simulink model "DYN_03x"  (R2021a)
(part 6 of 9)

C315 = + 1.5*a3*de5*m6*y6*cos(e2)*cos(e3)*sin(e4)*sin(e5)*sin(e6) + 1.5*a3*de6*m6*y6*cos(e5)*cos(e6)*sin(e2)*sin(e3)*sin(e4) + 0.5*d4*de2*m6*x6*cos(e5)*cos(e6)*sin(e2)*sin(e3)*sin(e4) + 0.5*d4*de3*m6*x6*cos(e5)*cos(e6)*sin(e2)*sin(e3)*sin(e4) + 1.5*d4*de5*m6*x6*cos(e2)*cos(e6)*sin(e3)*sin(e4)*sin(e5) + 1.5*d4*de5*m6*x6*cos(e3)*cos(e6)*sin(e2)*sin(e4)*sin(e5) + 1.5*d4*de6*m6*x6*cos(e2)*cos(e5)*sin(e3)*sin(e4)*sin(e6) + 1.5*d4*de6*m6*x6*cos(e3)*cos(e5)*sin(e2)*sin(e4)*sin(e6) - 2.0*I6xx*de5*cos(e4)*cos(e5)*cos(e6)^2*sin(e2)*sin(e3)*sin(e4)*sin(e5) - 2.0*I6xx*de6*cos(e4)*cos(e5)^2*cos(e6)*sin(e2)*sin(e3)*sin(e4)*sin(e6) + 2.0*I6yy*de5*cos(e4)*cos(e5)*cos(e6)^2*sin(e2)*sin(e3)*sin(e4)*sin(e5) + 2.0*I6yy*de6*cos(e4)*cos(e5)^2*cos(e6)*sin(e2)*sin(e3)*sin(e4)*sin(e6) - 4.0*d4*de1*m4*y4*cos(e2)*cos(e3)*sin(e2)*sin(e3)*sin(e4) + 4.0*d4*de1*m5*z5*cos(e2)*cos(e3)*sin(e2)*sin(e3)*sin(e4) - 8.0*de1*m6*x6*z6*cos(e2)^2*cos(e3)^2*cos(e4)*cos(e5)^2*cos(e6) - 4.0*de1*m5*x5*y5*cos(e2)*cos(e3)*cos(e4)*sin(e2)*sin(e3) + 2.0*de1*m6*x6*y6*cos(e2)*cos(e4)*cos(e5)*sin(e2)*sin(e4) + 2.0*de1*m6*x6*y6*cos(e3)*cos(e4)*cos(e5)*sin(e3)*sin(e4) + 2.0*de1*m6*x6*y6*cos(e4)*cos(e5)*cos(e6)*sin(e5)*sin(e6) + 4.0*de1*m4*x4*z4*cos(e2)*cos(e3)*cos(e4)*sin(e2)*sin(e3) + 2.0*de1*m5*x5*z5*cos(e2)*cos(e4)*cos(e5)*sin(e2)*sin(e4) + 2.0*de1*m5*x5*z5*cos(e3)*cos(e4)*cos(e5)*sin(e3)*sin(e4) - 2.0*de1*m6*x6*z6*cos(e2)*cos(e5)*cos(e6)*sin(e2)*sin(e5) - 2.0*de1*m6*x6*z6*cos(e3)*cos(e5)*cos(e6)*sin(e3)*sin(e5) - 4.0*de4*m5*y5*z5*cos(e2)*cos(e3)*cos(e4)*sin(e4)*sin(e5) + 0.5*de2*m6*y6*z6*cos(e4)*cos(e5)*cos(e6)*sin(e2)*sin(e3) + 0.5*de3*m6*y6*z6*cos(e4)*cos(e5)*cos(e6)*sin(e2)*sin(e3) + 1.5*de4*m6*y6*z6*cos(e2)*cos(e5)*cos(e6)*sin(e3)*sin(e4) + 1.5*de4*m6*y6*z6*cos(e3)*cos(e5)*cos(e6)*sin(e2)*sin(e4) - 2.0*de5*m6*y6*z6*cos(e2)*cos(e3)*cos(e4)*sin(e4)*sin(e6) - 1.0*de4*m6*y6*z6*cos(e2)*cos(e3)*cos(e5)*sin(e5)*sin(e6) + 0.5*de5*m6*y6*z6*cos(e2)*cos(e4)*cos(e6)*sin(e3)*sin(e5) + 0.5*de5*m6*y6*z6*cos(e3)*cos(e4)*cos(e6)*sin(e2)*sin(e5) + 1.5*de6*m6*y6*z6*cos(e2)*cos(e4)*cos(e5)*sin(e3)*sin(e6) + 1.5*de6*m6*y6*z6*cos(e3)*cos(e4)*cos(e5)*sin(e2)*sin(e6) + 1.5*a3*de5*m6*x6*cos(e6)*sin(e2)*sin(e3)*sin(e4)*sin(e5) + 1.5*a3*de6*m6*x6*cos(e5)*sin(e2)*sin(e3)*sin(e4)*sin(e6) - 1.0*a2*de1*m6*y6*cos(e2)*sin(e2)*sin(e3)*sin(e5)*sin(e6) - 0.5*d4*de2*m6*y6*cos(e5)*sin(e2)*sin(e3)*sin(e4)*sin(e6) - 0.5*d4*de3*m6*y6*cos(e5)*sin(e2)*sin(e3)*sin(e4)*sin(e6) - 1.5*d4*de5*m6*y6*cos(e2)*sin(e3)*sin(e4)*sin(e5)*sin(e6) - 1.5*d4*de5*m6*y6*cos(e3)*sin(e2)*sin(e4)*sin(e5)*sin(e6) - 0.5*de2*m6*x6^2*cos(e2)*cos(e3)*cos(e5)*cos(e6)^2*sin(e4)*sin(e5) - 1.0*de2*m6*x6^2*cos(e2)*cos(e4)^2*cos(e5)*cos(e6)*sin(e3)*sin(e6) - 1.0*de2*m6*x6^2*cos(e3)*cos(e4)^2*cos(e5)*cos(e6)*sin(e2)*sin(e6) - 0.5*de3*m6*x6^2*cos(e2)*cos(e3)*cos(e5)*cos(e6)^2*sin(e4)*sin(e5) - 1.0*de3*m6*x6^2*cos(e2)*cos(e4)^2*cos(e5)*cos(e6)*sin(e3)*sin(e6) - 1.0*de3*m6*x6^2*cos(e3)*cos(e4)^2*cos(e5)*cos(e6)*sin(e2)*sin(e6) - 1.5*de4*m6*x6^2*cos(e2)*cos(e4)*cos(e5)*cos(e6)^2*sin(e3)*sin(e5) - 1.5*de4*m6*x6^2*cos(e3)*cos(e4)*cos(e5)*cos(e6)^2*sin(e2)*sin(e5) - 2.0*de5*m6*x6^2*cos(e2)*cos(e3)*cos(e4)^2*cos(e6)*sin(e5)*sin(e6) + 0.5*de2*m6*y6^2*cos(e2)*cos(e3)*cos(e5)*cos(e6)^2*sin(e4)*sin(e5) + de2*m6*y6^2*cos(e2)*cos(e4)^2*cos(e5)*cos(e6)*sin(e3)*sin(e6) + de2*m6*y6^2*cos(e3)*cos(e4)^2*cos(e5)*cos(e6)*sin(e2)*sin(e6) + 0.5*de3*m6*y6^2*cos(e2)*cos(e3)*cos(e5)*cos(e6)^2*sin(e4)*sin(e5) + de3*m6*y6^2*cos(e2)*cos(e4)^2*cos(e5)*cos(e6)*sin(e3)*sin(e6) + de3*m6*y6^2*cos(e3)*cos(e4)^2*cos(e5)*cos(e6)*sin(e2)*sin(e6) + 1.5*de4*m6*y6^2*cos(e2)*cos(e4)*cos(e5)*cos(e6)^2*sin(e3)*sin(e5) + 1.5*de4*m6*y6^2*cos(e3)*cos(e4)*cos(e5)*cos(e6)^2*sin(e2)*sin(e5) + 2.0*de5*m6*y6^2*cos(e2)*cos(e3)*cos(e4)^2*cos(e6)*sin(e5)*sin(e6) + 4.0*de5*m5*x5*y5*cos(e2)*cos(e5)*sin(e3)*sin(e4)*sin(e5) + 4.0*de5*m5*x5*y5*cos(e3)*cos(e5)*sin(e2)*sin(e4)*sin(e5) - 4.0*de4*m6*x6*y6*cos(e4)*cos(e5)*sin(e2)*sin(e3)*sin(e4) - 2.0*de6*m6*x6*y6*cos(e2)*cos(e5)*sin(e3)*sin(e4)*sin(e5) - 2.0*de6*m6*x6*y6*cos(e3)*cos(e5)*sin(e2)*sin(e4)*sin(e5) - 3.0*de5*m6*x6*y6*cos(e2)*cos(e6)*sin(e3)*sin(e4)*sin(e6) - 3.0*de5*m6*x6*y6*cos(e3)*cos(e6)*sin(e2)*sin(e4)*sin(e6) - 4.0*de6*m6*x6*y6*cos(e5)*cos(e6)*sin(e2)*sin(e3)*sin(e6) + 8.0*de1*m6*y6*z6*cos(e2)^2*cos(e3)^2*cos(e4)*cos(e5)^2*sin(e6) - 4.0*de4*m5*x5*z5*cos(e4)*cos(e5)*sin(e2)*sin(e3)*sin(e4) + 0.5*de2*m6*x6*z6*cos(e4)*cos(e5)*sin(e2)*sin(e3)*sin(e6) + 0.5*de3*m6*x6*z6*cos(e4)*cos(e5)*sin(e2)*sin(e3)*sin(e6) + 1.5*de4*m6*x6*z6*cos(e2)*cos(e5)*sin(e3)*sin(e4)*sin(e6) + 1.5*de4*m6*x6*z6*cos(e3)*cos(e5)*sin(e2)*sin(e4)*sin(e6) - 2.0*de5*m6*x6*z6*cos(e4)*cos(e6)*sin(e2)*sin(e3)*sin(e4) - 1.0*de4*m6*x6*z6*cos(e5)*cos(e6)*sin(e2)*sin(e3)*sin(e5) + 0.5*de5*m6*x6*z6*cos(e2)*cos(e4)*sin(e3)*sin(e5)*sin(e6) + 0.5*de5*m6*x6*z6*cos(e3)*cos(e4)*sin(e2)*sin(e5)*sin(e6) - 4.0*de1*m4*y4*z4*cos(e2)*cos(e3)*sin(e2)*sin(e3)*sin(e4) - 2.0*de1*m5*y5*z5*cos(e2)*cos(e4)*sin(e2)*sin(e4)*sin(e5) - 2.0*de1*m5*y5*z5*cos(e3)*cos(e4)*sin(e3)*sin(e4)*sin(e5) + 2.0*de1*m6*y6*z6*cos(e2)*cos(e5)*sin(e2)*sin(e5)*sin(e6) + 2.0*de1*m6*y6*z6*cos(e3)*cos(e5)*sin(e3)*sin(e5)*sin(e6) - 1.5*a3*de5*m6*y6*sin(e2)*sin(e3)*sin(e4)*sin(e5)*sin(e6) - 2.0*de1*m6*x6^2*cos(e2)*cos(e3)^2*cos(e4)^2*cos(e5)^2*cos(e6)^2*sin(e2) - 2.0*de1*m6*x6^2*cos(e2)^2*cos(e3)*cos(e4)^2*cos(e5)^2*cos(e6)^2*sin(e3) + 2.0*de1*m6*y6^2*cos(e2)*cos(e3)^2*cos(e4)^2*cos(e5)^2*cos(e6)^2*sin(e2) + 2.0*de1*m6*y6^2*cos(e2)^2*cos(e3)*cos(e4)^2*cos(e5)^2*cos(e6)^2*sin(e3) + 8.0*de1*m6*x6*y6*cos(e2)^2*cos(e3)^2*cos(e6)^2*sin(e4)*sin(e5) + 4.0*de4*m5*y5*z5*cos(e4)*sin(e2)*sin(e3)*sin(e4)*sin(e5) + 2.0*de5*m6*y6*z6*cos(e4)*sin(e2)*sin(e3)*sin(e4)*sin(e6) + de4*m6*y6*z6*cos(e5)*sin(e2)*sin(e3)*sin(e5)*sin(e6) + 0.5*de2*m6*x6^2*cos(e5)*cos(e6)^2*sin(e2)*sin(e3)*sin(e4)*sin(e5) + 0.5*de3*m6*x6^2*cos(e5)*cos(e6)^2*sin(e2)*sin(e3)*sin(e4)*sin(e5) + 2.0*de5*m6*x6^2*cos(e4)^2*cos(e6)*sin(e2)*sin(e3)*sin(e5)*sin(e6) - 0.5*de2*m6*y6^2*cos(e5)*cos(e6)^2*sin(e2)*sin(e3)*sin(e4)*sin(e5) - 0.5*de3*m6*y6^2*cos(e5)*cos(e6)^2*sin(e2)*sin(e3)*sin(e4)*sin(e5) - 2.0*de5*m6*y6^2*cos(e4)^2*cos(e6)*sin(e2)*sin(e3)*sin(e5)*sin(e6) - 4.0*a3*de1*m5*x5*cos(e2)*cos(e3)^2*cos(e4)*cos(e5)*sin(e2) - 4.0*a3*de1*m5*x5*cos(e2)^2*cos(e3)*cos(e4)*cos(e5)*sin(e3) - 1.0*a2*de1*m6*x6*cos(e2)^2*cos(e4)*cos(e5)*cos(e6)*sin(e3) - 2.0*de5*m6*y6*z6*cos(e2)*cos(e3)*cos(e4)^2*cos(e5)*cos(e6) + 4.0*a3*de1*m5*y5*cos(e2)*cos(e3)^2*cos(e4)*sin(e2)*sin(e5) + 4.0*a3*de1*m5*y5*cos(e2)^2*cos(e3)*cos(e4)*sin(e3)*sin(e5) + 4.0*a3*de1*m6*y6*cos(e2)*cos(e3)^2*cos(e6)*sin(e2)*sin(e4) + 4.0*a3*de1*m6*y6*cos(e2)^2*cos(e3)*cos(e6)*sin(e3)*sin(e4) + a2*de1*m6*y6*cos(e2)^2*cos(e4)*cos(e5)*sin(e3)*sin(e6) + 4.0*a3*de1*m6*z6*cos(e2)*cos(e3)^2*cos(e4)*sin(e2)*sin(e5) + 4.0*a3*de1*m6*z6*cos(e2)^2*cos(e3)*cos(e4)*sin(e3)*sin(e5) + 4.0*d4*de1*m6*x6*cos(e2)*cos(e3)^2*cos(e6)*sin(e2)*sin(e5) + 4.0*d4*de1*m6*x6*cos(e2)^2*cos(e3)*cos(e6)*sin(e3)*sin(e5) - 4.0*de4*m5*x5*y5*cos(e2)*cos(e3)*cos(e4)^2*cos(e5)*sin(e5) - 4.0*de5*m5*x5*y5*cos(e2)*cos(e3)*cos(e4)*cos(e5)^2*sin(e4) - 1.0*de2*m6*x6*y6*cos(e2)*cos(e3)*cos(e4)*cos(e6)^2*sin(e5) - 1.0*de3*m6*x6*y6*cos(e2)*cos(e3)*cos(e4)*cos(e6)^2*sin(e5) + 2.0*de6*m6*x6*y6*cos(e2)*cos(e3)*cos(e4)*cos(e5)^2*sin(e4) - 4.0*de4*m6*x6*y6*cos(e2)*cos(e3)*cos(e4)^2*cos(e6)*sin(e6) - 1.0*de5*m6*x6*y6*cos(e2)*cos(e4)*cos(e5)*cos(e6)^2*sin(e3) - 1.0*de5*m6*x6*y6*cos(e3)*cos(e4)*cos(e5)*cos(e6)^2*sin(e2) - 4.0*de6*m6*x6*y6*cos(e2)*cos(e3)*cos(e4)*cos(e6)^2*sin(e4) + de4*m6*x6*y6*cos(e2)*cos(e3)*cos(e5)^2*cos(e6)*sin(e6) - 1.0*de2*m6*x6*z6*cos(e2)*cos(e3)*cos(e5)^2*cos(e6)*sin(e4) - 1.0*de3*m6*x6*z6*cos(e2)*cos(e3)*cos(e5)^2*cos(e6)*sin(e4) - 3.0*de4*m6*x6*z6*cos(e2)*cos(e4)*cos(e5)^2*cos(e6)*sin(e3) - 3.0*de4*m6*x6*z6*cos(e3)*cos(e4)*cos(e5)^2*cos(e6)*sin(e2) - 2.0*de5*m6*x6*z6*cos(e2)*cos(e3)*cos(e4)^2*cos(e5)*sin(e6) - 2.0*de6*m6*x6*z6*cos(e2)*cos(e3)*cos(e4)^2*cos(e6)*sin(e5) + 4.0*a3*de1*m6*x6*cos(e2)*cos(e3)^2*sin(e2)*sin(e4)*sin(e6) + 4.0*a3*de1*m6*x6*cos(e2)^2*cos(e3)*sin(e3)*sin(e4)*sin(e6) - 4.0*d4*de1*m6*y6*cos(e2)*cos(e3)^2*sin(e2)*sin(e5)*sin(e6) - 4.0*d4*de1*m6*y6*cos(e2)^2*cos(e3)*sin(e3)*sin(e5)*sin(e6) + 4.0*de1*m4*x4*y4*cos(e2)*cos(e3)^2*cos(e4)*sin(e2)*sin(e4) + 4.0*de1*m4*x4*y4*cos(e2)^2*cos(e3)*cos(e4)*sin(e3)*sin(e4) + 4.0*de1*m5*x5*y5*cos(e2)*cos(e3)^2*cos(e5)*sin(e2)*sin(e5) - 2.0*de1*m5*x5*y5*cos(e2)*cos(e4)^2*cos(e5)*sin(e2)*sin(e5) + 4.0*de1*m5*x5*y5*cos(e2)^2*cos(e3)*cos(e5)*sin(e3)*sin(e5) - 2.0*de1*m5*x5*y5*cos(e3)*cos(e4)^2*cos(e5)*sin(e3)*sin(e5) - 8.0*de1*m6*x6*y6*cos(e2)*cos(e3)^2*cos(e6)*sin(e2)*sin(e6) - 2.0*de1*m6*x6*y6*cos(e2)*cos(e4)^2*cos(e6)*sin(e2)*sin(e6) - 8.0*de1*m6*x6*y6*cos(e2)^2*cos(e3)*cos(e6)*sin(e3)*sin(e6) - 2.0*de1*m6*x6*y6*cos(e2)*cos(e5)^2*cos(e6)*sin(e2)*sin(e6) - 2.0*de1*m6*x6*y6*cos(e3)*cos(e4)^2*cos(e6)*sin(e3)*sin(e6) - 2.0*de1*m6*x6*y6*cos(e3)*cos(e5)^2*cos(e6)*sin(e3)*sin(e6) + de2*m6*y6*z6*cos(e2)*cos(e3)*cos(e5)^2*sin(e4)*sin(e6) + de2*m6*y6*z6*cos(e2)*cos(e4)^2*cos(e6)*sin(e3)*sin(e5) + de2*m6*y6*z6*cos(e3)*cos(e4)^2*cos(e6)*sin(e2)*sin(e5) + de3*m6*y6*z6*cos(e2)*cos(e3)*cos(e5)^2*sin(e4)*sin(e6) + de3*m6*y6*z6*cos(e2)*cos(e4)^2*cos(e6)*sin(e3)*sin(e5) + de3*m6*y6*z6*cos(e3)*cos(e4)^2*cos(e6)*sin(e2)*sin(e5) + 3.0*de4*m6*y6*z6*cos(e2)*cos(e4)*cos(e5)^2*sin(e3)*sin(e6) + 3.0*de4*m6*y6*z6*cos(e3)*cos(e4)*cos(e5)^2*sin(e2)*sin(e6) + 2.0*de5*m6*y6*z6*cos(e4)^2*cos(e5)*cos(e6)*sin(e2)*sin(e3) + 2.0*de6*m6*y6*z6*cos(e2)*cos(e3)*cos(e4)^2*sin(e5)*sin(e6) + 2.0*de6*m6*y6*z6*cos(e2)*cos(e5)^2*cos(e6)*sin(e3)*sin(e4) + 2.0*de6*m6*y6*z6*cos(e3)*cos(e5)^2*cos(e6)*sin(e2)*sin(e4) - 0.5*de2*m6*x6^2*cos(e2)*cos(e4)*cos(e5)^2*cos(e6)^2*sin(e3)*sin(e4) - 0.5*de2*m6*x6^2*cos(e3)*cos(e4)*cos(e5)^2*cos(e6)^2*sin(e2)*sin(e4) - 0.5*de3*m6*x6^2*cos(e2)*cos(e4)*cos(e5)^2*cos(e6)^2*sin(e3)*sin(e4) - 0.5*de3*m6*x6^2*cos(e3)*cos(e4)*cos(e5)^2*cos(e6)^2*sin(e2)*sin(e4) + 0.5*de2*m6*y6^2*cos(e2)*cos(e4)*cos(e5)^2*cos(e6)^2*sin(e3)*sin(e4) + 0.5*de2*m6*y6^2*cos(e3)*cos(e4)*cos(e5)^2*cos(e6)^2*sin(e2)*sin(e4) + 0.5*de3*m6*y6^2*cos(e2)*cos(e4)*cos(e5)^2*cos(e6)^2*sin(e3)*sin(e4) + 0.5*de3*m6*y6^2*cos(e3)*cos(e4)*cos(e5)^2*cos(e6)^2*sin(e2)*sin(e4) + 4.0*de4*m5*x5*y5*cos(e4)^2*cos(e5)*sin(e2)*sin(e3)*sin(e5) + 4.0*de5*m5*x5*y5*cos(e4)*cos(e5)^2*sin(e2)*sin(e3)*sin(e4) + de2*m6*x6*y6*cos(e4)*cos(e6)^2*sin(e2)*sin(e3)*sin(e5) + de3*m6*x6*y6*cos(e4)*cos(e6)^2*sin(e2)*sin(e3)*sin(e5) + 3.0*de4*m6*x6*y6*cos(e2)*cos(e6)^2*sin(e3)*sin(e4)*sin(e5) + 3.0*de4*m6*x6*y6*cos(e3)*cos(e6)^2*sin(e2)*sin(e4)*sin(e5) - 2.0*de6*m6*x6*y6*cos(e4)*cos(e5)^2*sin(e2)*sin(e3)*sin(e4) + 4.0*de4*m6*x6*y6*cos(e4)^2*cos(e6)*sin(e2)*sin(e3)*sin(e6) + 4.0*de6*m6*x6*y6*cos(e4)*cos(e6)^2*sin(e2)*sin(e3)*sin(e4) - 1.0*de4*m6*x6*y6*cos(e5)^2*cos(e6)*sin(e2)*sin(e3)*sin(e6) + de2*m6*x6*z6*cos(e2)*cos(e4)^2*sin(e3)*sin(e5)*sin(e6) + de2*m6*x6*z6*cos(e3)*cos(e4)^2*sin(e2)*sin(e5)*sin(e6) + de2*m6*x6*z6*cos(e5)^2*cos(e6)*sin(e2)*sin(e3)*sin(e4) + de3*m6*x6*z6*cos(e2)*cos(e4)^2*sin(e3)*sin(e5)*sin(e6) + de3*m6*x6*z6*cos(e3)*cos(e4)^2*sin(e2)*sin(e5)*sin(e6) + de3*m6*x6*z6*cos(e5)^2*cos(e6)*sin(e2)*sin(e3)*sin(e4) + 2.0*de5*m6*x6*z6*cos(e4)^2*cos(e5)*sin(e2)*sin(e3)*sin(e6) + 2.0*de6*m6*x6*z6*cos(e2)*cos(e5)^2*sin(e3)*sin(e4)*sin(e6) + 2.0*de6*m6*x6*z6*cos(e3)*cos(e5)^2*sin(e2)*sin(e4)*sin(e6) + 2.0*de6*m6*x6*z6*cos(e4)^2*cos(e6)*sin(e2)*sin(e3)*sin(e5) + 4.0*I6xx*de4*cos(e2)*cos(e3)*cos(e4)*cos(e5)*cos(e6)*sin(e4)*sin(e6) - 4.0*I6yy*de4*cos(e2)*cos(e3)*cos(e4)*cos(e5)*cos(e6)*sin(e4)*sin(e6) + 4.0*de1*m6*x6^2*cos(e2)^2*cos(e3)^2*cos(e6)*sin(e4)*sin(e5)*sin(e6) - 4.0*de1*m6*y6^2*cos(e2)^2*cos(e3)^2*cos(e6)*sin(e4)*sin(e5)*sin(e6) - 1.0*de2*m6*y6*z6*cos(e5)^2*sin(e2)*sin(e3)*sin(e4)*sin(e6) - 1.0*de3*m6*y6*z6*cos(e5)^2*sin(e2)*sin(e3)*sin(e4)*sin(e6) - 2.0*de6*m6*y6*z6*cos(e4)^2*sin(e2)*sin(e3)*sin(e5)*sin(e6) - 4.0*d4*de1*m6*x6*cos(e2)^2*cos(e3)^2*cos(e4)*cos(e5)*cos(e6) - 4.0*I5xx*de1*cos(e2)*cos(e3)*cos(e4)*cos(e5)*sin(e2)*sin(e3)*sin(e5) + 2.0*I6xx*de1*cos(e2)*cos(e4)*cos(e5)*cos(e6)*sin(e2)*sin(e4)*sin(e6) + 2.0*I6xx*de1*cos(e3)*cos(e4)*cos(e5)*cos(e6)*sin(e3)*sin(e4)*sin(e6) + 4.0*I5yy*de1*cos(e2)*cos(e3)*cos(e4)*cos(e5)*sin(e2)*sin(e3)*sin(e5) - 4.0*I6yy*de1*cos(e2)*cos(e3)*cos(e4)*cos(e5)*sin(e2)*sin(e3)*sin(e5) - 2.0*I6yy*de1*cos(e2)*cos(e4)*cos(e5)*cos(e6)*sin(e2)*sin(e4)*sin(e6) - 2.0*I6yy*de1*cos(e3)*cos(e4)*cos(e5)*cos(e6)*sin(e3)*sin(e4)*sin(e6) + 4.0*I6zz*de1*cos(e2)*cos(e3)*cos(e4)*cos(e5)*sin(e2)*sin(e3)*sin(e5) + 4.0*d4*de1*m6*y6*cos(e2)^2*cos(e3)^2*cos(e4)*cos(e5)*sin(e6) - 4.0*I6xx*de4*cos(e4)*cos(e5)*cos(e6)*sin(e2)*sin(e3)*sin(e4)*sin(e6) - 2.0*I6xx*de6*cos(e2)*cos(e5)*cos(e6)*sin(e3)*sin(e4)*sin(e5)*sin(e6) - 2.0*I6xx*de6*cos(e3)*cos(e5)*cos(e6)*sin(e2)*sin(e4)*sin(e5)*sin(e6) + 4.0*I6yy*de4*cos(e4)*cos(e5)*cos(e6)*sin(e2)*sin(e3)*sin(e4)*sin(e6) + 2.0*I6yy*de6*cos(e2)*cos(e5)*cos(e6)*sin(e3)*sin(e4)*sin(e5)*sin(e6) + 2.0*I6yy*de6*cos(e3)*cos(e5)*cos(e6)*sin(e2)*sin(e4)*sin(e5)*sin(e6) - 2.0*de5*m5*x5^2*cos(e2)*cos(e3)*cos(e4)*cos(e5)*sin(e4)*sin(e5) - 0.5*de2*m6*x6^2*cos(e2)*cos(e3)*cos(e4)*cos(e6)*sin(e5)*sin(e6) - 0.5*de3*m6*x6^2*cos(e2)*cos(e3)*cos(e4)*cos(e6)*sin(e5)*sin(e6) - 0.5*de5*m6*x6^2*cos(e2)*cos(e4)*cos(e5)*cos(e6)*sin(e3)*sin(e6) - 0.5*de5*m6*x6^2*cos(e3)*cos(e4)*cos(e5)*cos(e6)*sin(e2)*sin(e6) - 2.0*de6*m6*x6^2*cos(e2)*cos(e3)*cos(e4)*cos(e6)*sin(e4)*sin(e6) - 2.0*de2*m6*x6*y6*cos(e2)*cos(e4)^2*cos(e5)*cos(e6)^2*sin(e3) - 2.0*de2*m6*x6*y6*cos(e3)*cos(e4)^2*cos(e5)*cos(e6)^2*sin(e2) - 2.0*de3*m6*x6*y6*cos(e2)*cos(e4)^2*cos(e5)*cos(e6)^2*sin(e3) - 2.0*de3*m6*x6*y6*cos(e3)*cos(e4)^2*cos(e5)*cos(e6)^2*sin(e2) - 4.0*de5*m6*x6*y6*cos(e2)*cos(e3)*cos(e4)^2*cos(e6)^2*sin(e5) + 2.0*de5*m5*y5^2*cos(e2)*cos(e3)*cos(e4)*cos(e5)*sin(e4)*sin(e5) + 0.5*de2*m6*y6^2*cos(e2)*cos(e3)*cos(e4)*cos(e6)*sin(e5)*sin(e6) - 2.0*de5*m6*y6^2*cos(e2)*cos(e3)*cos(e4)*cos(e5)*sin(e4)*sin(e5) + 0.5*de3*m6*y6^2*cos(e2)*cos(e3)*cos(e4)*cos(e6)*sin(e5)*sin(e6) + 0.5*de5*m6*y6^2*cos(e2)*cos(e4)*cos(e5)*cos(e6)*sin(e3)*sin(e6) + 0.5*de5*m6*y6^2*cos(e3)*cos(e4)*cos(e5)*cos(e6)*sin(e2)*sin(e6) + 2.0*de6*m6*y6^2*cos(e2)*cos(e3)*cos(e4)*cos(e6)*sin(e4)*sin(e6) + 2.0*de5*m6*z6^2*cos(e2)*cos(e3)*cos(e4)*cos(e5)*sin(e4)*sin(e5) + 4.0*de1*m6*y6*z6*cos(e2)^2*cos(e3)^2*cos(e5)*cos(e6)*sin(e4) - 4.0*de1*m6*x6^2*cos(e2)^2*cos(e3)^2*cos(e4)*cos(e5)*cos(e6)^2*sin(e5) + 4.0*de1*m6*y6^2*cos(e2)^2*cos(e3)^2*cos(e4)*cos(e5)*cos(e6)^2*sin(e5) + 4.0*de1*m6*x6*z6*cos(e2)^2*cos(e3)^2*cos(e5)*sin(e4)*sin(e6) - 1.0*a1*de1*m6*x6*cos(e2)*cos(e3)*cos(e4)*cos(e5)*cos(e6) + 1.5*a3*de4*m6*x6*cos(e2)*cos(e3)*cos(e4)*cos(e5)*cos(e6) + 2.0*de5*m5*x5^2*cos(e4)*cos(e5)*sin(e2)*sin(e3)*sin(e4)*sin(e5) + 0.5*de2*m6*x6^2*cos(e4)*cos(e6)*sin(e2)*sin(e3)*sin(e5)*sin(e6) + 0.5*de3*m6*x6^2*cos(e4)*cos(e6)*sin(e2)*sin(e3)*sin(e5)*sin(e6) + 1.5*de4*m6*x6^2*cos(e2)*cos(e6)*sin(e3)*sin(e4)*sin(e5)*sin(e6) + 1.5*de4*m6*x6^2*cos(e3)*cos(e6)*sin(e2)*sin(e4)*sin(e5)*sin(e6) + 2.0*de6*m6*x6^2*cos(e4)*cos(e6)*sin(e2)*sin(e3)*sin(e4)*sin(e6) + 4.0*de5*m6*x6*y6*cos(e4)^2*cos(e6)^2*sin(e2)*sin(e3)*sin(e5) - 2.0*de5*m5*y5^2*cos(e4)*cos(e5)*sin(e2)*sin(e3)*sin(e4)*sin(e5) - 0.5*de2*m6*y6^2*cos(e4)*cos(e6)*sin(e2)*sin(e3)*sin(e5)*sin(e6) + 2.0*de5*m6*y6^2*cos(e4)*cos(e5)*sin(e2)*sin(e3)*sin(e4)*sin(e5) - 0.5*de3*m6*y6^2*cos(e4)*cos(e6)*sin(e2)*sin(e3)*sin(e5)*sin(e6) - 1.5*de4*m6*y6^2*cos(e2)*cos(e6)*sin(e3)*sin(e4)*sin(e5)*sin(e6) - 1.5*de4*m6*y6^2*cos(e3)*cos(e6)*sin(e2)*sin(e4)*sin(e5)*sin(e6) - 2.0*de6*m6*y6^2*cos(e4)*cos(e6)*sin(e2)*sin(e3)*sin(e4)*sin(e6) - 2.0*de5*m6*z6^2*cos(e4)*cos(e5)*sin(e2)*sin(e3)*sin(e4)*sin(e5) - 2.0*de5*m6*x6^2*cos(e2)*cos(e3)*cos(e4)*cos(e5)*cos(e6)^2*sin(e4)*sin(e5) - 2.0*de6*m6*x6^2*cos(e2)*cos(e3)*cos(e4)*cos(e5)^2*cos(e6)*sin(e4)*sin(e6) + 2.0*de5*m6*y6^2*cos(e2)*cos(e3)*cos(e4)*cos(e5)*cos(e6)^2*sin(e4)*sin(e5) + 2.0*de6*m6*y6^2*cos(e2)*cos(e3)*cos(e4)*cos(e5)^2*cos(e6)*sin(e4)*sin(e6) + de2*m5*x5*y5*cos(e2)*cos(e4)*cos(e5)*sin(e3)*sin(e4)*sin(e5) + de2*m5*x5*y5*cos(e3)*cos(e4)*cos(e5)*sin(e2)*sin(e4)*sin(e5) + de3*m5*x5*y5*cos(e2)*cos(e4)*cos(e5)*sin(e3)*sin(e4)*sin(e5) + de3*m5*x5*y5*cos(e3)*cos(e4)*cos(e5)*sin(e2)*sin(e4)*sin(e5) + de2*m6*x6*y6*cos(e2)*cos(e4)*cos(e6)*sin(e3)*sin(e4)*sin(e6) + de2*m6*x6*y6*cos(e3)*cos(e4)*cos(e6)*sin(e2)*sin(e4)*sin(e6) + de3*m6*x6*y6*cos(e2)*cos(e4)*cos(e6)*sin(e3)*sin(e4)*sin(e6) + de3*m6*x6*y6*cos(e3)*cos(e4)*cos(e6)*sin(e2)*sin(e4)*sin(e6) + 4.0*de6*m6*x6*y6*cos(e2)*cos(e4)*cos(e6)*sin(e3)*sin(e5)*sin(e6) + 4.0*de6*m6*x6*y6*cos(e3)*cos(e4)*cos(e6)*sin(e2)*sin(e5)*sin(e6) + 4.0*de4*m6*x6*z6*cos(e2)*cos(e3)*cos(e4)*sin(e4)*sin(e5)*sin(e6) + 4.0*de5*m6*x6*z6*cos(e2)*cos(e5)*cos(e6)*sin(e3)*sin(e4)*sin(e5) + 4.0*de5*m6*x6*z6*cos(e3)*cos(e5)*cos(e6)*sin(e2)*sin(e4)*sin(e5) + 4.0*de1*m5*y5*z5*cos(e2)*cos(e3)*cos(e5)*sin(e2)*sin(e3)*sin(e4) + 4.0*de1*m6*y6*z6*cos(e2)*cos(e3)*cos(e4)*sin(e2)*sin(e3)*sin(e6) + 2.0*de1*m6*y6*z6*cos(e2)*cos(e4)*cos(e6)*sin(e2)*sin(e4)*sin(e5) + 2.0*de1*m6*y6*z6*cos(e3)*cos(e4)*cos(e6)*sin(e3)*sin(e4)*sin(e5) + 4.0*de1*m6*x6*y6*cos(e2)*cos(e3)*sin(e2)*sin(e3)*sin(e4)*sin(e5) + 4.0*de1*m5*x5*z5*cos(e2)*cos(e3)*sin(e2)*sin(e3)*sin(e4)*sin(e5) + 2.0*de1*m6*x6*z6*cos(e2)*cos(e4)*sin(e2)*sin(e4)*sin(e5)*sin(e6) + 2.0*de1*m6*x6*z6*cos(e3)*cos(e4)*sin(e3)*sin(e4)*sin(e5)*sin(e6) - 4.0*de4*m6*y6*z6*cos(e4)*cos(e6)*sin(e2)*sin(e3)*sin(e4)*sin(e5) - 4.0*de5*m6*y6*z6*cos(e2)*cos(e5)*sin(e3)*sin(e4)*sin(e5)*sin(e6) - 4.0*de5*m6*y6*z6*cos(e3)*cos(e5)*sin(e2)*sin(e4)*sin(e5)*sin(e6) + 2.0*de5*m6*x6^2*cos(e4)*cos(e5)*cos(e6)^2*sin(e2)*sin(e3)*sin(e4)*sin(e5) + 2.0*de6*m6*x6^2*cos(e4)*cos(e5)^2*cos(e6)*sin(e2)*sin(e3)*sin(e4)*sin(e6) - 2.0*de5*m6*y6^2*cos(e4)*cos(e5)*cos(e6)^2*sin(e2)*sin(e3)*sin(e4)*sin(e5) - 2.0*de6*m6*y6^2*cos(e4)*cos(e5)^2*cos(e6)*sin(e2)*sin(e3)*sin(e4)*sin(e6) - 4.0*de4*m6*x6*z6*cos(e4)*sin(e2)*sin(e3)*sin(e4)*sin(e5)*sin(e6) - 4.0*a3*de1*m6*x6*cos(e2)*cos(e3)^2*cos(e4)*cos(e5)*cos(e6)*sin(e2) - 4.0*a3*de1*m6*x6*cos(e2)^2*cos(e3)*cos(e4)*cos(e5)*cos(e6)*sin(e3) + 4.0*a3*de1*m6*y6*cos(e2)*cos(e3)^2*cos(e4)*cos(e5)*sin(e2)*sin(e6) + 4.0*a3*de1*m6*y6*cos(e2)^2*cos(e3)*cos(e4)*cos(e5)*sin(e3)*sin(e6) - 8.0*de4*m6*x6*y6*cos(e2)*cos(e3)*cos(e4)*cos(e5)*cos(e6)^2*sin(e4) - 8.0*de6*m6*x6*y6*cos(e2)*cos(e3)*cos(e4)^2*cos(e5)*cos(e6)*sin(e6) - 4.0*de4*m6*x6*z6*cos(e2)*cos(e3)*cos(e4)^2*cos(e5)*cos(e6)*sin(e5) - 4.0*de5*m6*x6*z6*cos(e2)*cos(e3)*cos(e4)*cos(e5)^2*cos(e6)*sin(e4) + 8.0*de1*m5*x5*y5*cos(e2)*cos(e3)*cos(e4)*cos(e5)^2*sin(e2)*sin(e3) - 4.0*de1*m6*x6*y6*cos(e2)*cos(e3)^2*cos(e4)*cos(e5)*sin(e2)*sin(e4) - 4.0*de1*m6*x6*y6*cos(e2)^2*cos(e3)*cos(e4)*cos(e5)*sin(e3)*sin(e4) - 4.0*de1*m6*x6*y6*cos(e2)*cos(e4)*cos(e5)*cos(e6)^2*sin(e2)*sin(e4) - 4.0*de1*m6*x6*y6*cos(e3)*cos(e4)*cos(e5)*cos(e6)^2*sin(e3)*sin(e4) - 4.0*de1*m6*x6*y6*cos(e2)^2*cos(e4)*cos(e5)*cos(e6)*sin(e5)*sin(e6) - 4.0*de1*m6*x6*y6*cos(e3)^2*cos(e4)*cos(e5)*cos(e6)*sin(e5)*sin(e6) - 4.0*de1*m5*x5*z5*cos(e2)*cos(e3)^2*cos(e4)*cos(e5)*sin(e2)*sin(e4) - 4.0*de1*m5*x5*z5*cos(e2)^2*cos(e3)*cos(e4)*cos(e5)*sin(e3)*sin(e4) + 4.0*de1*m6*x6*z6*cos(e2)*cos(e3)^2*cos(e5)*cos(e6)*sin(e2)*sin(e5) - 2.0*de1*m6*x6*z6*cos(e2)*cos(e4)^2*cos(e5)*cos(e6)*sin(e2)*sin(e5) + 4.0*de1*m6*x6*z6*cos(e2)^2*cos(e3)*cos(e5)*cos(e6)*sin(e3)*sin(e5) - 2.0*de1*m6*x6*z6*cos(e3)*cos(e4)^2*cos(e5)*cos(e6)*sin(e3)*sin(e5) + 4.0*de4*m6*y6*z6*cos(e2)*cos(e3)*cos(e4)^2*cos(e5)*sin(e5)*sin(e6) + 4.0*de5*m6*y6*z6*cos(e2)*cos(e3)*cos(e4)*cos(e5)^2*sin(e4)*sin(e6) + 8.0*de4*m6*x6*y6*cos(e4)*cos(e5)*cos(e6)^2*sin(e2)*sin(e3)*sin(e4) + 4.0*de5*m6*x6*y6*cos(e2)*cos(e5)^2*cos(e6)*sin(e3)*sin(e4)*sin(e6) + 4.0*de5*m6*x6*y6*cos(e3)*cos(e5)^2*cos(e6)*sin(e2)*sin(e4)*sin(e6) + 4.0*de6*m6*x6*y6*cos(e2)*cos(e5)*cos(e6)^2*sin(e3)*sin(e4)*sin(e5) + 4.0*de6*m6*x6*y6*cos(e3)*cos(e5)*cos(e6)^2*sin(e2)*sin(e4)*sin(e5) + 8.0*de6*m6*x6*y6*cos(e4)^2*cos(e5)*cos(e6)*sin(e2)*sin(e3)*sin(e6) + 4.0*de4*m6*x6*z6*cos(e4)^2*cos(e5)*cos(e6)*sin(e2)*sin(e3)*sin(e5) + 4.0*de5*m6*x6*z6*cos(e4)*cos(e5)^2*cos(e6)*sin(e2)*sin(e3)*sin(e4) + 4.0*de1*m5*y5*z5*cos(e2)*cos(e3)^2*cos(e4)*sin(e2)*sin(e4)*sin(e5) + 4.0*de1*m5*y5*z5*cos(e2)^2*cos(e3)*cos(e4)*sin(e3)*sin(e4)*sin(e5) - 4.0*de1*m6*y6*z6*cos(e2)*cos(e3)^2*cos(e5)*sin(e2)*sin(e5)*sin(e6) + 2.0*de1*m6*y6*z6*cos(e2)*cos(e4)^2*cos(e5)*sin(e2)*sin(e5)*sin(e6) - 4.0*de1*m6*y6*z6*cos(e2)^2*cos(e3)*cos(e5)*sin(e3)*sin(e5)*sin(e6) + 2.0*de1*m6*y6*z6*cos(e3)*cos(e4)^2*cos(e5)*sin(e3)*sin(e5)*sin(e6) - 4.0*de4*m6*y6*z6*cos(e4)^2*cos(e5)*sin(e2)*sin(e3)*sin(e5)*sin(e6) - 4.0*de5*m6*y6*z6*cos(e4)*cos(e5)^2*sin(e2)*sin(e3)*sin(e4)*sin(e6) + 4.0*I6xx*de1*cos(e2)*cos(e3)*cos(e6)*sin(e2)*sin(e3)*sin(e4)*sin(e5)*sin(e6) - 4.0*I6yy*de1*cos(e2)*cos(e3)*cos(e6)*sin(e2)*sin(e3)*sin(e4)*sin(e5)*sin(e6) - 4.0*de4*m6*x6^2*cos(e2)*cos(e3)*cos(e4)*cos(e5)*cos(e6)*sin(e4)*sin(e6) - 4.0*de4*m6*x6*y6*cos(e2)*cos(e3)*cos(e4)^2*cos(e5)^2*cos(e6)*sin(e6) - 4.0*de6*m6*x6*y6*cos(e2)*cos(e3)*cos(e4)*cos(e5)^2*cos(e6)^2*sin(e4) + 4.0*de4*m6*y6^2*cos(e2)*cos(e3)*cos(e4)*cos(e5)*cos(e6)*sin(e4)*sin(e6) + 4.0*de1*m5*x5^2*cos(e2)*cos(e3)*cos(e4)*cos(e5)*sin(e2)*sin(e3)*sin(e5) - 2.0*de1*m6*x6^2*cos(e2)*cos(e4)*cos(e5)*cos(e6)*sin(e2)*sin(e4)*sin(e6) - 2.0*de1*m6*x6^2*cos(e3)*cos(e4)*cos(e5)*cos(e6)*sin(e3)*sin(e4)*sin(e6) + 4.0*de1*m5*x5*y5*cos(e2)*cos(e3)^2*cos(e4)^2*cos(e5)*sin(e2)*sin(e5) + 4.0*de1*m5*x5*y5*cos(e2)^2*cos(e3)*cos(e4)^2*cos(e5)*sin(e3)*sin(e5) + 4.0*de1*m6*x6*y6*cos(e2)*cos(e3)^2*cos(e4)^2*cos(e6)*sin(e2)*sin(e6) + 4.0*de1*m6*x6*y6*cos(e2)*cos(e3)^2*cos(e5)^2*cos(e6)*sin(e2)*sin(e6) + 4.0*de1*m6*x6*y6*cos(e2)^2*cos(e3)*cos(e4)^2*cos(e6)*sin(e3)*sin(e6) - 2.0*de1*m6*x6*y6*cos(e2)*cos(e4)^2*cos(e5)^2*cos(e6)*sin(e2)*sin(e6) + 4.0*de1*m6*x6*y6*cos(e2)^2*cos(e3)*cos(e5)^2*cos(e6)*sin(e3)*sin(e6) - 2.0*de1*m6*x6*y6*cos(e3)*cos(e4)^2*cos(e5)^2*cos(e6)*sin(e3)*sin(e6) - 4.0*de1*m5*y5^2*cos(e2)*cos(e3)*cos(e4)*cos(e5)*sin(e2)*sin(e3)*sin(e5) + 4.0*de1*m6*y6^2*cos(e2)*cos(e3)*cos(e4)*cos(e5)*sin(e2)*sin(e3)*sin(e5) + 2.0*de1*m6*y6^2*cos(e2)*cos(e4)*cos(e5)*cos(e6)*sin(e2)*sin(e4)*sin(e6) + 2.0*de1*m6*y6^2*cos(e3)*cos(e4)*cos(e5)*cos(e6)*sin(e3)*sin(e4)*sin(e6) - 4.0*de1*m6*z6^2*cos(e2)*cos(e3)*cos(e4)*cos(e5)*sin(e2)*sin(e3)*sin(e5) + 4.0*de4*m6*x6^2*cos(e4)*cos(e5)*cos(e6)*sin(e2)*sin(e3)*sin(e4)*sin(e6) + 2.0*de6*m6*x6^2*cos(e2)*cos(e5)*cos(e6)*sin(e3)*sin(e4)*sin(e5)*sin(e6) + 2.0*de6*m6*x6^2*cos(e3)*cos(e5)*cos(e6)*sin(e2)*sin(e4)*sin(e5)*sin(e6) + 4.0*de4*m6*x6*y6*cos(e4)^2*cos(e5)^2*cos(e6)*sin(e2)*sin(e3)*sin(e6) + 4.0*de6*m6*x6*y6*cos(e4)*cos(e5)^2*cos(e6)^2*sin(e2)*sin(e3)*sin(e4) - 4.0*de4*m6*y6^2*cos(e4)*cos(e5)*cos(e6)*sin(e2)*sin(e3)*sin(e4)*sin(e6) - 2.0*de6*m6*y6^2*cos(e2)*cos(e5)*cos(e6)*sin(e3)*sin(e4)*sin(e5)*sin(e6) - 2.0*de6*m6*y6^2*cos(e3)*cos(e5)*cos(e6)*sin(e2)*sin(e4)*sin(e5)*sin(e6) - 1.0*a2*de1*m6*x6*cos(e2)*cos(e3)*cos(e4)*cos(e5)*cos(e6)*sin(e2) + a2*de1*m6*y6*cos(e2)*cos(e3)*cos(e4)*cos(e5)*sin(e2)*sin(e6) + 4.0*d4*de1*m5*x5*cos(e2)*cos(e3)*cos(e4)*cos(e5)*sin(e2)*sin(e3) - 4.0*I6xx*de1*cos(e2)*cos(e3)*cos(e4)*cos(e5)*cos(e6)^2*sin(e2)*sin(e3)*sin(e5) - 4.0*I6xx*de1*cos(e2)*cos(e3)^2*cos(e4)*cos(e5)*cos(e6)*sin(e2)*sin(e4)*sin(e6) - 4.0*I6xx*de1*cos(e2)^2*cos(e3)*cos(e4)*cos(e5)*cos(e6)*sin(e3)*sin(e4)*sin(e6) + 4.0*I6yy*de1*cos(e2)*cos(e3)*cos(e4)*cos(e5)*cos(e6)^2*sin(e2)*sin(e3)*sin(e5) + 4.0*I6yy*de1*cos(e2)*cos(e3)^2*cos(e4)*cos(e5)*cos(e6)*sin(e2)*sin(e4)*sin(e6) + 4.0*I6yy*de1*cos(e2)^2*cos(e3)*cos(e4)*cos(e5)*cos(e6)*sin(e3)*sin(e4)*sin(e6) + 4.0*a3*de1*m6*x6*cos(e2)*cos(e3)*cos(e6)*sin(e2)*sin(e3)*sin(e5) - 4.0*d4*de1*m5*y5*cos(e2)*cos(e3)*cos(e4)*sin(e2)*sin(e3)*sin(e5) - 4.0*d4*de1*m6*y6*cos(e2)*cos(e3)*cos(e6)*sin(e2)*sin(e3)*sin(e4) - 4.0*d4*de1*m6*z6*cos(e2)*cos(e3)*cos(e4)*sin(e2)*sin(e3)*sin(e5) - 4.0*de1*m6*x6*z6*cos(e2)*cos(e3)*cos(e4)*cos(e6)*sin(e2)*sin(e3) + 4.0*de4*m6*y6*z6*cos(e2)*cos(e3)*cos(e4)*cos(e6)*sin(e4)*sin(e5) - 4.0*a3*de1*m6*y6*cos(e2)*cos(e3)*sin(e2)*sin(e3)*sin(e5)*sin(e6) - 4.0*d4*de1*m6*x6*cos(e2)*cos(e3)*sin(e2)*sin(e3)*sin(e4)*sin(e6) + 8.0*de1*m6*x6*z6*cos(e2)*cos(e3)*cos(e4)*cos(e5)^2*cos(e6)*sin(e2)*sin(e3) + de2*m6*x6*y6*cos(e2)*cos(e4)*cos(e5)^2*cos(e6)*sin(e3)*sin(e4)*sin(e6) + de2*m6*x6*y6*cos(e3)*cos(e4)*cos(e5)^2*cos(e6)*sin(e2)*sin(e4)*sin(e6) + de3*m6*x6*y6*cos(e2)*cos(e4)*cos(e5)^2*cos(e6)*sin(e3)*sin(e4)*sin(e6) + de3*m6*x6*y6*cos(e3)*cos(e4)*cos(e5)^2*cos(e6)*sin(e2)*sin(e4)*sin(e6) - 8.0*de1*m6*y6*z6*cos(e2)*cos(e3)*cos(e4)*cos(e5)^2*sin(e2)*sin(e3)*sin(e6) - 4.0*de1*m6*y6*z6*cos(e2)*cos(e3)^2*cos(e4)*cos(e6)*sin(e2)*sin(e4)*sin(e5) - 4.0*de1*m6*y6*z6*cos(e2)^2*cos(e3)*cos(e4)*cos(e6)*sin(e3)*sin(e4)*sin(e5) - 8.0*de1*m6*x6*y6*cos(e2)*cos(e3)*cos(e6)^2*sin(e2)*sin(e3)*sin(e4)*sin(e5) - 4.0*de1*m6*x6*z6*cos(e2)*cos(e3)^2*cos(e4)*sin(e2)*sin(e4)*sin(e5)*sin(e6) - 4.0*de1*m6*x6*z6*cos(e2)^2*cos(e3)*cos(e4)*sin(e3)*sin(e4)*sin(e5)*sin(e6) + 8.0*de1*m6*x6*y6*cos(e2)*cos(e3)^2*cos(e4)*cos(e5)*cos(e6)^2*sin(e2)*sin(e4) + 8.0*de1*m6*x6*y6*cos(e2)^2*cos(e3)*cos(e4)*cos(e5)*cos(e6)^2*sin(e3)*sin(e4) + 8.0*de1*m6*x6*y6*cos(e2)^2*cos(e3)^2*cos(e4)*cos(e5)*cos(e6)*sin(e5)*sin(e6) + 4.0*de1*m6*x6*z6*cos(e2)*cos(e3)^2*cos(e4)^2*cos(e5)*cos(e6)*sin(e2)*sin(e5) + 4.0*de1*m6*x6*z6*cos(e2)^2*cos(e3)*cos(e4)^2*cos(e5)*cos(e6)*sin(e3)*sin(e5) - 4.0*de1*m6*y6*z6*cos(e2)*cos(e3)^2*cos(e4)^2*cos(e5)*sin(e2)*sin(e5)*sin(e6) - 4.0*de1*m6*y6*z6*cos(e2)^2*cos(e3)*cos(e4)^2*cos(e5)*sin(e3)*sin(e5)*sin(e6) - 4.0*de1*m6*x6^2*cos(e2)*cos(e3)*cos(e6)*sin(e2)*sin(e3)*sin(e4)*sin(e5)*sin(e6) + 4.0*de1*m6*y6^2*cos(e2)*cos(e3)*cos(e6)*sin(e2)*sin(e3)*sin(e4)*sin(e5)*sin(e6) + 4.0*d4*de1*m6*x6*cos(e2)*cos(e3)*cos(e4)*cos(e5)*cos(e6)*sin(e2)*sin(e3) - 4.0*d4*de1*m6*y6*cos(e2)*cos(e3)*cos(e4)*cos(e5)*sin(e2)*sin(e3)*sin(e6) + 2.0*de6*m6*y6*z6*cos(e2)*cos(e3)*cos(e4)*cos(e5)*cos(e6)*sin(e4)*sin(e5) + de2*m6*x6*y6*cos(e2)*cos(e3)*cos(e5)*cos(e6)*sin(e4)*sin(e5)*sin(e6) + de3*m6*x6*y6*cos(e2)*cos(e3)*cos(e5)*cos(e6)*sin(e4)*sin(e5)*sin(e6) + 3.0*de4*m6*x6*y6*cos(e2)*cos(e4)*cos(e5)*cos(e6)*sin(e3)*sin(e5)*sin(e6) + 3.0*de4*m6*x6*y6*cos(e3)*cos(e4)*cos(e5)*cos(e6)*sin(e2)*sin(e5)*sin(e6) + de2*m6*x6*z6*cos(e2)*cos(e4)*cos(e5)*cos(e6)*sin(e3)*sin(e4)*sin(e5) + de2*m6*x6*z6*cos(e3)*cos(e4)*cos(e5)*cos(e6)*sin(e2)*sin(e4)*sin(e5) + de3*m6*x6*z6*cos(e2)*cos(e4)*cos(e5)*cos(e6)*sin(e3)*sin(e4)*sin(e5) + de3*m6*x6*z6*cos(e3)*cos(e4)*cos(e5)*cos(e6)*sin(e2)*sin(e4)*sin(e5) + 2.0*de6*m6*x6*z6*cos(e2)*cos(e3)*cos(e4)*cos(e5)*sin(e4)*sin(e5)*sin(e6) - 4.0*de1*m6*y6*z6*cos(e2)*cos(e3)*cos(e5)*cos(e6)*sin(e2)*sin(e3)*sin(e4) + 4.0*de1*m6*x6^2*cos(e2)*cos(e3)*cos(e4)*cos(e5)*cos(e6)^2*sin(e2)*sin(e3)*sin(e5) + 4.0*de1*m6*x6^2*cos(e2)*cos(e3)^2*cos(e4)*cos(e5)*cos(e6)*sin(e2)*sin(e4)*sin(e6) + 4.0*de1*m6*x6^2*cos(e2)^2*cos(e3)*cos(e4)*cos(e5)*cos(e6)*sin(e3)*sin(e4)*sin(e6) + 4.0*de1*m6*x6*y6*cos(e2)*cos(e3)^2*cos(e4)^2*cos(e5)^2*cos(e6)*sin(e2)*sin(e6) + 4.0*de1*m6*x6*y6*cos(e2)^2*cos(e3)*cos(e4)^2*cos(e5)^2*cos(e6)*sin(e3)*sin(e6) - 4.0*de1*m6*y6^2*cos(e2)*cos(e3)*cos(e4)*cos(e5)*cos(e6)^2*sin(e2)*sin(e3)*sin(e5) - 4.0*de1*m6*y6^2*cos(e2)*cos(e3)^2*cos(e4)*cos(e5)*cos(e6)*sin(e2)*sin(e4)*sin(e6) - 4.0*de1*m6*y6^2*cos(e2)^2*cos(e3)*cos(e4)*cos(e5)*cos(e6)*sin(e3)*sin(e4)*sin(e6) - 4.0*de1*m6*x6*z6*cos(e2)*cos(e3)*cos(e5)*sin(e2)*sin(e3)*sin(e4)*sin(e6) - 1.0*de2*m6*y6*z6*cos(e2)*cos(e4)*cos(e5)*sin(e3)*sin(e4)*sin(e5)*sin(e6) - 1.0*de2*m6*y6*z6*cos(e3)*cos(e4)*cos(e5)*sin(e2)*sin(e4)*sin(e5)*sin(e6) - 1.0*de3*m6*y6*z6*cos(e2)*cos(e4)*cos(e5)*sin(e3)*sin(e4)*sin(e5)*sin(e6) - 1.0*de3*m6*y6*z6*cos(e3)*cos(e4)*cos(e5)*sin(e2)*sin(e4)*sin(e5)*sin(e6) - 2.0*de6*m6*y6*z6*cos(e4)*cos(e5)*cos(e6)*sin(e2)*sin(e3)*sin(e4)*sin(e5) - 1.0*de2*m6*x6*y6*cos(e5)*cos(e6)*sin(e2)*sin(e3)*sin(e4)*sin(e5)*sin(e6) - 1.0*de3*m6*x6*y6*cos(e5)*cos(e6)*sin(e2)*sin(e3)*sin(e4)*sin(e5)*sin(e6) - 2.0*de6*m6*x6*z6*cos(e4)*cos(e5)*sin(e2)*sin(e3)*sin(e4)*sin(e5)*sin(e6) + 4.0*de5*m6*x6*y6*cos(e2)*cos(e3)*cos(e4)*cos(e5)*cos(e6)*sin(e4)*sin(e5)*sin(e6) - 4.0*de5*m6*x6*y6*cos(e4)*cos(e5)*cos(e6)*sin(e2)*sin(e3)*sin(e4)*sin(e5)*sin(e6) - 8.0*de1*m6*x6*y6*cos(e2)*cos(e3)*cos(e4)*cos(e5)*cos(e6)*sin(e2)*sin(e3)*sin(e5)*sin(e6);
C32 = I4xx*de4*sin(2.0*e4) - 1.0*I5xx*de5*sin(2*e5) - 1.0*I4yy*de4*sin(2*e4) - 1.0*I6yy*de5*sin(2*e5) - 1.0*I5zz*de4*sin(2*e4) - 1.0*I6xx*de4*sin(2*e4) + I5yy*de4*sin(2.0*e4) + I5yy*de5*sin(2.0*e5) + I6zz*de4*sin(2.0*e4) + I6zz*de5*sin(2.0*e5) + 2.0*de4*m4*x4*y4 - 2.0*de5*m5*x5*y5 - 1.0*de4*m4*x4^2*sin(2*e4) - 1.0*de4*m5*y5^2*sin(2*e4) - 1.0*de5*m5*y5^2*sin(2*e5) - 1.0*de4*m6*z6^2*sin(2*e4) - 1.0*de5*m6*z6^2*sin(2*e5) + de4*m6*x6^2*sin(2.0*e4) + de5*m5*x5^2*sin(2.0*e5) + de4*m4*y4^2*sin(2.0*e4) + de5*m6*y6^2*sin(2.0*e5) + de4*m5*z5^2*sin(2.0*e4) - 4.0*de4*m4*x4*y4*cos(e4)^2 + 2.0*de5*m5*x5*y5*cos(e4)^2 + 4.0*de5*m5*x5*y5*cos(e5)^2 + 2.0*de6*m6*x6*y6*cos(e4)^2 - 2.0*de6*m6*x6*y6*cos(e5)^2 - 2.0*I6xx*de6*cos(e4)*cos(e5)*sin(e4) - 2.0*I6xx*de4*cos(e5)*cos(e6)*sin(e6) + 2.0*I6yy*de6*cos(e4)*cos(e5)*sin(e4) + 2.0*I6yy*de4*cos(e5)*cos(e6)*sin(e6) + a2*d4*de2*m4*cos(e3) + a2*d4*de2*m5*cos(e3) - 0.5*a2*d4*de3*m4*cos(e3) + a2*d4*de2*m6*cos(e3) - 0.5*a2*d4*de3*m5*cos(e3) - 0.5*a2*d4*de3*m6*cos(e3) + a2*a3*de2*m4*sin(e3) + a2*a3*de2*m5*sin(e3) - 0.5*a2*a3*de3*m4*sin(e3) + a2*a3*de2*m6*sin(e3) - 0.5*a2*a3*de3*m5*sin(e3) - 0.5*a2*a3*de3*m6*sin(e3) + a2*de2*m3*y3*cos(e3) - 0.5*a2*de3*m3*y3*cos(e3) - 2.0*a3*de4*m4*y4*cos(e4) + a2*de2*m4*z4*cos(e3) - 0.5*a2*de3*m4*z4*cos(e3) + 2.0*a3*de4*m5*z5*cos(e4) + 2.0*d4*de5*m5*x5*cos(e5) + 2.0*I5xx*de4*cos(e4)*cos(e5)^2*sin(e4) + 2.0*I5xx*de5*cos(e4)^2*cos(e5)*sin(e5) + 2.0*I6xx*de4*cos(e4)*cos(e6)^2*sin(e4) - 2.0*I6xx*de5*cos(e5)*cos(e6)^2*sin(e5) + 2.0*I6xx*de6*cos(e4)^2*cos(e6)*sin(e6) - 2.0*I6xx*de6*cos(e5)^2*cos(e6)*sin(e6) - 2.0*I5yy*de4*cos(e4)*cos(e5)^2*sin(e4) + 2.0*I6yy*de4*cos(e4)*cos(e5)^2*sin(e4) - 2.0*I5yy*de5*cos(e4)^2*cos(e5)*sin(e5) - 2.0*I6yy*de4*cos(e4)*cos(e6)^2*sin(e4) + 2.0*I6yy*de5*cos(e4)^2*cos(e5)*sin(e5) + 2.0*I6yy*de5*cos(e5)*cos(e6)^2*sin(e5) - 2.0*I6yy*de6*cos(e4)^2*cos(e6)*sin(e6) + 2.0*I6yy*de6*cos(e5)^2*cos(e6)*sin(e6) - 2.0*I6zz*de4*cos(e4)*cos(e5)^2*sin(e4) - 2.0*I6zz*de5*cos(e4)^2*cos(e5)*sin(e5) + a2*de2*m3*x3*sin(e3) - 0.5*a2*de3*m3*x3*sin(e3) - 2.0*a3*de4*m4*x4*sin(e4) - 2.0*d4*de5*m5*y5*sin(e5) - 2.0*d4*de5*m6*z6*sin(e5) - 2.0*de4*m6*x6*y6*cos(e5) - 2.0*de4*m5*x5*z5*cos(e5) - 2.0*de5*m6*x6*z6*cos(e6) + 2.0*de4*m5*y5*z5*sin(e5) + 2.0*de5*m6*y6*z6*sin(e6) + 4.0*de4*m6*x6*y6*cos(e4)^2*cos(e5) + 4.0*de4*m6*x6*y6*cos(e5)*cos(e6)^2 + 4.0*de4*m5*x5*z5*cos(e4)^2*cos(e5) + 2.0*de5*m6*x6*z6*cos(e4)^2*cos(e6) + 4.0*de5*m6*x6*z6*cos(e5)^2*cos(e6) - 4.0*de4*m5*y5*z5*cos(e4)^2*sin(e5) - 2.0*de5*m6*y6*z6*cos(e4)^2*sin(e6) - 4.0*de5*m6*y6*z6*cos(e5)^2*sin(e6) - 0.5*I4xx*de1*cos(e2)*cos(e4)*sin(e3)*sin(e4) - 0.5*I4xx*de1*cos(e3)*cos(e4)*sin(e2)*sin(e4) + 0.5*I6xx*de1*cos(e2)*cos(e4)*sin(e3)*sin(e4) + 0.5*I6xx*de1*cos(e3)*cos(e4)*sin(e2)*sin(e4) + 0.5*I4yy*de1*cos(e2)*cos(e4)*sin(e3)*sin(e4) + 0.5*I4yy*de1*cos(e3)*cos(e4)*sin(e2)*sin(e4) - 0.5*I5yy*de1*cos(e2)*cos(e4)*sin(e3)*sin(e4) - 0.5*I5yy*de1*cos(e3)*cos(e4)*sin(e2)*sin(e4) + 0.5*I5zz*de1*cos(e2)*cos(e4)*sin(e3)*sin(e4) + 0.5*I5zz*de1*cos(e3)*cos(e4)*sin(e2)*sin(e4) - 0.5*I6zz*de1*cos(e2)*cos(e4)*sin(e3)*sin(e4) - 0.5*I6zz*de1*cos(e3)*cos(e4)*sin(e2)*sin(e4) + 2.0*de6*m6*x6^2*cos(e4)*cos(e5)*sin(e4) + 2.0*de4*m6*x6^2*cos(e5)*cos(e6)*sin(e6) - 4.0*de5*m5*x5*y5*cos(e4)^2*cos(e5)^2 + 2.0*de6*m6*x6*y6*cos(e4)^2*cos(e5)^2 - 4.0*de6*m6*x6*y6*cos(e4)^2*cos(e6)^2 + 4.0*de6*m6*x6*y6*cos(e5)^2*cos(e6)^2 - 2.0*de6*m6*y6^2*cos(e4)*cos(e5)*sin(e4) - 2.0*de4*m6*y6^2*cos(e5)*cos(e6)*sin(e6) - 0.5*a2*de4*m4*y4*cos(e3)*cos(e4) + a2*de2*m5*y5*cos(e3)*cos(e5) - 0.5*a2*de3*m5*y5*cos(e3)*cos(e5) - 2.0*a3*de5*m5*y5*cos(e4)*cos(e5) - 2.0*a3*de4*m6*y6*cos(e4)*cos(e6) + 0.5*a2*de4*m5*z5*cos(e3)*cos(e4) + a2*de2*m6*z6*cos(e3)*cos(e5) - 0.5*a2*de3*m6*z6*cos(e3)*cos(e5) - 2.0*a3*de5*m6*z6*cos(e4)*cos(e5) + 2.0*d4*de5*m6*x6*cos(e5)*cos(e6) + 4.0*I6xx*de4*cos(e4)^2*cos(e5)*cos(e6)*sin(e6) + 4.0*I6xx*de6*cos(e4)*cos(e5)*cos(e6)^2*sin(e4) - 4.0*I6yy*de4*cos(e4)^2*cos(e5)*cos(e6)*sin(e6) - 4.0*I6yy*de6*cos(e4)*cos(e5)*cos(e6)^2*sin(e4) + a2*de2*m4*x4*cos(e4)*sin(e3) - 0.5*a2*de3*m4*x4*cos(e4)*sin(e3) - 0.5*a2*de4*m4*x4*cos(e3)*sin(e4) + a2*de2*m5*x5*cos(e3)*sin(e5) - 0.5*a2*de3*m5*x5*cos(e3)*sin(e5) - 0.5*a2*de5*m5*x5*cos(e5)*sin(e3) - 2.0*a3*de4*m5*x5*cos(e5)*sin(e4) - 2.0*a3*de5*m5*x5*cos(e4)*sin(e5) - 2.0*a3*de4*m6*x6*cos(e4)*sin(e6) - 2.0*a3*de6*m6*x6*cos(e6)*sin(e4) - 2.0*d4*de5*m6*y6*cos(e5)*sin(e6) - 2.0*d4*de6*m6*y6*cos(e6)*sin(e5) - 0.5*de1*m3*y3*z3*cos(e2)*cos(e3) - 1.0*a2*de2*m4*y4*sin(e3)*sin(e4) + 0.5*a2*de3*m4*y4*sin(e3)*sin(e4) + 0.5*a2*de5*m5*y5*sin(e3)*sin(e5) + 2.0*a3*de4*m5*y5*sin(e4)*sin(e5) + 2.0*a3*de6*m6*y6*sin(e4)*sin(e6) + a2*de2*m5*z5*sin(e3)*sin(e4) - 0.5*a2*de3*m5*z5*sin(e3)*sin(e4) + 0.5*a2*de5*m6*z6*sin(e3)*sin(e5) + 2.0*a3*de4*m6*z6*sin(e4)*sin(e5) - 2.0*d4*de6*m6*x6*sin(e5)*sin(e6) - 0.5*de1*m4*x4*y4*cos(e2)*sin(e3) - 0.5*de1*m4*x4*y4*cos(e3)*sin(e2) - 0.5*de1*m3*x3*z3*cos(e2)*sin(e3) - 0.5*de1*m3*x3*z3*cos(e3)*sin(e2) - 2.0*de4*m6*y6*z6*cos(e6)*sin(e5) - 2.0*de4*m5*x5^2*cos(e4)*cos(e5)^2*sin(e4) - 2.0*de5*m5*x5^2*cos(e4)^2*cos(e5)*sin(e5) - 2.0*de4*m6*x6^2*cos(e4)*cos(e6)^2*sin(e4) + 2.0*de5*m6*x6^2*cos(e5)*cos(e6)^2*sin(e5) - 2.0*de6*m6*x6^2*cos(e4)^2*cos(e6)*sin(e6) + 2.0*de6*m6*x6^2*cos(e5)^2*cos(e6)*sin(e6) + 2.0*de4*m5*y5^2*cos(e4)*cos(e5)^2*sin(e4) - 2.0*de4*m6*y6^2*cos(e4)*cos(e5)^2*sin(e4) + 2.0*de5*m5*y5^2*cos(e4)^2*cos(e5)*sin(e5) + 2.0*de4*m6*y6^2*cos(e4)*cos(e6)^2*sin(e4) - 2.0*de5*m6*y6^2*cos(e4)^2*cos(e5)*sin(e5) - 2.0*de5*m6*y6^2*cos(e5)*cos(e6)^2*sin(e5) + 2.0*de6*m6*y6^2*cos(e4)^2*cos(e6)*sin(e6) - 2.0*de6*m6*y6^2*cos(e5)^2*cos(e6)*sin(e6) + 2.0*de4*m6*z6^2*cos(e4)*cos(e5)^2*sin(e4) + 2.0*de5*m6*z6^2*cos(e4)^2*cos(e5)*sin(e5) - 2.0*de4*m6*x6*z6*sin(e5)*sin(e6) + 0.5*de1*m3*y3*z3*sin(e2)*sin(e3) + 2.0*I6xx*de4*cos(e4)*cos(e5)^2*cos(e6)^2*sin(e4) + 2.0*I6xx*de5*cos(e4)^2*cos(e5)*cos(e6)^2*sin(e5) + 2.0*I6xx*de6*cos(e4)^2*cos(e5)^2*cos(e6)*sin(e6) - 2.0*I6yy*de4*cos(e4)*cos(e5)^2*cos(e6)^2*sin(e4) - 2.0*I6yy*de5*cos(e4)^2*cos(e5)*cos(e6)^2*sin(e5) - 2.0*I6yy*de6*cos(e4)^2*cos(e5)^2*cos(e6)*sin(e6) - 0.5*I5xx*de1*cos(e2)*cos(e3)*cos(e5)*sin(e4)*sin(e5) + 0.5*I6xx*de1*cos(e2)*cos(e5)*cos(e6)*sin(e3)*sin(e6) + 0.5*I6xx*de1*cos(e3)*cos(e5)*cos(e6)*sin(e2)*sin(e6) + 0.5*I5yy*de1*cos(e2)*cos(e3)*cos(e5)*sin(e4)*sin(e5) - 0.5*I6yy*de1*cos(e2)*cos(e3)*cos(e5)*sin(e4)*sin(e5) - 0.5*I6yy*de1*cos(e2)*cos(e5)*cos(e6)*sin(e3)*sin(e6) - 0.5*I6yy*de1*cos(e3)*cos(e5)*cos(e6)*sin(e2)*sin(e6) + 0.5*I6zz*de1*cos(e2)*cos(e3)*cos(e5)*sin(e4)*sin(e5) - 2.0*I6xx*de5*cos(e4)*cos(e6)*sin(e4)*sin(e5)*sin(e6) + 2.0*I6yy*de5*cos(e4)*cos(e6)*sin(e4)*sin(e5)*sin(e6) + 0.5*I5xx*de1*cos(e5)*sin(e2)*sin(e3)*sin(e4)*sin(e5) - 0.5*I5yy*de1*cos(e5)*sin(e2)*sin(e3)*sin(e4)*sin(e5) + 0.5*I6yy*de1*cos(e5)*sin(e2)*sin(e3)*sin(e4)*sin(e5) - 0.5*I6zz*de1*cos(e5)*sin(e2)*sin(e3)*sin(e4)*sin(e5) - 8.0*de4*m6*x6*y6*cos(e4)^2*cos(e5)*cos(e6)^2 - 4.0*de5*m6*x6*z6*cos(e4)^2*cos(e5)^2*cos(e6) + 0.5*de1*m4*x4^2*cos(e2)*cos(e4)*sin(e3)*sin(e4) + 0.5*de1*m4*x4^2*cos(e3)*cos(e4)*sin(e2)*sin(e4) - 0.5*de1*m6*x6^2*cos(e2)*cos(e4)*sin(e3)*sin(e4) - 0.5*de1*m6*x6^2*cos(e3)*cos(e4)*sin(e2)*sin(e4) - 0.5*de1*m4*y4^2*cos(e2)*cos(e4)*sin(e3)*sin(e4) - 0.5*de1*m4*y4^2*cos(e3)*cos(e4)*sin(e2)*sin(e4) + 0.5*de1*m5*y5^2*cos(e2)*cos(e4)*sin(e3)*sin(e4) + 0.5*de1*m5*y5^2*cos(e3)*cos(e4)*sin(e2)*sin(e4) - 0.5*de1*m5*z5^2*cos(e2)*cos(e4)*sin(e3)*sin(e4) - 0.5*de1*m5*z5^2*cos(e3)*cos(e4)*sin(e2)*sin(e4) + 0.5*de1*m6*z6^2*cos(e2)*cos(e4)*sin(e3)*sin(e4) + 0.5*de1*m6*z6^2*cos(e3)*cos(e4)*sin(e2)*sin(e4) + 4.0*de5*m6*y6*z6*cos(e4)^2*cos(e5)^2*sin(e6) - 0.5*a2*de5*m5*y5*cos(e3)*cos(e4)*cos(e5) - 0.5*a2*de4*m6*y6*cos(e3)*cos(e4)*cos(e6) - 2.0*a3*de6*m6*y6*cos(e4)*cos(e5)*cos(e6) - 0.5*a2*de5*m6*z6*cos(e3)*cos(e4)*cos(e5) + 0.5*d4*de1*m4*y4*cos(e2)*cos(e3)*cos(e4) - 0.5*d4*de1*m5*z5*cos(e2)*cos(e3)*cos(e4) + a2*de2*m5*x5*cos(e4)*cos(e5)*sin(e3) - 0.5*a2*de3*m5*x5*cos(e4)*cos(e5)*sin(e3) - 0.5*a2*de4*m5*x5*cos(e3)*cos(e5)*sin(e4) - 0.5*a2*de5*m5*x5*cos(e3)*cos(e4)*sin(e5) + a2*de2*m6*x6*cos(e3)*cos(e6)*sin(e5) - 0.5*a2*de3*m6*x6*cos(e3)*cos(e6)*sin(e5) - 0.5*a2*de4*m6*x6*cos(e3)*cos(e4)*sin(e6) - 0.5*a2*de5*m6*x6*cos(e5)*cos(e6)*sin(e3) - 0.5*a2*de6*m6*x6*cos(e3)*cos(e6)*sin(e4) - 2.0*a3*de4*m6*x6*cos(e5)*cos(e6)*sin(e4) - 2.0*a3*de5*m6*x6*cos(e4)*cos(e6)*sin(e5) - 2.0*a3*de6*m6*x6*cos(e4)*cos(e5)*sin(e6) + 0.5*a3*de1*m4*y4*cos(e2)*cos(e4)*sin(e3) + 0.5*a3*de1*m4*y4*cos(e3)*cos(e4)*sin(e2) - 0.5*a3*de1*m5*z5*cos(e2)*cos(e4)*sin(e3) - 0.5*a3*de1*m5*z5*cos(e3)*cos(e4)*sin(e2) + 0.5*d4*de1*m4*x4*cos(e2)*cos(e3)*sin(e4) - 0.5*I5xx*de1*cos(e2)*cos(e4)*cos(e5)^2*sin(e3)*sin(e4) - 0.5*I5xx*de1*cos(e3)*cos(e4)*cos(e5)^2*sin(e2)*sin(e4) - 0.5*I6xx*de1*cos(e2)*cos(e4)*cos(e6)^2*sin(e3)*sin(e4) - 0.5*I6xx*de1*cos(e3)*cos(e4)*cos(e6)^2*sin(e2)*sin(e4) + 0.5*I5yy*de1*cos(e2)*cos(e4)*cos(e5)^2*sin(e3)*sin(e4) + 0.5*I5yy*de1*cos(e3)*cos(e4)*cos(e5)^2*sin(e2)*sin(e4) - 0.5*I6yy*de1*cos(e2)*cos(e4)*cos(e5)^2*sin(e3)*sin(e4) - 0.5*I6yy*de1*cos(e3)*cos(e4)*cos(e5)^2*sin(e2)*sin(e4) + 0.5*I6yy*de1*cos(e2)*cos(e4)*cos(e6)^2*sin(e3)*sin(e4) + 0.5*I6yy*de1*cos(e3)*cos(e4)*cos(e6)^2*sin(e2)*sin(e4) + 0.5*I6zz*de1*cos(e2)*cos(e4)*cos(e5)^2*sin(e3)*sin(e4) + 0.5*I6zz*de1*cos(e3)*cos(e4)*cos(e5)^2*sin(e2)*sin(e4) + 0.5*de1*m4*y4*z4*cos(e2)*cos(e3)*cos(e4) + 0.5*a3*de1*m4*x4*cos(e2)*sin(e3)*sin(e4) + 0.5*a3*de1*m4*x4*cos(e3)*sin(e2)*sin(e4) - 1.0*a2*de2*m5*y5*cos(e4)*sin(e3)*sin(e5) + 0.5*a2*de3*m5*y5*cos(e4)*sin(e3)*sin(e5) + 0.5*a2*de4*m5*y5*cos(e3)*sin(e4)*sin(e5) - 1.0*a2*de2*m6*y6*cos(e6)*sin(e3)*sin(e4) - 1.0*a2*de2*m6*y6*cos(e3)*sin(e5)*sin(e6) + 0.5*a2*de3*m6*y6*cos(e6)*sin(e3)*sin(e4) + 0.5*a2*de3*m6*y6*cos(e3)*sin(e5)*sin(e6) + 0.5*a2*de5*m6*y6*cos(e5)*sin(e3)*sin(e6) + 0.5*a2*de6*m6*y6*cos(e3)*sin(e4)*sin(e6) + 0.5*a2*de6*m6*y6*cos(e6)*sin(e3)*sin(e5) + 2.0*a3*de4*m6*y6*cos(e5)*sin(e4)*sin(e6) + 2.0*a3*de5*m6*y6*cos(e4)*sin(e5)*sin(e6) - 1.0*a2*de2*m6*z6*cos(e4)*sin(e3)*sin(e5) + 0.5*a2*de3*m6*z6*cos(e4)*sin(e3)*sin(e5) + 0.5*a2*de4*m6*z6*cos(e3)*sin(e4)*sin(e5) - 0.5*d4*de1*m4*y4*cos(e4)*sin(e2)*sin(e3) + 0.5*d4*de1*m5*z5*cos(e4)*sin(e2)*sin(e3) - 0.5*de1*m5*x5*y5*cos(e2)*cos(e3)*sin(e4) + 0.5*de1*m6*x6*y6*cos(e2)*cos(e5)*sin(e3) + 0.5*de1*m6*x6*y6*cos(e3)*cos(e5)*sin(e2) + 0.5*de1*m4*x4*z4*cos(e2)*cos(e3)*sin(e4) + 0.5*de1*m5*x5*z5*cos(e2)*cos(e5)*sin(e3) + 0.5*de1*m5*x5*z5*cos(e3)*cos(e5)*sin(e2) - 2.0*de5*m5*y5*z5*cos(e4)*cos(e5)*sin(e4) - 2.0*de6*m6*y6*z6*cos(e5)*cos(e6)*sin(e5) - 1.0*a2*de2*m6*x6*sin(e3)*sin(e4)*sin(e6) + 0.5*a2*de3*m6*x6*sin(e3)*sin(e4)*sin(e6) + 0.5*a2*de6*m6*x6*sin(e3)*sin(e5)*sin(e6) - 0.5*d4*de1*m4*x4*sin(e2)*sin(e3)*sin(e4) - 4.0*de4*m6*x6^2*cos(e4)^2*cos(e5)*cos(e6)*sin(e6) - 4.0*de6*m6*x6^2*cos(e4)*cos(e5)*cos(e6)^2*sin(e4) - 4.0*de6*m6*x6*y6*cos(e4)^2*cos(e5)^2*cos(e6)^2 + 4.0*de4*m6*y6^2*cos(e4)^2*cos(e5)*cos(e6)*sin(e6) + 4.0*de6*m6*y6^2*cos(e4)*cos(e5)*cos(e6)^2*sin(e4) - 2.0*de5*m6*x6*y6*cos(e4)*sin(e4)*sin(e5) - 2.0*de5*m5*x5*z5*cos(e4)*sin(e4)*sin(e5) - 2.0*de6*m6*x6*z6*cos(e5)*sin(e5)*sin(e6) - 0.5*de1*m4*y4*z4*cos(e4)*sin(e2)*sin(e3) - 0.5*de1*m5*y5*z5*cos(e2)*sin(e3)*sin(e5) - 0.5*de1*m5*y5*z5*cos(e3)*sin(e2)*sin(e5) + 0.5*de1*m5*x5*y5*sin(e2)*sin(e3)*sin(e4) - 0.5*de1*m4*x4*z4*sin(e2)*sin(e3)*sin(e4) + de1*m4*x4*y4*cos(e2)*cos(e4)^2*sin(e3) + de1*m4*x4*y4*cos(e3)*cos(e4)^2*sin(e2) + 4.0*de4*m6*y6*z6*cos(e4)^2*cos(e6)*sin(e5) - 2.0*de4*m6*x6^2*cos(e4)*cos(e5)^2*cos(e6)^2*sin(e4) - 2.0*de5*m6*x6^2*cos(e4)^2*cos(e5)*cos(e6)^2*sin(e5) - 2.0*de6*m6*x6^2*cos(e4)^2*cos(e5)^2*cos(e6)*sin(e6) + 2.0*de4*m6*y6^2*cos(e4)*cos(e5)^2*cos(e6)^2*sin(e4) + 2.0*de5*m6*y6^2*cos(e4)^2*cos(e5)*cos(e6)^2*sin(e5) + 2.0*de6*m6*y6^2*cos(e4)^2*cos(e5)^2*cos(e6)*sin(e6) + 4.0*de4*m6*x6*z6*cos(e4)^2*sin(e5)*sin(e6) + 0.5*de1*m5*x5^2*cos(e2)*cos(e3)*cos(e5)*sin(e4)*sin(e5) - 0.5*de1*m6*x6^2*cos(e2)*cos(e5)*cos(e6)*sin(e3)*sin(e6) - 0.5*de1*m6*x6^2*cos(e3)*cos(e5)*cos(e6)*sin(e2)*sin(e6) - 0.5*de1*m5*y5^2*cos(e2)*cos(e3)*cos(e5)*sin(e4)*sin(e5) + 0.5*de1*m6*y6^2*cos(e2)*cos(e3)*cos(e5)*sin(e4)*sin(e5) + 0.5*de1*m6*y6^2*cos(e2)*cos(e5)*cos(e6)*sin(e3)*sin(e6) + 0.5*de1*m6*y6^2*cos(e3)*cos(e5)*cos(e6)*sin(e2)*sin(e6) - 0.5*de1*m6*z6^2*cos(e2)*cos(e3)*cos(e5)*sin(e4)*sin(e5) + 2.0*de5*m6*x6^2*cos(e4)*cos(e6)*sin(e4)*sin(e5)*sin(e6) - 2.0*de5*m6*y6^2*cos(e4)*cos(e6)*sin(e4)*sin(e5)*sin(e6) - 0.5*a2*de6*m6*y6*cos(e3)*cos(e4)*cos(e5)*cos(e6) + 0.5*d4*de1*m6*y6*cos(e2)*cos(e3)*cos(e4)*cos(e6) - 0.5*de1*m5*x5^2*cos(e5)*sin(e2)*sin(e3)*sin(e4)*sin(e5) + 0.5*de1*m5*y5^2*cos(e5)*sin(e2)*sin(e3)*sin(e4)*sin(e5) - 0.5*de1*m6*y6^2*cos(e5)*sin(e2)*sin(e3)*sin(e4)*sin(e5) + 0.5*de1*m6*z6^2*cos(e5)*sin(e2)*sin(e3)*sin(e4)*sin(e5) + a2*de2*m6*x6*cos(e4)*cos(e5)*cos(e6)*sin(e3) - 0.5*a2*de3*m6*x6*cos(e4)*cos(e5)*cos(e6)*sin(e3) - 0.5*a2*de4*m6*x6*cos(e3)*cos(e5)*cos(e6)*sin(e4) - 0.5*a2*de5*m6*x6*cos(e3)*cos(e4)*cos(e6)*sin(e5) - 0.5*a2*de6*m6*x6*cos(e3)*cos(e4)*cos(e5)*sin(e6) + 0.5*a3*de1*m6*y6*cos(e2)*cos(e4)*cos(e6)*sin(e3) + 0.5*a3*de1*m6*y6*cos(e3)*cos(e4)*cos(e6)*sin(e2) + 0.5*d4*de1*m5*x5*cos(e2)*cos(e3)*cos(e5)*sin(e4) + 0.5*d4*de1*m6*x6*cos(e2)*cos(e3)*cos(e4)*sin(e6) - 0.5*I6xx*de1*cos(e2)*cos(e3)*cos(e5)*cos(e6)^2*sin(e4)*sin(e5) - 1.0*I6xx*de1*cos(e2)*cos(e4)^2*cos(e5)*cos(e6)*sin(e3)*sin(e6) - 1.0*I6xx*de1*cos(e3)*cos(e4)^2*cos(e5)*cos(e6)*sin(e2)*sin(e6) + 0.5*I6yy*de1*cos(e2)*cos(e3)*cos(e5)*cos(e6)^2*sin(e4)*sin(e5) + I6yy*de1*cos(e2)*cos(e4)^2*cos(e5)*cos(e6)*sin(e3)*sin(e6) + I6yy*de1*cos(e3)*cos(e4)^2*cos(e5)*cos(e6)*sin(e2)*sin(e6) - 0.5*de1*m5*y5*z5*cos(e2)*cos(e3)*cos(e4)*cos(e5) + 0.5*a3*de1*m5*x5*cos(e2)*cos(e5)*sin(e3)*sin(e4) + 0.5*a3*de1*m5*x5*cos(e3)*cos(e5)*sin(e2)*sin(e4) + 0.5*a3*de1*m6*x6*cos(e2)*cos(e4)*sin(e3)*sin(e6) + 0.5*a3*de1*m6*x6*cos(e3)*cos(e4)*sin(e2)*sin(e6) - 1.0*a2*de2*m6*y6*cos(e4)*cos(e5)*sin(e3)*sin(e6) + 0.5*a2*de3*m6*y6*cos(e4)*cos(e5)*sin(e3)*sin(e6) + 0.5*a2*de4*m6*y6*cos(e3)*cos(e5)*sin(e4)*sin(e6) + 0.5*a2*de5*m6*y6*cos(e3)*cos(e4)*sin(e5)*sin(e6) - 0.5*d4*de1*m5*y5*cos(e2)*cos(e3)*sin(e4)*sin(e5) - 0.5*d4*de1*m6*y6*cos(e4)*cos(e6)*sin(e2)*sin(e3) - 0.5*d4*de1*m6*z6*cos(e2)*cos(e3)*sin(e4)*sin(e5) - 0.5*de1*m6*x6*y6*cos(e2)*cos(e3)*cos(e4)*sin(e5) - 0.5*de1*m5*x5*z5*cos(e2)*cos(e3)*cos(e4)*sin(e5) - 0.5*de1*m6*x6*z6*cos(e2)*cos(e3)*cos(e6)*sin(e4) + 2.0*de5*m6*y6*z6*cos(e4)*cos(e5)*cos(e6)*sin(e4) - 0.5*a3*de1*m5*y5*cos(e2)*sin(e3)*sin(e4)*sin(e5) - 0.5*a3*de1*m5*y5*cos(e3)*sin(e2)*sin(e4)*sin(e5) - 0.5*a3*de1*m6*z6*cos(e2)*sin(e3)*sin(e4)*sin(e5) - 0.5*a3*de1*m6*z6*cos(e3)*sin(e2)*sin(e4)*sin(e5) - 0.5*d4*de1*m5*x5*cos(e5)*sin(e2)*sin(e3)*sin(e4) - 0.5*d4*de1*m6*x6*cos(e4)*sin(e2)*sin(e3)*sin(e6) + 0.5*I6xx*de1*cos(e5)*cos(e6)^2*sin(e2)*sin(e3)*sin(e4)*sin(e5) - 0.5*I6yy*de1*cos(e5)*cos(e6)^2*sin(e2)*sin(e3)*sin(e4)*sin(e5) + 4.0*de4*m5*x5*y5*cos(e4)*cos(e5)*sin(e4)*sin(e5) + 4.0*de4*m6*x6*y6*cos(e4)*cos(e6)*sin(e4)*sin(e6) - 4.0*de5*m6*x6*y6*cos(e5)*cos(e6)*sin(e5)*sin(e6) + 2.0*de5*m6*x6*z6*cos(e4)*cos(e5)*sin(e4)*sin(e6) + 2.0*de6*m6*x6*z6*cos(e4)*cos(e6)*sin(e4)*sin(e5) + 0.5*de1*m5*y5*z5*cos(e4)*cos(e5)*sin(e2)*sin(e3) + 0.5*de1*m6*y6*z6*cos(e2)*cos(e3)*sin(e4)*sin(e6) + 0.5*de1*m6*y6*z6*cos(e2)*cos(e6)*sin(e3)*sin(e5) + 0.5*de1*m6*y6*z6*cos(e3)*cos(e6)*sin(e2)*sin(e5) + 0.5*d4*de1*m5*y5*sin(e2)*sin(e3)*sin(e4)*sin(e5) + 0.5*d4*de1*m6*z6*sin(e2)*sin(e3)*sin(e4)*sin(e5) + 0.5*de1*m5*x5^2*cos(e2)*cos(e4)*cos(e5)^2*sin(e3)*sin(e4) + 0.5*de1*m5*x5^2*cos(e3)*cos(e4)*cos(e5)^2*sin(e2)*sin(e4) + 0.5*de1*m6*x6^2*cos(e2)*cos(e4)*cos(e6)^2*sin(e3)*sin(e4) + 0.5*de1*m6*x6^2*cos(e3)*cos(e4)*cos(e6)^2*sin(e2)*sin(e4) - 0.5*de1*m5*y5^2*cos(e2)*cos(e4)*cos(e5)^2*sin(e3)*sin(e4) - 0.5*de1*m5*y5^2*cos(e3)*cos(e4)*cos(e5)^2*sin(e2)*sin(e4) + 0.5*de1*m6*y6^2*cos(e2)*cos(e4)*cos(e5)^2*sin(e3)*sin(e4) + 0.5*de1*m6*y6^2*cos(e3)*cos(e4)*cos(e5)^2*sin(e2)*sin(e4) - 0.5*de1*m6*y6^2*cos(e2)*cos(e4)*cos(e6)^2*sin(e3)*sin(e4) - 0.5*de1*m6*y6^2*cos(e3)*cos(e4)*cos(e6)^2*sin(e2)*sin(e4) + 0.5*de1*m6*x6*y6*cos(e4)*sin(e2)*sin(e3)*sin(e5) - 0.5*de1*m6*z6^2*cos(e2)*cos(e4)*cos(e5)^2*sin(e3)*sin(e4) - 0.5*de1*m6*z6^2*cos(e3)*cos(e4)*cos(e5)^2*sin(e2)*sin(e4) + 0.5*de1*m5*x5*z5*cos(e4)*sin(e2)*sin(e3)*sin(e5) + 0.5*de1*m6*x6*z6*cos(e6)*sin(e2)*sin(e3)*sin(e4) + 0.5*de1*m6*x6*z6*cos(e2)*sin(e3)*sin(e5)*sin(e6) + 0.5*de1*m6*x6*z6*cos(e3)*sin(e2)*sin(e5)*sin(e6) - 2.0*de6*m6*y6*z6*cos(e4)*sin(e4)*sin(e5)*sin(e6) - 0.5*de1*m6*y6*z6*sin(e2)*sin(e3)*sin(e4)*sin(e6) - 0.5*I6xx*de1*cos(e2)*cos(e4)*cos(e5)^2*cos(e6)^2*sin(e3)*sin(e4) - 0.5*I6xx*de1*cos(e3)*cos(e4)*cos(e5)^2*cos(e6)^2*sin(e2)*sin(e4) + 0.5*I6yy*de1*cos(e2)*cos(e4)*cos(e5)^2*cos(e6)^2*sin(e3)*sin(e4) + 0.5*I6yy*de1*cos(e3)*cos(e4)*cos(e5)^2*cos(e6)^2*sin(e2)*sin(e4) + de1*m5*x5*y5*cos(e2)*cos(e3)*cos(e5)^2*sin(e4) - 1.0*de1*m6*x6*y6*cos(e2)*cos(e4)^2*cos(e5)*sin(e3) - 1.0*de1*m6*x6*y6*cos(e3)*cos(e4)^2*cos(e5)*sin(e2) - 1.0*de1*m6*x6*y6*cos(e2)*cos(e5)*cos(e6)^2*sin(e3) - 1.0*de1*m6*x6*y6*cos(e3)*cos(e5)*cos(e6)^2*sin(e2) - 1.0*de1*m5*x5*z5*cos(e2)*cos(e4)^2*cos(e5)*sin(e3) - 1.0*de1*m5*x5*z5*cos(e3)*cos(e4)^2*cos(e5)*sin(e2) + 2.0*de6*m6*y6*z6*cos(e4)^2*cos(e5)*cos(e6)*sin(e5) + 4.0*de5*m6*x6*y6*cos(e4)*cos(e6)^2*sin(e4)*sin(e5) + 2.0*de6*m6*x6*z6*cos(e4)^2*cos(e5)*sin(e5)*sin(e6) + de1*m5*y5*z5*cos(e2)*cos(e4)^2*sin(e3)*sin(e5) + de1*m5*y5*z5*cos(e3)*cos(e4)^2*sin(e2)*sin(e5) - 1.0*de1*m5*x5*y5*cos(e5)^2*sin(e2)*sin(e3)*sin(e4) - 0.5*I6xx*de1*cos(e2)*cos(e3)*cos(e4)*cos(e6)*sin(e5)*sin(e6) + 0.5*I6yy*de1*cos(e2)*cos(e3)*cos(e4)*cos(e6)*sin(e5)*sin(e6) + 0.5*I6xx*de1*cos(e4)*cos(e6)*sin(e2)*sin(e3)*sin(e5)*sin(e6) - 0.5*I6yy*de1*cos(e4)*cos(e6)*sin(e2)*sin(e3)*sin(e5)*sin(e6) + 0.5*d4*de1*m6*x6*cos(e2)*cos(e3)*cos(e5)*cos(e6)*sin(e4) + 0.5*de1*m6*y6*z6*cos(e2)*cos(e3)*cos(e4)*cos(e5)*cos(e6) + 0.5*a3*de1*m6*x6*cos(e2)*cos(e5)*cos(e6)*sin(e3)*sin(e4) + 0.5*a3*de1*m6*x6*cos(e3)*cos(e5)*cos(e6)*sin(e2)*sin(e4) - 0.5*d4*de1*m6*y6*cos(e2)*cos(e3)*cos(e5)*sin(e4)*sin(e6) + 0.5*de1*m6*x6*z6*cos(e2)*cos(e3)*cos(e4)*cos(e5)*sin(e6) - 0.5*a3*de1*m6*y6*cos(e2)*cos(e5)*sin(e3)*sin(e4)*sin(e6) - 0.5*a3*de1*m6*y6*cos(e3)*cos(e5)*sin(e2)*sin(e4)*sin(e6) - 0.5*d4*de1*m6*x6*cos(e5)*cos(e6)*sin(e2)*sin(e3)*sin(e4) + 8.0*de6*m6*x6*y6*cos(e4)*cos(e5)*cos(e6)*sin(e4)*sin(e6) + 4.0*de4*m6*x6*z6*cos(e4)*cos(e5)*cos(e6)*sin(e4)*sin(e5) - 0.5*de1*m6*y6*z6*cos(e4)*cos(e5)*cos(e6)*sin(e2)*sin(e3) + 0.5*d4*de1*m6*y6*cos(e5)*sin(e2)*sin(e3)*sin(e4)*sin(e6) + 0.5*de1*m6*x6^2*cos(e2)*cos(e3)*cos(e5)*cos(e6)^2*sin(e4)*sin(e5) + de1*m6*x6^2*cos(e2)*cos(e4)^2*cos(e5)*cos(e6)*sin(e3)*sin(e6) + de1*m6*x6^2*cos(e3)*cos(e4)^2*cos(e5)*cos(e6)*sin(e2)*sin(e6) - 0.5*de1*m6*y6^2*cos(e2)*cos(e3)*cos(e5)*cos(e6)^2*sin(e4)*sin(e5) - 1.0*de1*m6*y6^2*cos(e2)*cos(e4)^2*cos(e5)*cos(e6)*sin(e3)*sin(e6) - 1.0*de1*m6*y6^2*cos(e3)*cos(e4)^2*cos(e5)*cos(e6)*sin(e2)*sin(e6) - 0.5*de1*m6*x6*z6*cos(e4)*cos(e5)*sin(e2)*sin(e3)*sin(e6) - 4.0*de4*m6*y6*z6*cos(e4)*cos(e5)*sin(e4)*sin(e5)*sin(e6) - 0.5*de1*m6*x6^2*cos(e5)*cos(e6)^2*sin(e2)*sin(e3)*sin(e4)*sin(e5) + 0.5*de1*m6*y6^2*cos(e5)*cos(e6)^2*sin(e2)*sin(e3)*sin(e4)*sin(e5) + de1*m6*x6*y6*cos(e2)*cos(e3)*cos(e4)*cos(e6)^2*sin(e5) + de1*m6*x6*z6*cos(e2)*cos(e3)*cos(e5)^2*cos(e6)*sin(e4) + 4.0*de4*m6*x6*y6*cos(e4)*cos(e5)^2*cos(e6)*sin(e4)*sin(e6) + 4.0*de5*m6*x6*y6*cos(e4)^2*cos(e5)*cos(e6)*sin(e5)*sin(e6) - 1.0*de1*m6*y6*z6*cos(e2)*cos(e3)*cos(e5)^2*sin(e4)*sin(e6) - 1.0*de1*m6*y6*z6*cos(e2)*cos(e4)^2*cos(e6)*sin(e3)*sin(e5) - 1.0*de1*m6*y6*z6*cos(e3)*cos(e4)^2*cos(e6)*sin(e2)*sin(e5) + 0.5*de1*m6*x6^2*cos(e2)*cos(e4)*cos(e5)^2*cos(e6)^2*sin(e3)*sin(e4) + 0.5*de1*m6*x6^2*cos(e3)*cos(e4)*cos(e5)^2*cos(e6)^2*sin(e2)*sin(e4) - 0.5*de1*m6*y6^2*cos(e2)*cos(e4)*cos(e5)^2*cos(e6)^2*sin(e3)*sin(e4) - 0.5*de1*m6*y6^2*cos(e3)*cos(e4)*cos(e5)^2*cos(e6)^2*sin(e2)*sin(e4) - 1.0*de1*m6*x6*y6*cos(e4)*cos(e6)^2*sin(e2)*sin(e3)*sin(e5) - 1.0*de1*m6*x6*z6*cos(e2)*cos(e4)^2*sin(e3)*sin(e5)*sin(e6) - 1.0*de1*m6*x6*z6*cos(e3)*cos(e4)^2*sin(e2)*sin(e5)*sin(e6) - 1.0*de1*m6*x6*z6*cos(e5)^2*cos(e6)*sin(e2)*sin(e3)*sin(e4) + de1*m6*y6*z6*cos(e5)^2*sin(e2)*sin(e3)*sin(e4)*sin(e6) + 0.5*de1*m6*x6^2*cos(e2)*cos(e3)*cos(e4)*cos(e6)*sin(e5)*sin(e6) + 2.0*de1*m6*x6*y6*cos(e2)*cos(e4)^2*cos(e5)*cos(e6)^2*sin(e3) + 2.0*de1*m6*x6*y6*cos(e3)*cos(e4)^2*cos(e5)*cos(e6)^2*sin(e2) - 0.5*de1*m6*y6^2*cos(e2)*cos(e3)*cos(e4)*cos(e6)*sin(e5)*sin(e6) - 0.5*de1*m6*x6^2*cos(e4)*cos(e6)*sin(e2)*sin(e3)*sin(e5)*sin(e6) + 0.5*de1*m6*y6^2*cos(e4)*cos(e6)*sin(e2)*sin(e3)*sin(e5)*sin(e6) - 1.0*de1*m5*x5*y5*cos(e2)*cos(e4)*cos(e5)*sin(e3)*sin(e4)*sin(e5) - 1.0*de1*m5*x5*y5*cos(e3)*cos(e4)*cos(e5)*sin(e2)*sin(e4)*sin(e5) - 1.0*de1*m6*x6*y6*cos(e2)*cos(e4)*cos(e6)*sin(e3)*sin(e4)*sin(e6) - 1.0*de1*m6*x6*y6*cos(e3)*cos(e4)*cos(e6)*sin(e2)*sin(e4)*sin(e6) - 1.0*de1*m6*x6*y6*cos(e2)*cos(e4)*cos(e5)^2*cos(e6)*sin(e3)*sin(e4)*sin(e6) - 1.0*de1*m6*x6*y6*cos(e3)*cos(e4)*cos(e5)^2*cos(e6)*sin(e2)*sin(e4)*sin(e6) - 1.0*de1*m6*x6*y6*cos(e2)*cos(e3)*cos(e5)*cos(e6)*sin(e4)*sin(e5)*sin(e6) - 1.0*de1*m6*x6*z6*cos(e2)*cos(e4)*cos(e5)*cos(e6)*sin(e3)*sin(e4)*sin(e5) - 1.0*de1*m6*x6*z6*cos(e3)*cos(e4)*cos(e5)*cos(e6)*sin(e2)*sin(e4)*sin(e5) + de1*m6*y6*z6*cos(e2)*cos(e4)*cos(e5)*sin(e3)*sin(e4)*sin(e5)*sin(e6) + de1*m6*y6*z6*cos(e3)*cos(e4)*cos(e5)*sin(e2)*sin(e4)*sin(e5)*sin(e6) + de1*m6*x6*y6*cos(e5)*cos(e6)*sin(e2)*sin(e3)*sin(e4)*sin(e5)*sin(e6);
C33 = I4xx*de4*sin(2.0*e4) - 1.0*I5xx*de5*sin(2*e5) - 1.0*I4yy*de4*sin(2*e4) - 1.0*I6yy*de5*sin(2*e5) - 1.0*I5zz*de4*sin(2*e4) - 1.0*I6xx*de4*sin(2*e4) + I5yy*de4*sin(2.0*e4) + I5yy*de5*sin(2.0*e5) + I6zz*de4*sin(2.0*e4) + I6zz*de5*sin(2.0*e5) + 2.0*de4*m4*x4*y4 - 2.0*de5*m5*x5*y5 - 1.0*de4*m4*x4^2*sin(2*e4) - 1.0*de4*m5*y5^2*sin(2*e4) - 1.0*de5*m5*y5^2*sin(2*e5) - 1.0*de4*m6*z6^2*sin(2*e4) - 1.0*de5*m6*z6^2*sin(2*e5) + de4*m6*x6^2*sin(2.0*e4) + de5*m5*x5^2*sin(2.0*e5) + de4*m4*y4^2*sin(2.0*e4) + de5*m6*y6^2*sin(2.0*e5) + de4*m5*z5^2*sin(2.0*e4) - 4.0*de4*m4*x4*y4*cos(e4)^2 + 2.0*de5*m5*x5*y5*cos(e4)^2 + 4.0*de5*m5*x5*y5*cos(e5)^2 + 2.0*de6*m6*x6*y6*cos(e4)^2 - 2.0*de6*m6*x6*y6*cos(e5)^2 - 2.0*I6xx*de6*cos(e4)*cos(e5)*sin(e4) - 2.0*I6xx*de4*cos(e5)*cos(e6)*sin(e6) + 2.0*I6yy*de6*cos(e4)*cos(e5)*sin(e4) + 2.0*I6yy*de4*cos(e5)*cos(e6)*sin(e6) + 0.5*a2*d4*de2*m4*cos(e3) + 0.5*a2*d4*de2*m5*cos(e3) + 0.5*a2*d4*de2*m6*cos(e3) + 0.5*a2*a3*de2*m4*sin(e3) + 0.5*a2*a3*de2*m5*sin(e3) + 0.5*a2*a3*de2*m6*sin(e3) + 0.5*a2*de2*m3*y3*cos(e3) - 2.0*a3*de4*m4*y4*cos(e4) + 0.5*a2*de2*m4*z4*cos(e3) + 2.0*a3*de4*m5*z5*cos(e4) + 2.0*d4*de5*m5*x5*cos(e5) + 2.0*I5xx*de4*cos(e4)*cos(e5)^2*sin(e4) + 2.0*I5xx*de5*cos(e4)^2*cos(e5)*sin(e5) + 2.0*I6xx*de4*cos(e4)*cos(e6)^2*sin(e4) - 2.0*I6xx*de5*cos(e5)*cos(e6)^2*sin(e5) + 2.0*I6xx*de6*cos(e4)^2*cos(e6)*sin(e6) - 2.0*I6xx*de6*cos(e5)^2*cos(e6)*sin(e6) - 2.0*I5yy*de4*cos(e4)*cos(e5)^2*sin(e4) + 2.0*I6yy*de4*cos(e4)*cos(e5)^2*sin(e4) - 2.0*I5yy*de5*cos(e4)^2*cos(e5)*sin(e5) - 2.0*I6yy*de4*cos(e4)*cos(e6)^2*sin(e4) + 2.0*I6yy*de5*cos(e4)^2*cos(e5)*sin(e5) + 2.0*I6yy*de5*cos(e5)*cos(e6)^2*sin(e5) - 2.0*I6yy*de6*cos(e4)^2*cos(e6)*sin(e6) + 2.0*I6yy*de6*cos(e5)^2*cos(e6)*sin(e6) - 2.0*I6zz*de4*cos(e4)*cos(e5)^2*sin(e4) - 2.0*I6zz*de5*cos(e4)^2*cos(e5)*sin(e5) + 0.5*a2*de2*m3*x3*sin(e3) - 2.0*a3*de4*m4*x4*sin(e4) - 2.0*d4*de5*m5*y5*sin(e5) - 2.0*d4*de5*m6*z6*sin(e5) - 2.0*de4*m6*x6*y6*cos(e5) - 2.0*de4*m5*x5*z5*cos(e5) - 2.0*de5*m6*x6*z6*cos(e6) + 2.0*de4*m5*y5*z5*sin(e5) + 2.0*de5*m6*y6*z6*sin(e6) + 4.0*de4*m6*x6*y6*cos(e4)^2*cos(e5) + 4.0*de4*m6*x6*y6*cos(e5)*cos(e6)^2 + 4.0*de4*m5*x5*z5*cos(e4)^2*cos(e5) + 2.0*de5*m6*x6*z6*cos(e4)^2*cos(e6) + 4.0*de5*m6*x6*z6*cos(e5)^2*cos(e6) - 4.0*de4*m5*y5*z5*cos(e4)^2*sin(e5) - 2.0*de5*m6*y6*z6*cos(e4)^2*sin(e6) - 4.0*de5*m6*y6*z6*cos(e5)^2*sin(e6) - 0.5*I4xx*de1*cos(e2)*cos(e4)*sin(e3)*sin(e4) - 0.5*I4xx*de1*cos(e3)*cos(e4)*sin(e2)*sin(e4) + 0.5*I6xx*de1*cos(e2)*cos(e4)*sin(e3)*sin(e4) + 0.5*I6xx*de1*cos(e3)*cos(e4)*sin(e2)*sin(e4) + 0.5*I4yy*de1*cos(e2)*cos(e4)*sin(e3)*sin(e4) + 0.5*I4yy*de1*cos(e3)*cos(e4)*sin(e2)*sin(e4) - 0.5*I5yy*de1*cos(e2)*cos(e4)*sin(e3)*sin(e4) - 0.5*I5yy*de1*cos(e3)*cos(e4)*sin(e2)*sin(e4) + 0.5*I5zz*de1*cos(e2)*cos(e4)*sin(e3)*sin(e4) + 0.5*I5zz*de1*cos(e3)*cos(e4)*sin(e2)*sin(e4) - 0.5*I6zz*de1*cos(e2)*cos(e4)*sin(e3)*sin(e4) - 0.5*I6zz*de1*cos(e3)*cos(e4)*sin(e2)*sin(e4) + 2.0*de6*m6*x6^2*cos(e4)*cos(e5)*sin(e4) + 2.0*de4*m6*x6^2*cos(e5)*cos(e6)*sin(e6) - 4.0*de5*m5*x5*y5*cos(e4)^2*cos(e5)^2 + 2.0*de6*m6*x6*y6*cos(e4)^2*cos(e5)^2 - 4.0*de6*m6*x6*y6*cos(e4)^2*cos(e6)^2 + 4.0*de6*m6*x6*y6*cos(e5)^2*cos(e6)^2 - 2.0*de6*m6*y6^2*cos(e4)*cos(e5)*sin(e4) - 2.0*de4*m6*y6^2*cos(e5)*cos(e6)*sin(e6) + 0.5*a2*de2*m5*y5*cos(e3)*cos(e5) - 2.0*a3*de5*m5*y5*cos(e4)*cos(e5) - 2.0*a3*de4*m6*y6*cos(e4)*cos(e6) + 0.5*a2*de2*m6*z6*cos(e3)*cos(e5) - 2.0*a3*de5*m6*z6*cos(e4)*cos(e5) + 2.0*d4*de5*m6*x6*cos(e5)*cos(e6) + 4.0*I6xx*de4*cos(e4)^2*cos(e5)*cos(e6)*sin(e6) + 4.0*I6xx*de6*cos(e4)*cos(e5)*cos(e6)^2*sin(e4) - 4.0*I6yy*de4*cos(e4)^2*cos(e5)*cos(e6)*sin(e6) - 4.0*I6yy*de6*cos(e4)*cos(e5)*cos(e6)^2*sin(e4) + 0.5*a2*de2*m4*x4*cos(e4)*sin(e3) + 0.5*a2*de2*m5*x5*cos(e3)*sin(e5) - 2.0*a3*de4*m5*x5*cos(e5)*sin(e4) - 2.0*a3*de5*m5*x5*cos(e4)*sin(e5) - 2.0*a3*de4*m6*x6*cos(e4)*sin(e6) - 2.0*a3*de6*m6*x6*cos(e6)*sin(e4) - 2.0*d4*de5*m6*y6*cos(e5)*sin(e6) - 2.0*d4*de6*m6*y6*cos(e6)*sin(e5) - 0.5*de1*m3*y3*z3*cos(e2)*cos(e3) - 0.5*a2*de2*m4*y4*sin(e3)*sin(e4) + 2.0*a3*de4*m5*y5*sin(e4)*sin(e5) + 2.0*a3*de6*m6*y6*sin(e4)*sin(e6) + 0.5*a2*de2*m5*z5*sin(e3)*sin(e4) + 2.0*a3*de4*m6*z6*sin(e4)*sin(e5) - 2.0*d4*de6*m6*x6*sin(e5)*sin(e6) - 0.5*de1*m4*x4*y4*cos(e2)*sin(e3) - 0.5*de1*m4*x4*y4*cos(e3)*sin(e2) - 0.5*de1*m3*x3*z3*cos(e2)*sin(e3) - 0.5*de1*m3*x3*z3*cos(e3)*sin(e2) - 2.0*de4*m6*y6*z6*cos(e6)*sin(e5) - 2.0*de4*m5*x5^2*cos(e4)*cos(e5)^2*sin(e4) - 2.0*de5*m5*x5^2*cos(e4)^2*cos(e5)*sin(e5) - 2.0*de4*m6*x6^2*cos(e4)*cos(e6)^2*sin(e4) + 2.0*de5*m6*x6^2*cos(e5)*cos(e6)^2*sin(e5) - 2.0*de6*m6*x6^2*cos(e4)^2*cos(e6)*sin(e6) + 2.0*de6*m6*x6^2*cos(e5)^2*cos(e6)*sin(e6) + 2.0*de4*m5*y5^2*cos(e4)*cos(e5)^2*sin(e4) - 2.0*de4*m6*y6^2*cos(e4)*cos(e5)^2*sin(e4) + 2.0*de5*m5*y5^2*cos(e4)^2*cos(e5)*sin(e5) + 2.0*de4*m6*y6^2*cos(e4)*cos(e6)^2*sin(e4) - 2.0*de5*m6*y6^2*cos(e4)^2*cos(e5)*sin(e5) - 2.0*de5*m6*y6^2*cos(e5)*cos(e6)^2*sin(e5) + 2.0*de6*m6*y6^2*cos(e4)^2*cos(e6)*sin(e6) - 2.0*de6*m6*y6^2*cos(e5)^2*cos(e6)*sin(e6) + 2.0*de4*m6*z6^2*cos(e4)*cos(e5)^2*sin(e4) + 2.0*de5*m6*z6^2*cos(e4)^2*cos(e5)*sin(e5) - 2.0*de4*m6*x6*z6*sin(e5)*sin(e6) + 0.5*de1*m3*y3*z3*sin(e2)*sin(e3) + 2.0*I6xx*de4*cos(e4)*cos(e5)^2*cos(e6)^2*sin(e4) + 2.0*I6xx*de5*cos(e4)^2*cos(e5)*cos(e6)^2*sin(e5) + 2.0*I6xx*de6*cos(e4)^2*cos(e5)^2*cos(e6)*sin(e6) - 2.0*I6yy*de4*cos(e4)*cos(e5)^2*cos(e6)^2*sin(e4) - 2.0*I6yy*de5*cos(e4)^2*cos(e5)*cos(e6)^2*sin(e5) - 2.0*I6yy*de6*cos(e4)^2*cos(e5)^2*cos(e6)*sin(e6) - 0.5*I5xx*de1*cos(e2)*cos(e3)*cos(e5)*sin(e4)*sin(e5) + 0.5*I6xx*de1*cos(e2)*cos(e5)*cos(e6)*sin(e3)*sin(e6) + 0.5*I6xx*de1*cos(e3)*cos(e5)*cos(e6)*sin(e2)*sin(e6) + 0.5*I5yy*de1*cos(e2)*cos(e3)*cos(e5)*sin(e4)*sin(e5) - 0.5*I6yy*de1*cos(e2)*cos(e3)*cos(e5)*sin(e4)*sin(e5) - 0.5*I6yy*de1*cos(e2)*cos(e5)*cos(e6)*sin(e3)*sin(e6) - 0.5*I6yy*de1*cos(e3)*cos(e5)*cos(e6)*sin(e2)*sin(e6) + 0.5*I6zz*de1*cos(e2)*cos(e3)*cos(e5)*sin(e4)*sin(e5) - 2.0*I6xx*de5*cos(e4)*cos(e6)*sin(e4)*sin(e5)*sin(e6) + 2.0*I6yy*de5*cos(e4)*cos(e6)*sin(e4)*sin(e5)*sin(e6) + 0.5*I5xx*de1*cos(e5)*sin(e2)*sin(e3)*sin(e4)*sin(e5) - 0.5*I5yy*de1*cos(e5)*sin(e2)*sin(e3)*sin(e4)*sin(e5) + 0.5*I6yy*de1*cos(e5)*sin(e2)*sin(e3)*sin(e4)*sin(e5) - 0.5*I6zz*de1*cos(e5)*sin(e2)*sin(e3)*sin(e4)*sin(e5) - 8.0*de4*m6*x6*y6*cos(e4)^2*cos(e5)*cos(e6)^2 - 4.0*de5*m6*x6*z6*cos(e4)^2*cos(e5)^2*cos(e6) + 0.5*de1*m4*x4^2*cos(e2)*cos(e4)*sin(e3)*sin(e4) + 0.5*de1*m4*x4^2*cos(e3)*cos(e4)*sin(e2)*sin(e4) - 0.5*de1*m6*x6^2*cos(e2)*cos(e4)*sin(e3)*sin(e4) - 0.5*de1*m6*x6^2*cos(e3)*cos(e4)*sin(e2)*sin(e4) - 0.5*de1*m4*y4^2*cos(e2)*cos(e4)*sin(e3)*sin(e4) - 0.5*de1*m4*y4^2*cos(e3)*cos(e4)*sin(e2)*sin(e4) + 0.5*de1*m5*y5^2*cos(e2)*cos(e4)*sin(e3)*sin(e4) + 0.5*de1*m5*y5^2*cos(e3)*cos(e4)*sin(e2)*sin(e4) - 0.5*de1*m5*z5^2*cos(e2)*cos(e4)*sin(e3)*sin(e4) - 0.5*de1*m5*z5^2*cos(e3)*cos(e4)*sin(e2)*sin(e4) + 0.5*de1*m6*z6^2*cos(e2)*cos(e4)*sin(e3)*sin(e4) + 0.5*de1*m6*z6^2*cos(e3)*cos(e4)*sin(e2)*sin(e4) + 4.0*de5*m6*y6*z6*cos(e4)^2*cos(e5)^2*sin(e6) - 2.0*a3*de6*m6*y6*cos(e4)*cos(e5)*cos(e6) + 0.5*d4*de1*m4*y4*cos(e2)*cos(e3)*cos(e4) - 0.5*d4*de1*m5*z5*cos(e2)*cos(e3)*cos(e4) + 0.5*a2*de2*m5*x5*cos(e4)*cos(e5)*sin(e3) + 0.5*a2*de2*m6*x6*cos(e3)*cos(e6)*sin(e5) - 2.0*a3*de4*m6*x6*cos(e5)*cos(e6)*sin(e4) - 2.0*a3*de5*m6*x6*cos(e4)*cos(e6)*sin(e5) - 2.0*a3*de6*m6*x6*cos(e4)*cos(e5)*sin(e6) + 0.5*a3*de1*m4*y4*cos(e2)*cos(e4)*sin(e3) + 0.5*a3*de1*m4*y4*cos(e3)*cos(e4)*sin(e2) - 0.5*a3*de1*m5*z5*cos(e2)*cos(e4)*sin(e3) - 0.5*a3*de1*m5*z5*cos(e3)*cos(e4)*sin(e2) + 0.5*d4*de1*m4*x4*cos(e2)*cos(e3)*sin(e4) - 0.5*I5xx*de1*cos(e2)*cos(e4)*cos(e5)^2*sin(e3)*sin(e4) - 0.5*I5xx*de1*cos(e3)*cos(e4)*cos(e5)^2*sin(e2)*sin(e4) - 0.5*I6xx*de1*cos(e2)*cos(e4)*cos(e6)^2*sin(e3)*sin(e4) - 0.5*I6xx*de1*cos(e3)*cos(e4)*cos(e6)^2*sin(e2)*sin(e4) + 0.5*I5yy*de1*cos(e2)*cos(e4)*cos(e5)^2*sin(e3)*sin(e4) + 0.5*I5yy*de1*cos(e3)*cos(e4)*cos(e5)^2*sin(e2)*sin(e4) - 0.5*I6yy*de1*cos(e2)*cos(e4)*cos(e5)^2*sin(e3)*sin(e4) - 0.5*I6yy*de1*cos(e3)*cos(e4)*cos(e5)^2*sin(e2)*sin(e4) + 0.5*I6yy*de1*cos(e2)*cos(e4)*cos(e6)^2*sin(e3)*sin(e4) + 0.5*I6yy*de1*cos(e3)*cos(e4)*cos(e6)^2*sin(e2)*sin(e4) + 0.5*I6zz*de1*cos(e2)*cos(e4)*cos(e5)^2*sin(e3)*sin(e4) + 0.5*I6zz*de1*cos(e3)*cos(e4)*cos(e5)^2*sin(e2)*sin(e4) + 0.5*de1*m4*y4*z4*cos(e2)*cos(e3)*cos(e4) + 0.5*a3*de1*m4*x4*cos(e2)*sin(e3)*sin(e4) + 0.5*a3*de1*m4*x4*cos(e3)*sin(e2)*sin(e4) - 0.5*a2*de2*m5*y5*cos(e4)*sin(e3)*sin(e5) - 0.5*a2*de2*m6*y6*cos(e6)*sin(e3)*sin(e4) - 0.5*a2*de2*m6*y6*cos(e3)*sin(e5)*sin(e6) + 2.0*a3*de4*m6*y6*cos(e5)*sin(e4)*sin(e6) + 2.0*a3*de5*m6*y6*cos(e4)*sin(e5)*sin(e6) - 0.5*a2*de2*m6*z6*cos(e4)*sin(e3)*sin(e5) - 0.5*d4*de1*m4*y4*cos(e4)*sin(e2)*sin(e3) + 0.5*d4*de1*m5*z5*cos(e4)*sin(e2)*sin(e3) - 0.5*de1*m5*x5*y5*cos(e2)*cos(e3)*sin(e4) + 0.5*de1*m6*x6*y6*cos(e2)*cos(e5)*sin(e3) + 0.5*de1*m6*x6*y6*cos(e3)*cos(e5)*sin(e2) + 0.5*de1*m4*x4*z4*cos(e2)*cos(e3)*sin(e4) + 0.5*de1*m5*x5*z5*cos(e2)*cos(e5)*sin(e3) + 0.5*de1*m5*x5*z5*cos(e3)*cos(e5)*sin(e2) - 2.0*de5*m5*y5*z5*cos(e4)*cos(e5)*sin(e4) - 2.0*de6*m6*y6*z6*cos(e5)*cos(e6)*sin(e5) - 0.5*a2*de2*m6*x6*sin(e3)*sin(e4)*sin(e6) - 0.5*d4*de1*m4*x4*sin(e2)*sin(e3)*sin(e4) - 4.0*de4*m6*x6^2*cos(e4)^2*cos(e5)*cos(e6)*sin(e6) - 4.0*de6*m6*x6^2*cos(e4)*cos(e5)*cos(e6)^2*sin(e4) - 4.0*de6*m6*x6*y6*cos(e4)^2*cos(e5)^2*cos(e6)^2 + 4.0*de4*m6*y6^2*cos(e4)^2*cos(e5)*cos(e6)*sin(e6) + 4.0*de6*m6*y6^2*cos(e4)*cos(e5)*cos(e6)^2*sin(e4) - 2.0*de5*m6*x6*y6*cos(e4)*sin(e4)*sin(e5) - 2.0*de5*m5*x5*z5*cos(e4)*sin(e4)*sin(e5) - 2.0*de6*m6*x6*z6*cos(e5)*sin(e5)*sin(e6) - 0.5*de1*m4*y4*z4*cos(e4)*sin(e2)*sin(e3) - 0.5*de1*m5*y5*z5*cos(e2)*sin(e3)*sin(e5) - 0.5*de1*m5*y5*z5*cos(e3)*sin(e2)*sin(e5) + 0.5*de1*m5*x5*y5*sin(e2)*sin(e3)*sin(e4) - 0.5*de1*m4*x4*z4*sin(e2)*sin(e3)*sin(e4) + de1*m4*x4*y4*cos(e2)*cos(e4)^2*sin(e3) + de1*m4*x4*y4*cos(e3)*cos(e4)^2*sin(e2) + 4.0*de4*m6*y6*z6*cos(e4)^2*cos(e6)*sin(e5) - 2.0*de4*m6*x6^2*cos(e4)*cos(e5)^2*cos(e6)^2*sin(e4) - 2.0*de5*m6*x6^2*cos(e4)^2*cos(e5)*cos(e6)^2*sin(e5) - 2.0*de6*m6*x6^2*cos(e4)^2*cos(e5)^2*cos(e6)*sin(e6) + 2.0*de4*m6*y6^2*cos(e4)*cos(e5)^2*cos(e6)^2*sin(e4) + 2.0*de5*m6*y6^2*cos(e4)^2*cos(e5)*cos(e6)^2*sin(e5) + 2.0*de6*m6*y6^2*cos(e4)^2*cos(e5)^2*cos(e6)*sin(e6) + 4.0*de4*m6*x6*z6*cos(e4)^2*sin(e5)*sin(e6) + 0.5*de1*m5*x5^2*cos(e2)*cos(e3)*cos(e5)*sin(e4)*sin(e5) - 0.5*de1*m6*x6^2*cos(e2)*cos(e5)*cos(e6)*sin(e3)*sin(e6) - 0.5*de1*m6*x6^2*cos(e3)*cos(e5)*cos(e6)*sin(e2)*sin(e6) - 0.5*de1*m5*y5^2*cos(e2)*cos(e3)*cos(e5)*sin(e4)*sin(e5) + 0.5*de1*m6*y6^2*cos(e2)*cos(e3)*cos(e5)*sin(e4)*sin(e5) + 0.5*de1*m6*y6^2*cos(e2)*cos(e5)*cos(e6)*sin(e3)*sin(e6) + 0.5*de1*m6*y6^2*cos(e3)*cos(e5)*cos(e6)*sin(e2)*sin(e6) - 0.5*de1*m6*z6^2*cos(e2)*cos(e3)*cos(e5)*sin(e4)*sin(e5) + 2.0*de5*m6*x6^2*cos(e4)*cos(e6)*sin(e4)*sin(e5)*sin(e6) - 2.0*de5*m6*y6^2*cos(e4)*cos(e6)*sin(e4)*sin(e5)*sin(e6) + 0.5*d4*de1*m6*y6*cos(e2)*cos(e3)*cos(e4)*cos(e6) - 0.5*de1*m5*x5^2*cos(e5)*sin(e2)*sin(e3)*sin(e4)*sin(e5) + 0.5*de1*m5*y5^2*cos(e5)*sin(e2)*sin(e3)*sin(e4)*sin(e5) - 0.5*de1*m6*y6^2*cos(e5)*sin(e2)*sin(e3)*sin(e4)*sin(e5) + 0.5*de1*m6*z6^2*cos(e5)*sin(e2)*sin(e3)*sin(e4)*sin(e5) + 0.5*a2*de2*m6*x6*cos(e4)*cos(e5)*cos(e6)*sin(e3) + 0.5*a3*de1*m6*y6*cos(e2)*cos(e4)*cos(e6)*sin(e3) + 0.5*a3*de1*m6*y6*cos(e3)*cos(e4)*cos(e6)*sin(e2) + 0.5*d4*de1*m5*x5*cos(e2)*cos(e3)*cos(e5)*sin(e4) + 0.5*d4*de1*m6*x6*cos(e2)*cos(e3)*cos(e4)*sin(e6) - 0.5*I6xx*de1*cos(e2)*cos(e3)*cos(e5)*cos(e6)^2*sin(e4)*sin(e5) - 1.0*I6xx*de1*cos(e2)*cos(e4)^2*cos(e5)*cos(e6)*sin(e3)*sin(e6) - 1.0*I6xx*de1*cos(e3)*cos(e4)^2*cos(e5)*cos(e6)*sin(e2)*sin(e6) + 0.5*I6yy*de1*cos(e2)*cos(e3)*cos(e5)*cos(e6)^2*sin(e4)*sin(e5) + I6yy*de1*cos(e2)*cos(e4)^2*cos(e5)*cos(e6)*sin(e3)*sin(e6) + I6yy*de1*cos(e3)*cos(e4)^2*cos(e5)*cos(e6)*sin(e2)*sin(e6) - 0.5*de1*m5*y5*z5*cos(e2)*cos(e3)*cos(e4)*cos(e5) + 0.5*a3*de1*m5*x5*cos(e2)*cos(e5)*sin(e3)*sin(e4) + 0.5*a3*de1*m5*x5*cos(e3)*cos(e5)*sin(e2)*sin(e4) + 0.5*a3*de1*m6*x6*cos(e2)*cos(e4)*sin(e3)*sin(e6) + 0.5*a3*de1*m6*x6*cos(e3)*cos(e4)*sin(e2)*sin(e6) - 0.5*a2*de2*m6*y6*cos(e4)*cos(e5)*sin(e3)*sin(e6) - 0.5*d4*de1*m5*y5*cos(e2)*cos(e3)*sin(e4)*sin(e5) - 0.5*d4*de1*m6*y6*cos(e4)*cos(e6)*sin(e2)*sin(e3) - 0.5*d4*de1*m6*z6*cos(e2)*cos(e3)*sin(e4)*sin(e5) - 0.5*de1*m6*x6*y6*cos(e2)*cos(e3)*cos(e4)*sin(e5) - 0.5*de1*m5*x5*z5*cos(e2)*cos(e3)*cos(e4)*sin(e5) - 0.5*de1*m6*x6*z6*cos(e2)*cos(e3)*cos(e6)*sin(e4) + 2.0*de5*m6*y6*z6*cos(e4)*cos(e5)*cos(e6)*sin(e4) - 0.5*a3*de1*m5*y5*cos(e2)*sin(e3)*sin(e4)*sin(e5) - 0.5*a3*de1*m5*y5*cos(e3)*sin(e2)*sin(e4)*sin(e5) - 0.5*a3*de1*m6*z6*cos(e2)*sin(e3)*sin(e4)*sin(e5) - 0.5*a3*de1*m6*z6*cos(e3)*sin(e2)*sin(e4)*sin(e5) - 0.5*d4*de1*m5*x5*cos(e5)*sin(e2)*sin(e3)*sin(e4) - 0.5*d4*de1*m6*x6*cos(e4)*sin(e2)*sin(e3)*sin(e6) + 0.5*I6xx*de1*cos(e5)*cos(e6)^2*sin(e2)*sin(e3)*sin(e4)*sin(e5) - 0.5*I6yy*de1*cos(e5)*cos(e6)^2*sin(e2)*sin(e3)*sin(e4)*sin(e5) + 4.0*de4*m5*x5*y5*cos(e4)*cos(e5)*sin(e4)*sin(e5) + 4.0*de4*m6*x6*y6*cos(e4)*cos(e6)*sin(e4)*sin(e6) - 4.0*de5*m6*x6*y6*cos(e5)*cos(e6)*sin(e5)*sin(e6) + 2.0*de5*m6*x6*z6*cos(e4)*cos(e5)*sin(e4)*sin(e6) + 2.0*de6*m6*x6*z6*cos(e4)*cos(e6)*sin(e4)*sin(e5) + 0.5*de1*m5*y5*z5*cos(e4)*cos(e5)*sin(e2)*sin(e3) + 0.5*de1*m6*y6*z6*cos(e2)*cos(e3)*sin(e4)*sin(e6) + 0.5*de1*m6*y6*z6*cos(e2)*cos(e6)*sin(e3)*sin(e5) + 0.5*de1*m6*y6*z6*cos(e3)*cos(e6)*sin(e2)*sin(e5) + 0.5*d4*de1*m5*y5*sin(e2)*sin(e3)*sin(e4)*sin(e5) + 0.5*d4*de1*m6*z6*sin(e2)*sin(e3)*sin(e4)*sin(e5) + 0.5*de1*m5*x5^2*cos(e2)*cos(e4)*cos(e5)^2*sin(e3)*sin(e4) + 0.5*de1*m5*x5^2*cos(e3)*cos(e4)*cos(e5)^2*sin(e2)*sin(e4) + 0.5*de1*m6*x6^2*cos(e2)*cos(e4)*cos(e6)^2*sin(e3)*sin(e4) + 0.5*de1*m6*x6^2*cos(e3)*cos(e4)*cos(e6)^2*sin(e2)*sin(e4) - 0.5*de1*m5*y5^2*cos(e2)*cos(e4)*cos(e5)^2*sin(e3)*sin(e4) - 0.5*de1*m5*y5^2*cos(e3)*cos(e4)*cos(e5)^2*sin(e2)*sin(e4) + 0.5*de1*m6*y6^2*cos(e2)*cos(e4)*cos(e5)^2*sin(e3)*sin(e4) + 0.5*de1*m6*y6^2*cos(e3)*cos(e4)*cos(e5)^2*sin(e2)*sin(e4) - 0.5*de1*m6*y6^2*cos(e2)*cos(e4)*cos(e6)^2*sin(e3)*sin(e4) - 0.5*de1*m6*y6^2*cos(e3)*cos(e4)*cos(e6)^2*sin(e2)*sin(e4) + 0.5*de1*m6*x6*y6*cos(e4)*sin(e2)*sin(e3)*sin(e5) - 0.5*de1*m6*z6^2*cos(e2)*cos(e4)*cos(e5)^2*sin(e3)*sin(e4) - 0.5*de1*m6*z6^2*cos(e3)*cos(e4)*cos(e5)^2*sin(e2)*sin(e4) + 0.5*de1*m5*x5*z5*cos(e4)*sin(e2)*sin(e3)*sin(e5) + 0.5*de1*m6*x6*z6*cos(e6)*sin(e2)*sin(e3)*sin(e4) + 0.5*de1*m6*x6*z6*cos(e2)*sin(e3)*sin(e5)*sin(e6) + 0.5*de1*m6*x6*z6*cos(e3)*sin(e2)*sin(e5)*sin(e6) - 2.0*de6*m6*y6*z6*cos(e4)*sin(e4)*sin(e5)*sin(e6) - 0.5*de1*m6*y6*z6*sin(e2)*sin(e3)*sin(e4)*sin(e6) - 0.5*I6xx*de1*cos(e2)*cos(e4)*cos(e5)^2*cos(e6)^2*sin(e3)*sin(e4) - 0.5*I6xx*de1*cos(e3)*cos(e4)*cos(e5)^2*cos(e6)^2*sin(e2)*sin(e4) + 0.5*I6yy*de1*cos(e2)*cos(e4)*cos(e5)^2*cos(e6)^2*sin(e3)*sin(e4) + 0.5*I6yy*de1*cos(e3)*cos(e4)*cos(e5)^2*cos(e6)^2*sin(e2)*sin(e4) + de1*m5*x5*y5*cos(e2)*cos(e3)*cos(e5)^2*sin(e4) - 1.0*de1*m6*x6*y6*cos(e2)*cos(e4)^2*cos(e5)*sin(e3) - 1.0*de1*m6*x6*y6*cos(e3)*cos(e4)^2*cos(e5)*sin(e2) - 1.0*de1*m6*x6*y6*cos(e2)*cos(e5)*cos(e6)^2*sin(e3) - 1.0*de1*m6*x6*y6*cos(e3)*cos(e5)*cos(e6)^2*sin(e2) - 1.0*de1*m5*x5*z5*cos(e2)*cos(e4)^2*cos(e5)*sin(e3) - 1.0*de1*m5*x5*z5*cos(e3)*cos(e4)^2*cos(e5)*sin(e2) + 2.0*de6*m6*y6*z6*cos(e4)^2*cos(e5)*cos(e6)*sin(e5) + 4.0*de5*m6*x6*y6*cos(e4)*cos(e6)^2*sin(e4)*sin(e5) + 2.0*de6*m6*x6*z6*cos(e4)^2*cos(e5)*sin(e5)*sin(e6) + de1*m5*y5*z5*cos(e2)*cos(e4)^2*sin(e3)*sin(e5) + de1*m5*y5*z5*cos(e3)*cos(e4)^2*sin(e2)*sin(e5) - 1.0*de1*m5*x5*y5*cos(e5)^2*sin(e2)*sin(e3)*sin(e4) - 0.5*I6xx*de1*cos(e2)*cos(e3)*cos(e4)*cos(e6)*sin(e5)*sin(e6) + 0.5*I6yy*de1*cos(e2)*cos(e3)*cos(e4)*cos(e6)*sin(e5)*sin(e6) + 0.5*I6xx*de1*cos(e4)*cos(e6)*sin(e2)*sin(e3)*sin(e5)*sin(e6) - 0.5*I6yy*de1*cos(e4)*cos(e6)*sin(e2)*sin(e3)*sin(e5)*sin(e6) + 0.5*d4*de1*m6*x6*cos(e2)*cos(e3)*cos(e5)*cos(e6)*sin(e4) + 0.5*de1*m6*y6*z6*cos(e2)*cos(e3)*cos(e4)*cos(e5)*cos(e6) + 0.5*a3*de1*m6*x6*cos(e2)*cos(e5)*cos(e6)*sin(e3)*sin(e4) + 0.5*a3*de1*m6*x6*cos(e3)*cos(e5)*cos(e6)*sin(e2)*sin(e4) - 0.5*d4*de1*m6*y6*cos(e2)*cos(e3)*cos(e5)*sin(e4)*sin(e6) + 0.5*de1*m6*x6*z6*cos(e2)*cos(e3)*cos(e4)*cos(e5)*sin(e6) - 0.5*a3*de1*m6*y6*cos(e2)*cos(e5)*sin(e3)*sin(e4)*sin(e6) - 0.5*a3*de1*m6*y6*cos(e3)*cos(e5)*sin(e2)*sin(e4)*sin(e6) - 0.5*d4*de1*m6*x6*cos(e5)*cos(e6)*sin(e2)*sin(e3)*sin(e4) + 8.0*de6*m6*x6*y6*cos(e4)*cos(e5)*cos(e6)*sin(e4)*sin(e6) + 4.0*de4*m6*x6*z6*cos(e4)*cos(e5)*cos(e6)*sin(e4)*sin(e5) - 0.5*de1*m6*y6*z6*cos(e4)*cos(e5)*cos(e6)*sin(e2)*sin(e3) + 0.5*d4*de1*m6*y6*cos(e5)*sin(e2)*sin(e3)*sin(e4)*sin(e6) + 0.5*de1*m6*x6^2*cos(e2)*cos(e3)*cos(e5)*cos(e6)^2*sin(e4)*sin(e5) + de1*m6*x6^2*cos(e2)*cos(e4)^2*cos(e5)*cos(e6)*sin(e3)*sin(e6) + de1*m6*x6^2*cos(e3)*cos(e4)^2*cos(e5)*cos(e6)*sin(e2)*sin(e6) - 0.5*de1*m6*y6^2*cos(e2)*cos(e3)*cos(e5)*cos(e6)^2*sin(e4)*sin(e5) - 1.0*de1*m6*y6^2*cos(e2)*cos(e4)^2*cos(e5)*cos(e6)*sin(e3)*sin(e6) - 1.0*de1*m6*y6^2*cos(e3)*cos(e4)^2*cos(e5)*cos(e6)*sin(e2)*sin(e6) - 0.5*de1*m6*x6*z6*cos(e4)*cos(e5)*sin(e2)*sin(e3)*sin(e6) - 4.0*de4*m6*y6*z6*cos(e4)*cos(e5)*sin(e4)*sin(e5)*sin(e6) - 0.5*de1*m6*x6^2*cos(e5)*cos(e6)^2*sin(e2)*sin(e3)*sin(e4)*sin(e5) + 0.5*de1*m6*y6^2*cos(e5)*cos(e6)^2*sin(e2)*sin(e3)*sin(e4)*sin(e5) + de1*m6*x6*y6*cos(e2)*cos(e3)*cos(e4)*cos(e6)^2*sin(e5) + de1*m6*x6*z6*cos(e2)*cos(e3)*cos(e5)^2*cos(e6)*sin(e4) + 4.0*de4*m6*x6*y6*cos(e4)*cos(e5)^2*cos(e6)*sin(e4)*sin(e6) + 4.0*de5*m6*x6*y6*cos(e4)^2*cos(e5)*cos(e6)*sin(e5)*sin(e6) - 1.0*de1*m6*y6*z6*cos(e2)*cos(e3)*cos(e5)^2*sin(e4)*sin(e6) - 1.0*de1*m6*y6*z6*cos(e2)*cos(e4)^2*cos(e6)*sin(e3)*sin(e5) - 1.0*de1*m6*y6*z6*cos(e3)*cos(e4)^2*cos(e6)*sin(e2)*sin(e5) + 0.5*de1*m6*x6^2*cos(e2)*cos(e4)*cos(e5)^2*cos(e6)^2*sin(e3)*sin(e4) + 0.5*de1*m6*x6^2*cos(e3)*cos(e4)*cos(e5)^2*cos(e6)^2*sin(e2)*sin(e4) - 0.5*de1*m6*y6^2*cos(e2)*cos(e4)*cos(e5)^2*cos(e6)^2*sin(e3)*sin(e4) - 0.5*de1*m6*y6^2*cos(e3)*cos(e4)*cos(e5)^2*cos(e6)^2*sin(e2)*sin(e4) - 1.0*de1*m6*x6*y6*cos(e4)*cos(e6)^2*sin(e2)*sin(e3)*sin(e5) - 1.0*de1*m6*x6*z6*cos(e2)*cos(e4)^2*sin(e3)*sin(e5)*sin(e6) - 1.0*de1*m6*x6*z6*cos(e3)*cos(e4)^2*sin(e2)*sin(e5)*sin(e6) - 1.0*de1*m6*x6*z6*cos(e5)^2*cos(e6)*sin(e2)*sin(e3)*sin(e4) + de1*m6*y6*z6*cos(e5)^2*sin(e2)*sin(e3)*sin(e4)*sin(e6) + 0.5*de1*m6*x6^2*cos(e2)*cos(e3)*cos(e4)*cos(e6)*sin(e5)*sin(e6) + 2.0*de1*m6*x6*y6*cos(e2)*cos(e4)^2*cos(e5)*cos(e6)^2*sin(e3) + 2.0*de1*m6*x6*y6*cos(e3)*cos(e4)^2*cos(e5)*cos(e6)^2*sin(e2) - 0.5*de1*m6*y6^2*cos(e2)*cos(e3)*cos(e4)*cos(e6)*sin(e5)*sin(e6) - 0.5*de1*m6*x6^2*cos(e4)*cos(e6)*sin(e2)*sin(e3)*sin(e5)*sin(e6) + 0.5*de1*m6*y6^2*cos(e4)*cos(e6)*sin(e2)*sin(e3)*sin(e5)*sin(e6) - 1.0*de1*m5*x5*y5*cos(e2)*cos(e4)*cos(e5)*sin(e3)*sin(e4)*sin(e5) - 1.0*de1*m5*x5*y5*cos(e3)*cos(e4)*cos(e5)*sin(e2)*sin(e4)*sin(e5) - 1.0*de1*m6*x6*y6*cos(e2)*cos(e4)*cos(e6)*sin(e3)*sin(e4)*sin(e6) - 1.0*de1*m6*x6*y6*cos(e3)*cos(e4)*cos(e6)*sin(e2)*sin(e4)*sin(e6) - 1.0*de1*m6*x6*y6*cos(e2)*cos(e4)*cos(e5)^2*cos(e6)*sin(e3)*sin(e4)*sin(e6) - 1.0*de1*m6*x6*y6*cos(e3)*cos(e4)*cos(e5)^2*cos(e6)*sin(e2)*sin(e4)*sin(e6) - 1.0*de1*m6*x6*y6*cos(e2)*cos(e3)*cos(e5)*cos(e6)*sin(e4)*sin(e5)*sin(e6) - 1.0*de1*m6*x6*z6*cos(e2)*cos(e4)*cos(e5)*cos(e6)*sin(e3)*sin(e4)*sin(e5) - 1.0*de1*m6*x6*z6*cos(e3)*cos(e4)*cos(e5)*cos(e6)*sin(e2)*sin(e4)*sin(e5) + de1*m6*y6*z6*cos(e2)*cos(e4)*cos(e5)*sin(e3)*sin(e4)*sin(e5)*sin(e6) + de1*m6*y6*z6*cos(e3)*cos(e4)*cos(e5)*sin(e2)*sin(e4)*sin(e5)*sin(e6) + de1*m6*x6*y6*cos(e5)*cos(e6)*sin(e2)*sin(e3)*sin(e4)*sin(e5)*sin(e6);
C34 = I5xx*de5*sin(e4) - 1.0*I5yy*de5*sin(e4) + I6yy*de5*sin(e4) - 1.0*I6zz*de5*sin(e4) - 2.0*I5xx*de5*cos(e5)^2*sin(e4) + I6xx*de5*cos(e6)^2*sin(e4) + 2.0*I5yy*de5*cos(e5)^2*sin(e4) - 2.0*I6yy*de5*cos(e5)^2*sin(e4) - 1.0*I6yy*de5*cos(e6)^2*sin(e4) + 2.0*I6zz*de5*cos(e5)^2*sin(e4) + 0.5*I5xx*de1*cos(e2)*cos(e3) + 0.5*I6yy*de1*cos(e2)*cos(e3) + 0.5*I4zz*de1*cos(e2)*cos(e3) + I6xx*de6*cos(e4)*sin(e5) - 1.0*I6yy*de6*cos(e4)*sin(e5) - (I5xx*de1*sin(e2)*sin(e3))/2 - (I6yy*de1*sin(e2)*sin(e3))/2 - (I4zz*de1*sin(e2)*sin(e3))/2 - 1.0*de5*m5*x5^2*sin(e4) + de5*m5*y5^2*sin(e4) - 1.0*de5*m6*y6^2*sin(e4) + de5*m6*z6^2*sin(e4) + 2.0*de5*m5*x5^2*cos(e5)^2*sin(e4) - 1.0*de5*m6*x6^2*cos(e6)^2*sin(e4) - 2.0*de5*m5*y5^2*cos(e5)^2*sin(e4) + 2.0*de5*m6*y6^2*cos(e5)^2*sin(e4) + de5*m6*y6^2*cos(e6)^2*sin(e4) - 2.0*de5*m6*z6^2*cos(e5)^2*sin(e4) - 2.0*I6xx*de5*cos(e5)^2*cos(e6)^2*sin(e4) + 2.0*I6yy*de5*cos(e5)^2*cos(e6)^2*sin(e4) - 1.0*I5xx*de4*cos(e4)*cos(e5)*sin(e5) + I5yy*de4*cos(e4)*cos(e5)*sin(e5) - 1.0*I6yy*de4*cos(e4)*cos(e5)*sin(e5) + I6zz*de4*cos(e4)*cos(e5)*sin(e5) + 0.5*de1*m4*x4^2*cos(e2)*cos(e3) + 0.5*de1*m6*x6^2*cos(e2)*cos(e3) + 0.5*de1*m4*y4^2*cos(e2)*cos(e3) + 0.5*de1*m5*y5^2*cos(e2)*cos(e3) + 0.5*de1*m5*z5^2*cos(e2)*cos(e3) + 0.5*de1*m6*z6^2*cos(e2)*cos(e3) - 1.0*de6*m6*x6^2*cos(e4)*sin(e5) + de6*m6*y6^2*cos(e4)*sin(e5) - (de1*m4*x4^2*sin(e2)*sin(e3))/2 - (de1*m6*x6^2*sin(e2)*sin(e3))/2 - (de1*m4*y4^2*sin(e2)*sin(e3))/2 - (de1*m5*y5^2*sin(e2)*sin(e3))/2 - (de1*m5*z5^2*sin(e2)*sin(e3))/2 - (de1*m6*z6^2*sin(e2)*sin(e3))/2 - (I5xx*de1*cos(e2)*cos(e3)*cos(e5)^2)/2 + 0.5*I6xx*de1*cos(e2)*cos(e3)*cos(e6)^2 + 0.5*I5yy*de1*cos(e2)*cos(e3)*cos(e5)^2 - (I6yy*de1*cos(e2)*cos(e3)*cos(e5)^2)/2 - (I6yy*de1*cos(e2)*cos(e3)*cos(e6)^2)/2 + 0.5*I6zz*de1*cos(e2)*cos(e3)*cos(e5)^2 + d4*de4*m4*x4*cos(e4) - 2.0*I6xx*de6*cos(e4)*cos(e6)^2*sin(e5) + 2.0*I6yy*de6*cos(e4)*cos(e6)^2*sin(e5) + 0.5*I5xx*de1*cos(e5)^2*sin(e2)*sin(e3) - (I6xx*de1*cos(e6)^2*sin(e2)*sin(e3))/2 - (I5yy*de1*cos(e5)^2*sin(e2)*sin(e3))/2 + 0.5*I6yy*de1*cos(e5)^2*sin(e2)*sin(e3) + 0.5*I6yy*de1*cos(e6)^2*sin(e2)*sin(e3) - (I6zz*de1*cos(e5)^2*sin(e2)*sin(e3))/2 - 1.0*d4*de4*m4*y4*sin(e4) + d4*de4*m5*z5*sin(e4) - 1.0*de4*m5*x5*y5*cos(e4) + de4*m4*x4*z4*cos(e4) - 1.0*de4*m4*y4*z4*sin(e4) + 0.5*I6xx*de1*cos(e5)^2*cos(e6)^2*sin(e2)*sin(e3) - (I6yy*de1*cos(e5)^2*cos(e6)^2*sin(e2)*sin(e3))/2 + 2.0*de4*m5*x5*y5*cos(e4)*cos(e5)^2 + 2.0*de5*m6*x6^2*cos(e5)^2*cos(e6)^2*sin(e4) - 2.0*de5*m6*y6^2*cos(e5)^2*cos(e6)^2*sin(e4) - 1.0*I6xx*de5*cos(e4)*cos(e5)*cos(e6)*sin(e6) + I6yy*de5*cos(e4)*cos(e5)*cos(e6)*sin(e6) + I6xx*de4*cos(e6)*sin(e4)*sin(e5)*sin(e6) - 1.0*I6yy*de4*cos(e6)*sin(e4)*sin(e5)*sin(e6) + de4*m5*x5^2*cos(e4)*cos(e5)*sin(e5) - 1.0*de4*m5*y5^2*cos(e4)*cos(e5)*sin(e5) + de4*m6*y6^2*cos(e4)*cos(e5)*sin(e5) - 1.0*de4*m6*z6^2*cos(e4)*cos(e5)*sin(e5) + 0.5*a2*de2*m4*y4*cos(e3)*cos(e4) - (a2*de2*m5*z5*cos(e3)*cos(e4))/2 + d4*de4*m5*x5*cos(e4)*cos(e5) + d4*de6*m6*x6*cos(e4)*cos(e6) - 1.0*I6xx*de4*cos(e4)*cos(e5)*cos(e6)^2*sin(e5) + I6yy*de4*cos(e4)*cos(e5)*cos(e6)^2*sin(e5) + 0.5*a2*de2*m4*x4*cos(e3)*sin(e4) - 1.0*d4*de4*m5*y5*cos(e4)*sin(e5) - 1.0*d4*de5*m5*y5*cos(e5)*sin(e4) - 1.0*d4*de4*m6*y6*cos(e6)*sin(e4) - 1.0*d4*de6*m6*y6*cos(e4)*sin(e6) - 1.0*d4*de4*m6*z6*cos(e4)*sin(e5) - 1.0*d4*de5*m6*z6*cos(e5)*sin(e4) - 1.0*de5*m6*x6*y6*cos(e4)*cos(e5) - 1.0*de5*m5*x5*z5*cos(e4)*cos(e5) - 1.0*de4*m6*x6*z6*cos(e4)*cos(e6) - 1.0*d4*de5*m5*x5*sin(e4)*sin(e5) - 1.0*d4*de4*m6*x6*sin(e4)*sin(e6) + 0.5*de1*m5*x5^2*cos(e2)*cos(e3)*cos(e5)^2 - (de1*m6*x6^2*cos(e2)*cos(e3)*cos(e6)^2)/2 - (de1*m5*y5^2*cos(e2)*cos(e3)*cos(e5)^2)/2 + 0.5*de1*m6*y6^2*cos(e2)*cos(e3)*cos(e5)^2 + 0.5*de1*m6*y6^2*cos(e2)*cos(e3)*cos(e6)^2 - (de1*m6*z6^2*cos(e2)*cos(e3)*cos(e5)^2)/2 + de4*m5*y5*z5*cos(e5)*sin(e4) + de5*m5*y5*z5*cos(e4)*sin(e5) + de4*m6*y6*z6*cos(e4)*sin(e6) + de6*m6*y6*z6*cos(e6)*sin(e4) + 2.0*de6*m6*x6^2*cos(e4)*cos(e6)^2*sin(e5) - 2.0*de6*m6*y6^2*cos(e4)*cos(e6)^2*sin(e5) + de4*m6*x6*y6*sin(e4)*sin(e5) + de4*m5*x5*z5*sin(e4)*sin(e5) + de6*m6*x6*z6*sin(e4)*sin(e6) - (de1*m5*x5^2*cos(e5)^2*sin(e2)*sin(e3))/2 + 0.5*de1*m6*x6^2*cos(e6)^2*sin(e2)*sin(e3) + 0.5*de1*m5*y5^2*cos(e5)^2*sin(e2)*sin(e3) - (de1*m6*y6^2*cos(e5)^2*sin(e2)*sin(e3))/2 - (de1*m6*y6^2*cos(e6)^2*sin(e2)*sin(e3))/2 + 0.5*de1*m6*z6^2*cos(e5)^2*sin(e2)*sin(e3) - (I6xx*de1*cos(e2)*cos(e3)*cos(e5)^2*cos(e6)^2)/2 + 0.5*I6yy*de1*cos(e2)*cos(e3)*cos(e5)^2*cos(e6)^2 - (de1*m6*x6^2*cos(e5)^2*cos(e6)^2*sin(e2)*sin(e3))/2 + 0.5*de1*m6*y6^2*cos(e5)^2*cos(e6)^2*sin(e2)*sin(e3) + 0.5*I5xx*de1*cos(e2)*cos(e4)*cos(e5)*sin(e3)*sin(e5) + 0.5*I5xx*de1*cos(e3)*cos(e4)*cos(e5)*sin(e2)*sin(e5) - (I5yy*de1*cos(e2)*cos(e4)*cos(e5)*sin(e3)*sin(e5))/2 - (I5yy*de1*cos(e3)*cos(e4)*cos(e5)*sin(e2)*sin(e5))/2 + 0.5*I6yy*de1*cos(e2)*cos(e4)*cos(e5)*sin(e3)*sin(e5) + 0.5*I6yy*de1*cos(e3)*cos(e4)*cos(e5)*sin(e2)*sin(e5) - (I6zz*de1*cos(e2)*cos(e4)*cos(e5)*sin(e3)*sin(e5))/2 - (I6zz*de1*cos(e3)*cos(e4)*cos(e5)*sin(e2)*sin(e5))/2 + 2.0*I6xx*de6*cos(e5)*cos(e6)*sin(e4)*sin(e5)*sin(e6) - 2.0*I6yy*de6*cos(e5)*cos(e6)*sin(e4)*sin(e5)*sin(e6) + de5*m6*x6^2*cos(e4)*cos(e5)*cos(e6)*sin(e6) - 1.0*de5*m6*y6^2*cos(e4)*cos(e5)*cos(e6)*sin(e6) - 1.0*de4*m6*x6^2*cos(e6)*sin(e4)*sin(e5)*sin(e6) + de4*m6*y6^2*cos(e6)*sin(e4)*sin(e5)*sin(e6) + 0.5*a3*de1*m4*x4*cos(e2)*cos(e3)*cos(e4) + 0.5*a2*de2*m6*y6*cos(e3)*cos(e4)*cos(e6) + d4*de4*m6*x6*cos(e4)*cos(e5)*cos(e6) + 0.5*a2*de2*m5*x5*cos(e3)*cos(e5)*sin(e4) + 0.5*a2*de2*m6*x6*cos(e3)*cos(e4)*sin(e6) - (a3*de1*m4*y4*cos(e2)*cos(e3)*sin(e4))/2 + 0.5*a3*de1*m5*z5*cos(e2)*cos(e3)*sin(e4) - (d4*de1*m4*x4*cos(e2)*cos(e4)*sin(e3))/2 - (d4*de1*m4*x4*cos(e3)*cos(e4)*sin(e2))/2 - 1.0*d4*de4*m6*y6*cos(e4)*cos(e5)*sin(e6) - 1.0*d4*de6*m6*y6*cos(e5)*cos(e6)*sin(e4) + de6*m6*x6*z6*cos(e4)*cos(e5)*cos(e6) - (a3*de1*m4*x4*cos(e4)*sin(e2)*sin(e3))/2 - (a2*de2*m5*y5*cos(e3)*sin(e4)*sin(e5))/2 - (a2*de2*m6*z6*cos(e3)*sin(e4)*sin(e5))/2 - 1.0*d4*de5*m6*x6*cos(e6)*sin(e4)*sin(e5) - 1.0*d4*de6*m6*x6*cos(e5)*sin(e4)*sin(e6) + 0.5*d4*de1*m4*y4*cos(e2)*sin(e3)*sin(e4) + 0.5*d4*de1*m4*y4*cos(e3)*sin(e2)*sin(e4) - (d4*de1*m5*z5*cos(e2)*sin(e3)*sin(e4))/2 - (d4*de1*m5*z5*cos(e3)*sin(e2)*sin(e4))/2 + 0.5*de1*m5*x5*y5*cos(e2)*cos(e4)*sin(e3) + 0.5*de1*m5*x5*y5*cos(e3)*cos(e4)*sin(e2) - (de1*m4*x4*z4*cos(e2)*cos(e4)*sin(e3))/2 - (de1*m4*x4*z4*cos(e3)*cos(e4)*sin(e2))/2 - 1.0*de4*m6*y6*z6*cos(e5)*cos(e6)*sin(e4) - 1.0*de5*m6*y6*z6*cos(e4)*cos(e6)*sin(e5) - 1.0*de6*m6*y6*z6*cos(e4)*cos(e5)*sin(e6) + 0.5*a3*de1*m4*y4*sin(e2)*sin(e3)*sin(e4) - (a3*de1*m5*z5*sin(e2)*sin(e3)*sin(e4))/2 + d4*de5*m6*y6*sin(e4)*sin(e5)*sin(e6) + de4*m6*x6^2*cos(e4)*cos(e5)*cos(e6)^2*sin(e5) - 1.0*de4*m6*y6^2*cos(e4)*cos(e5)*cos(e6)^2*sin(e5) - 4.0*de5*m5*x5*y5*cos(e5)*sin(e4)*sin(e5) + 2.0*de6*m6*x6*y6*cos(e5)*sin(e4)*sin(e5) + 2.0*de5*m6*x6*y6*cos(e6)*sin(e4)*sin(e6) - 1.0*de4*m6*x6*z6*cos(e5)*sin(e4)*sin(e6) - 1.0*de5*m6*x6*z6*cos(e4)*sin(e5)*sin(e6) + 0.5*de1*m4*y4*z4*cos(e2)*sin(e3)*sin(e4) + 0.5*de1*m4*y4*z4*cos(e3)*sin(e2)*sin(e4) + 2.0*de5*m6*x6*y6*cos(e4)*cos(e5)*cos(e6)^2 + 2.0*de4*m6*x6*z6*cos(e4)*cos(e5)^2*cos(e6) + 0.5*de1*m6*x6^2*cos(e2)*cos(e3)*cos(e5)^2*cos(e6)^2 - (de1*m6*y6^2*cos(e2)*cos(e3)*cos(e5)^2*cos(e6)^2)/2 - 2.0*de4*m6*y6*z6*cos(e4)*cos(e5)^2*sin(e6) - 2.0*de6*m6*y6*z6*cos(e5)^2*cos(e6)*sin(e4) - 2.0*de4*m6*x6*y6*cos(e6)^2*sin(e4)*sin(e5) - 2.0*de6*m6*x6*z6*cos(e5)^2*sin(e4)*sin(e6) - (de1*m5*x5^2*cos(e2)*cos(e4)*cos(e5)*sin(e3)*sin(e5))/2 - (de1*m5*x5^2*cos(e3)*cos(e4)*cos(e5)*sin(e2)*sin(e5))/2 + 0.5*de1*m5*y5^2*cos(e2)*cos(e4)*cos(e5)*sin(e3)*sin(e5) + 0.5*de1*m5*y5^2*cos(e3)*cos(e4)*cos(e5)*sin(e2)*sin(e5) - (de1*m6*y6^2*cos(e2)*cos(e4)*cos(e5)*sin(e3)*sin(e5))/2 - (de1*m6*y6^2*cos(e3)*cos(e4)*cos(e5)*sin(e2)*sin(e5))/2 + 0.5*de1*m6*z6^2*cos(e2)*cos(e4)*cos(e5)*sin(e3)*sin(e5) + 0.5*de1*m6*z6^2*cos(e3)*cos(e4)*cos(e5)*sin(e2)*sin(e5) - 2.0*de6*m6*x6^2*cos(e5)*cos(e6)*sin(e4)*sin(e5)*sin(e6) + 2.0*de6*m6*y6^2*cos(e5)*cos(e6)*sin(e4)*sin(e5)*sin(e6) + 0.5*a3*de1*m5*x5*cos(e2)*cos(e3)*cos(e4)*cos(e5) + 0.5*a2*de2*m6*x6*cos(e3)*cos(e5)*cos(e6)*sin(e4) - (a3*de1*m5*y5*cos(e2)*cos(e3)*cos(e4)*sin(e5))/2 - (a3*de1*m6*y6*cos(e2)*cos(e3)*cos(e6)*sin(e4))/2 - (a3*de1*m6*z6*cos(e2)*cos(e3)*cos(e4)*sin(e5))/2 - (d4*de1*m5*x5*cos(e2)*cos(e4)*cos(e5)*sin(e3))/2 - (d4*de1*m5*x5*cos(e3)*cos(e4)*cos(e5)*sin(e2))/2 + 0.5*I6xx*de1*cos(e2)*cos(e4)*cos(e5)*cos(e6)^2*sin(e3)*sin(e5) + 0.5*I6xx*de1*cos(e3)*cos(e4)*cos(e5)*cos(e6)^2*sin(e2)*sin(e5) - (I6yy*de1*cos(e2)*cos(e4)*cos(e5)*cos(e6)^2*sin(e3)*sin(e5))/2 - (I6yy*de1*cos(e3)*cos(e4)*cos(e5)*cos(e6)^2*sin(e2)*sin(e5))/2 - (a3*de1*m5*x5*cos(e4)*cos(e5)*sin(e2)*sin(e3))/2 - (a3*de1*m6*x6*cos(e2)*cos(e3)*sin(e4)*sin(e6))/2 - (a2*de2*m6*y6*cos(e3)*cos(e5)*sin(e4)*sin(e6))/2 + 0.5*d4*de1*m5*y5*cos(e2)*cos(e4)*sin(e3)*sin(e5) + 0.5*d4*de1*m5*y5*cos(e3)*cos(e4)*sin(e2)*sin(e5) + 0.5*d4*de1*m6*y6*cos(e2)*cos(e6)*sin(e3)*sin(e4) + 0.5*d4*de1*m6*y6*cos(e3)*cos(e6)*sin(e2)*sin(e4) + 0.5*d4*de1*m6*z6*cos(e2)*cos(e4)*sin(e3)*sin(e5) + 0.5*d4*de1*m6*z6*cos(e3)*cos(e4)*sin(e2)*sin(e5) - 1.0*de1*m5*x5*y5*cos(e2)*cos(e3)*cos(e5)*sin(e5) + de1*m6*x6*y6*cos(e2)*cos(e3)*cos(e6)*sin(e6) + 0.5*de1*m6*x6*z6*cos(e2)*cos(e4)*cos(e6)*sin(e3) + 0.5*de1*m6*x6*z6*cos(e3)*cos(e4)*cos(e6)*sin(e2) + 0.5*a3*de1*m5*y5*cos(e4)*sin(e2)*sin(e3)*sin(e5) + 0.5*a3*de1*m6*y6*cos(e6)*sin(e2)*sin(e3)*sin(e4) + 0.5*a3*de1*m6*z6*cos(e4)*sin(e2)*sin(e3)*sin(e5) + 0.5*d4*de1*m6*x6*cos(e2)*sin(e3)*sin(e4)*sin(e6) + 0.5*d4*de1*m6*x6*cos(e3)*sin(e2)*sin(e4)*sin(e6) - 4.0*de6*m6*x6*y6*cos(e4)*cos(e6)*sin(e5)*sin(e6) - 4.0*de5*m6*x6*z6*cos(e5)*cos(e6)*sin(e4)*sin(e5) - (de1*m5*y5*z5*cos(e2)*cos(e5)*sin(e3)*sin(e4))/2 - (de1*m5*y5*z5*cos(e3)*cos(e5)*sin(e2)*sin(e4))/2 - (de1*m6*y6*z6*cos(e2)*cos(e4)*sin(e3)*sin(e6))/2 - (de1*m6*y6*z6*cos(e3)*cos(e4)*sin(e2)*sin(e6))/2 + 0.5*a3*de1*m6*x6*sin(e2)*sin(e3)*sin(e4)*sin(e6) + de1*m5*x5*y5*cos(e5)*sin(e2)*sin(e3)*sin(e5) - (de1*m6*x6*y6*cos(e2)*sin(e3)*sin(e4)*sin(e5))/2 - (de1*m6*x6*y6*cos(e3)*sin(e2)*sin(e4)*sin(e5))/2 - 1.0*de1*m6*x6*y6*cos(e6)*sin(e2)*sin(e3)*sin(e6) - (de1*m5*x5*z5*cos(e2)*sin(e3)*sin(e4)*sin(e5))/2 - (de1*m5*x5*z5*cos(e3)*sin(e2)*sin(e4)*sin(e5))/2 + 4.0*de5*m6*y6*z6*cos(e5)*sin(e4)*sin(e5)*sin(e6) - 1.0*de1*m5*x5*y5*cos(e2)*cos(e4)*cos(e5)^2*sin(e3) - 1.0*de1*m5*x5*y5*cos(e3)*cos(e4)*cos(e5)^2*sin(e2) - 4.0*de5*m6*x6*y6*cos(e5)^2*cos(e6)*sin(e4)*sin(e6) - 4.0*de6*m6*x6*y6*cos(e5)*cos(e6)^2*sin(e4)*sin(e5) - (I6xx*de1*cos(e2)*cos(e6)*sin(e3)*sin(e4)*sin(e5)*sin(e6))/2 - (I6xx*de1*cos(e3)*cos(e6)*sin(e2)*sin(e4)*sin(e5)*sin(e6))/2 + 0.5*I6yy*de1*cos(e2)*cos(e6)*sin(e3)*sin(e4)*sin(e5)*sin(e6) + 0.5*I6yy*de1*cos(e3)*cos(e6)*sin(e2)*sin(e4)*sin(e5)*sin(e6) - (a3*de1*m6*y6*cos(e2)*cos(e3)*cos(e4)*cos(e5)*sin(e6))/2 - (d4*de1*m6*x6*cos(e2)*cos(e4)*cos(e5)*cos(e6)*sin(e3))/2 - (d4*de1*m6*x6*cos(e3)*cos(e4)*cos(e5)*cos(e6)*sin(e2))/2 - (a3*de1*m6*x6*cos(e4)*cos(e5)*cos(e6)*sin(e2)*sin(e3))/2 + 0.5*d4*de1*m6*y6*cos(e2)*cos(e4)*cos(e5)*sin(e3)*sin(e6) + 0.5*d4*de1*m6*y6*cos(e3)*cos(e4)*cos(e5)*sin(e2)*sin(e6) - 1.0*de1*m6*x6*z6*cos(e2)*cos(e3)*cos(e5)*cos(e6)*sin(e5) + 0.5*a3*de1*m6*y6*cos(e4)*cos(e5)*sin(e2)*sin(e3)*sin(e6) - 2.0*de4*m6*x6*y6*cos(e4)*cos(e5)*cos(e6)*sin(e5)*sin(e6) + 0.5*de1*m6*y6*z6*cos(e2)*cos(e5)*cos(e6)*sin(e3)*sin(e4) + 0.5*de1*m6*y6*z6*cos(e3)*cos(e5)*cos(e6)*sin(e2)*sin(e4) + de1*m6*y6*z6*cos(e2)*cos(e3)*cos(e5)*sin(e5)*sin(e6) - (de1*m6*x6^2*cos(e2)*cos(e4)*cos(e5)*cos(e6)^2*sin(e3)*sin(e5))/2 - (de1*m6*x6^2*cos(e3)*cos(e4)*cos(e5)*cos(e6)^2*sin(e2)*sin(e5))/2 + 0.5*de1*m6*y6^2*cos(e2)*cos(e4)*cos(e5)*cos(e6)^2*sin(e3)*sin(e5) + 0.5*de1*m6*y6^2*cos(e3)*cos(e4)*cos(e5)*cos(e6)^2*sin(e2)*sin(e5) + 0.5*de1*m6*x6*z6*cos(e2)*cos(e5)*sin(e3)*sin(e4)*sin(e6) + 0.5*de1*m6*x6*z6*cos(e3)*cos(e5)*sin(e2)*sin(e4)*sin(e6) + de1*m6*x6*z6*cos(e5)*cos(e6)*sin(e2)*sin(e3)*sin(e5) - 1.0*de1*m6*y6*z6*cos(e5)*sin(e2)*sin(e3)*sin(e5)*sin(e6) - 1.0*de1*m6*x6*y6*cos(e2)*cos(e3)*cos(e5)^2*cos(e6)*sin(e6) - 1.0*de1*m6*x6*z6*cos(e2)*cos(e4)*cos(e5)^2*cos(e6)*sin(e3) - 1.0*de1*m6*x6*z6*cos(e3)*cos(e4)*cos(e5)^2*cos(e6)*sin(e2) + de1*m6*y6*z6*cos(e2)*cos(e4)*cos(e5)^2*sin(e3)*sin(e6) + de1*m6*y6*z6*cos(e3)*cos(e4)*cos(e5)^2*sin(e2)*sin(e6) + de1*m6*x6*y6*cos(e2)*cos(e6)^2*sin(e3)*sin(e4)*sin(e5) + de1*m6*x6*y6*cos(e3)*cos(e6)^2*sin(e2)*sin(e4)*sin(e5) + de1*m6*x6*y6*cos(e5)^2*cos(e6)*sin(e2)*sin(e3)*sin(e6) + 0.5*a3*de1*m6*x6*cos(e2)*cos(e3)*cos(e4)*cos(e5)*cos(e6) + 0.5*de1*m6*x6^2*cos(e2)*cos(e6)*sin(e3)*sin(e4)*sin(e5)*sin(e6) + 0.5*de1*m6*x6^2*cos(e3)*cos(e6)*sin(e2)*sin(e4)*sin(e5)*sin(e6) - (de1*m6*y6^2*cos(e2)*cos(e6)*sin(e3)*sin(e4)*sin(e5)*sin(e6))/2 - (de1*m6*y6^2*cos(e3)*cos(e6)*sin(e2)*sin(e4)*sin(e5)*sin(e6))/2 + de1*m6*x6*y6*cos(e2)*cos(e4)*cos(e5)*cos(e6)*sin(e3)*sin(e5)*sin(e6) + de1*m6*x6*y6*cos(e3)*cos(e4)*cos(e5)*cos(e6)*sin(e2)*sin(e5)*sin(e6);
C35 = I6xx*de4*cos(e6)^2*sin(e4) - 1.0*I5zz*de4*sin(e4) - 1.0*I6xx*de4*sin(e4) - 1.0*I6yy*de4*cos(e6)^2*sin(e4) - 1.0*I6xx*de6*cos(e5)*sin(e4) + I6yy*de6*cos(e5)*sin(e4) - 1.0*de4*m5*x5^2*sin(e4) - 1.0*de4*m5*y5^2*sin(e4) - 1.0*de4*m6*y6^2*sin(e4) - 1.0*de4*m6*z6^2*sin(e4) - 1.0*de4*m6*x6^2*cos(e6)^2*sin(e4) + de4*m6*y6^2*cos(e6)^2*sin(e4) + 2.0*I6xx*de6*cos(e4)*cos(e6)*sin(e6) - 2.0*I6yy*de6*cos(e4)*cos(e6)*sin(e6) + 0.5*I6xx*de1*cos(e2)*sin(e3)*sin(e4) + 0.5*I6xx*de1*cos(e3)*sin(e2)*sin(e4) + 0.5*I5zz*de1*cos(e2)*sin(e3)*sin(e4) + 0.5*I5zz*de1*cos(e3)*sin(e2)*sin(e4) + de6*m6*x6^2*cos(e5)*sin(e4) - 1.0*de6*m6*y6^2*cos(e5)*sin(e4) - 1.0*a3*de5*m5*y5*cos(e5) - 1.0*a3*de5*m6*z6*cos(e5) + 2.0*I6xx*de6*cos(e5)*cos(e6)^2*sin(e4) - 2.0*I6yy*de6*cos(e5)*cos(e6)^2*sin(e4) - 1.0*a3*de5*m5*x5*sin(e5) + 2.0*de6*m6*x6*y6*cos(e4) - 4.0*de6*m6*x6*y6*cos(e4)*cos(e6)^2 + I6xx*de4*cos(e4)*cos(e5)*cos(e6)*sin(e6) - 1.0*I6yy*de4*cos(e4)*cos(e5)*cos(e6)*sin(e6) - 1.0*I6xx*de5*cos(e6)*sin(e4)*sin(e5)*sin(e6) + I6yy*de5*cos(e6)*sin(e4)*sin(e5)*sin(e6) - 2.0*de6*m6*x6^2*cos(e4)*cos(e6)*sin(e6) + 2.0*de6*m6*y6^2*cos(e4)*cos(e6)*sin(e6) + 0.5*de1*m5*x5^2*cos(e2)*sin(e3)*sin(e4) + 0.5*de1*m5*x5^2*cos(e3)*sin(e2)*sin(e4) + 0.5*de1*m5*y5^2*cos(e2)*sin(e3)*sin(e4) + 0.5*de1*m5*y5^2*cos(e3)*sin(e2)*sin(e4) + 0.5*de1*m6*y6^2*cos(e2)*sin(e3)*sin(e4) + 0.5*de1*m6*y6^2*cos(e3)*sin(e2)*sin(e4) + 0.5*de1*m6*z6^2*cos(e2)*sin(e3)*sin(e4) + 0.5*de1*m6*z6^2*cos(e3)*sin(e2)*sin(e4) - 1.0*a3*de6*m6*y6*cos(e5)*cos(e6) + d4*de5*m5*x5*cos(e4)*cos(e5) + 0.5*a2*de2*m5*x5*cos(e5)*sin(e3) - 1.0*a3*de5*m6*x6*cos(e6)*sin(e5) - 1.0*a3*de6*m6*x6*cos(e5)*sin(e6) - (I6xx*de1*cos(e2)*cos(e6)^2*sin(e3)*sin(e4))/2 - (I6xx*de1*cos(e3)*cos(e6)^2*sin(e2)*sin(e4))/2 + 0.5*I6yy*de1*cos(e2)*cos(e6)^2*sin(e3)*sin(e4) + 0.5*I6yy*de1*cos(e3)*cos(e6)^2*sin(e2)*sin(e4) - 1.0*d4*de4*m5*y5*cos(e5)*sin(e4) - 1.0*d4*de5*m5*y5*cos(e4)*sin(e5) - 1.0*d4*de4*m6*z6*cos(e5)*sin(e4) - 1.0*d4*de5*m6*z6*cos(e4)*sin(e5) + de4*m6*x6*y6*cos(e4)*cos(e5) + de4*m5*x5*z5*cos(e4)*cos(e5) - (a2*de2*m5*y5*sin(e3)*sin(e5))/2 + a3*de5*m6*y6*sin(e5)*sin(e6) - (a2*de2*m6*z6*sin(e3)*sin(e5))/2 - 1.0*d4*de4*m5*x5*sin(e4)*sin(e5) - 1.0*de4*m5*y5*z5*cos(e4)*sin(e5) - 1.0*de5*m5*y5*z5*cos(e5)*sin(e4) - 2.0*de6*m6*x6^2*cos(e5)*cos(e6)^2*sin(e4) + 2.0*de6*m6*y6^2*cos(e5)*cos(e6)^2*sin(e4) - 1.0*de5*m6*x6*y6*sin(e4)*sin(e5) - 1.0*de5*m5*x5*z5*sin(e4)*sin(e5) - (I6xx*de1*cos(e2)*cos(e3)*cos(e6)*sin(e5)*sin(e6))/2 + 0.5*I6yy*de1*cos(e2)*cos(e3)*cos(e6)*sin(e5)*sin(e6) + 0.5*I6xx*de1*cos(e6)*sin(e2)*sin(e3)*sin(e5)*sin(e6) - (I6yy*de1*cos(e6)*sin(e2)*sin(e3)*sin(e5)*sin(e6))/2 - 1.0*de4*m6*x6^2*cos(e4)*cos(e5)*cos(e6)*sin(e6) + de4*m6*y6^2*cos(e4)*cos(e5)*cos(e6)*sin(e6) + de5*m6*x6^2*cos(e6)*sin(e4)*sin(e5)*sin(e6) - 1.0*de5*m6*y6^2*cos(e6)*sin(e4)*sin(e5)*sin(e6) + 0.5*a2*de2*m5*y5*cos(e3)*cos(e4)*cos(e5) + 0.5*a2*de2*m6*z6*cos(e3)*cos(e4)*cos(e5) + d4*de5*m6*x6*cos(e4)*cos(e5)*cos(e6) + 0.5*a2*de2*m5*x5*cos(e3)*cos(e4)*sin(e5) + 0.5*a2*de2*m6*x6*cos(e5)*cos(e6)*sin(e3) - 1.0*d4*de5*m6*y6*cos(e4)*cos(e5)*sin(e6) - 1.0*d4*de6*m6*y6*cos(e4)*cos(e6)*sin(e5) - (de1*m5*y5*z5*cos(e2)*cos(e3)*cos(e5))/2 - (a2*de2*m6*y6*cos(e5)*sin(e3)*sin(e6))/2 - 1.0*d4*de4*m6*x6*cos(e6)*sin(e4)*sin(e5) - 1.0*d4*de6*m6*x6*cos(e4)*sin(e5)*sin(e6) - (de1*m6*x6*y6*cos(e2)*cos(e3)*sin(e5))/2 - (de1*m5*x5*z5*cos(e2)*cos(e3)*sin(e5))/2 + de4*m6*y6*z6*cos(e4)*cos(e6)*sin(e5) + de5*m6*y6*z6*cos(e5)*cos(e6)*sin(e4) + d4*de4*m6*y6*sin(e4)*sin(e5)*sin(e6) + 2.0*de4*m6*x6*y6*cos(e6)*sin(e4)*sin(e6) + de4*m6*x6*z6*cos(e4)*sin(e5)*sin(e6) + de5*m6*x6*z6*cos(e5)*sin(e4)*sin(e6) + de6*m6*x6*z6*cos(e6)*sin(e4)*sin(e5) + 0.5*de1*m5*y5*z5*cos(e5)*sin(e2)*sin(e3) + 0.5*de1*m6*x6^2*cos(e2)*cos(e6)^2*sin(e3)*sin(e4) + 0.5*de1*m6*x6^2*cos(e3)*cos(e6)^2*sin(e2)*sin(e4) - (de1*m6*y6^2*cos(e2)*cos(e6)^2*sin(e3)*sin(e4))/2 - (de1*m6*y6^2*cos(e3)*cos(e6)^2*sin(e2)*sin(e4))/2 + 0.5*de1*m6*x6*y6*sin(e2)*sin(e3)*sin(e5) + 0.5*de1*m5*x5*z5*sin(e2)*sin(e3)*sin(e5) - 1.0*de6*m6*y6*z6*sin(e4)*sin(e5)*sin(e6) - 2.0*de4*m6*x6*y6*cos(e4)*cos(e5)*cos(e6)^2 + 2.0*de5*m6*x6*y6*cos(e6)^2*sin(e4)*sin(e5) + 0.5*de1*m6*x6^2*cos(e2)*cos(e3)*cos(e6)*sin(e5)*sin(e6) - (de1*m6*y6^2*cos(e2)*cos(e3)*cos(e6)*sin(e5)*sin(e6))/2 - (de1*m6*x6^2*cos(e6)*sin(e2)*sin(e3)*sin(e5)*sin(e6))/2 + 0.5*de1*m6*y6^2*cos(e6)*sin(e2)*sin(e3)*sin(e5)*sin(e6) + 0.5*a2*de2*m6*x6*cos(e3)*cos(e4)*cos(e6)*sin(e5) - (a3*de1*m5*y5*cos(e2)*cos(e3)*cos(e5)*sin(e4))/2 - (a3*de1*m6*z6*cos(e2)*cos(e3)*cos(e5)*sin(e4))/2 + 0.5*de1*m6*y6*z6*cos(e2)*cos(e3)*cos(e5)*cos(e6) - (a3*de1*m5*x5*cos(e2)*cos(e3)*sin(e4)*sin(e5))/2 - (a2*de2*m6*y6*cos(e3)*cos(e4)*sin(e5)*sin(e6))/2 + 0.5*d4*de1*m5*y5*cos(e2)*cos(e5)*sin(e3)*sin(e4) + 0.5*d4*de1*m5*y5*cos(e3)*cos(e5)*sin(e2)*sin(e4) + 0.5*d4*de1*m6*z6*cos(e2)*cos(e5)*sin(e3)*sin(e4) + 0.5*d4*de1*m6*z6*cos(e3)*cos(e5)*sin(e2)*sin(e4) - (de1*m6*x6*y6*cos(e2)*cos(e4)*cos(e5)*sin(e3))/2 - (de1*m6*x6*y6*cos(e3)*cos(e4)*cos(e5)*sin(e2))/2 - (de1*m5*x5*z5*cos(e2)*cos(e4)*cos(e5)*sin(e3))/2 - (de1*m5*x5*z5*cos(e3)*cos(e4)*cos(e5)*sin(e2))/2 + 0.5*de1*m6*x6*z6*cos(e2)*cos(e3)*cos(e5)*sin(e6) + 0.5*a3*de1*m5*y5*cos(e5)*sin(e2)*sin(e3)*sin(e4) + 0.5*a3*de1*m6*z6*cos(e5)*sin(e2)*sin(e3)*sin(e4) + 0.5*d4*de1*m5*x5*cos(e2)*sin(e3)*sin(e4)*sin(e5) + 0.5*d4*de1*m5*x5*cos(e3)*sin(e2)*sin(e4)*sin(e5) + 4.0*de6*m6*x6*y6*cos(e5)*cos(e6)*sin(e4)*sin(e6) + 0.5*de1*m5*y5*z5*cos(e2)*cos(e4)*sin(e3)*sin(e5) + 0.5*de1*m5*y5*z5*cos(e3)*cos(e4)*sin(e2)*sin(e5) - (de1*m6*y6*z6*cos(e5)*cos(e6)*sin(e2)*sin(e3))/2 + 0.5*a3*de1*m5*x5*sin(e2)*sin(e3)*sin(e4)*sin(e5) - (de1*m6*x6*z6*cos(e5)*sin(e2)*sin(e3)*sin(e6))/2 + de1*m6*x6*y6*cos(e2)*cos(e3)*cos(e6)^2*sin(e5) - 1.0*de1*m6*x6*y6*cos(e6)^2*sin(e2)*sin(e3)*sin(e5) - (I6xx*de1*cos(e2)*cos(e4)*cos(e5)*cos(e6)*sin(e3)*sin(e6))/2 - (I6xx*de1*cos(e3)*cos(e4)*cos(e5)*cos(e6)*sin(e2)*sin(e6))/2 + 0.5*I6yy*de1*cos(e2)*cos(e4)*cos(e5)*cos(e6)*sin(e3)*sin(e6) + 0.5*I6yy*de1*cos(e3)*cos(e4)*cos(e5)*cos(e6)*sin(e2)*sin(e6) - (a3*de1*m6*x6*cos(e2)*cos(e3)*cos(e6)*sin(e4)*sin(e5))/2 + 0.5*a3*de1*m6*y6*cos(e2)*cos(e3)*sin(e4)*sin(e5)*sin(e6) + 0.5*d4*de1*m6*x6*cos(e2)*cos(e6)*sin(e3)*sin(e4)*sin(e5) + 0.5*d4*de1*m6*x6*cos(e3)*cos(e6)*sin(e2)*sin(e4)*sin(e5) - (de1*m6*y6*z6*cos(e2)*cos(e4)*cos(e6)*sin(e3)*sin(e5))/2 - (de1*m6*y6*z6*cos(e3)*cos(e4)*cos(e6)*sin(e2)*sin(e5))/2 + 0.5*a3*de1*m6*x6*cos(e6)*sin(e2)*sin(e3)*sin(e4)*sin(e5) - (d4*de1*m6*y6*cos(e2)*sin(e3)*sin(e4)*sin(e5)*sin(e6))/2 - (d4*de1*m6*y6*cos(e3)*sin(e2)*sin(e4)*sin(e5)*sin(e6))/2 - 1.0*de1*m6*x6*y6*cos(e2)*cos(e6)*sin(e3)*sin(e4)*sin(e6) - 1.0*de1*m6*x6*y6*cos(e3)*cos(e6)*sin(e2)*sin(e4)*sin(e6) - (de1*m6*x6*z6*cos(e2)*cos(e4)*sin(e3)*sin(e5)*sin(e6))/2 - (de1*m6*x6*z6*cos(e3)*cos(e4)*sin(e2)*sin(e5)*sin(e6))/2 - (a3*de1*m6*y6*sin(e2)*sin(e3)*sin(e4)*sin(e5)*sin(e6))/2 + de1*m6*x6*y6*cos(e2)*cos(e4)*cos(e5)*cos(e6)^2*sin(e3) + de1*m6*x6*y6*cos(e3)*cos(e4)*cos(e5)*cos(e6)^2*sin(e2) + 0.5*de1*m6*x6^2*cos(e2)*cos(e4)*cos(e5)*cos(e6)*sin(e3)*sin(e6) + 0.5*de1*m6*x6^2*cos(e3)*cos(e4)*cos(e5)*cos(e6)*sin(e2)*sin(e6) - (de1*m6*y6^2*cos(e2)*cos(e4)*cos(e5)*cos(e6)*sin(e3)*sin(e6))/2 - (de1*m6*y6^2*cos(e3)*cos(e4)*cos(e5)*cos(e6)*sin(e2)*sin(e6))/2;
C36 = I6zz*de4*cos(e4)*sin(e5) + I6zz*de5*cos(e5)*sin(e4) + (I6zz*de1*cos(e2)*cos(e3)*cos(e5))/2 - 0.5*I6zz*de1*cos(e5)*sin(e2)*sin(e3) + de4*m6*x6^2*cos(e4)*sin(e5) + de5*m6*x6^2*cos(e5)*sin(e4) + de4*m6*y6^2*cos(e4)*sin(e5) + de5*m6*y6^2*cos(e5)*sin(e4) - 0.5*I6zz*de1*cos(e2)*cos(e4)*sin(e3)*sin(e5) - 0.5*I6zz*de1*cos(e3)*cos(e4)*sin(e2)*sin(e5) + (de1*m6*x6^2*cos(e2)*cos(e3)*cos(e5))/2 + (de1*m6*y6^2*cos(e2)*cos(e3)*cos(e5))/2 - 0.5*de1*m6*x6^2*cos(e5)*sin(e2)*sin(e3) - 0.5*de1*m6*y6^2*cos(e5)*sin(e2)*sin(e3) - 1.0*a3*de5*m6*y6*cos(e5)*cos(e6) + d4*de4*m6*x6*cos(e4)*cos(e6) - 1.0*a3*de5*m6*x6*cos(e5)*sin(e6) - 1.0*a3*de6*m6*x6*cos(e6)*sin(e5) - 1.0*d4*de4*m6*y6*cos(e4)*sin(e6) - 1.0*d4*de6*m6*y6*cos(e6)*sin(e4) + de6*m6*x6*z6*cos(e4)*cos(e6) + a3*de6*m6*y6*sin(e5)*sin(e6) - 1.0*d4*de6*m6*x6*sin(e4)*sin(e6) - 1.0*de4*m6*y6*z6*cos(e6)*sin(e4) - 1.0*de6*m6*y6*z6*cos(e4)*sin(e6) - 1.0*de4*m6*x6*z6*sin(e4)*sin(e6) - 0.5*de1*m6*x6^2*cos(e2)*cos(e4)*sin(e3)*sin(e5) - 0.5*de1*m6*x6^2*cos(e3)*cos(e4)*sin(e2)*sin(e5) - 0.5*de1*m6*y6^2*cos(e2)*cos(e4)*sin(e3)*sin(e5) - 0.5*de1*m6*y6^2*cos(e3)*cos(e4)*sin(e2)*sin(e5) + d4*de6*m6*x6*cos(e4)*cos(e5)*cos(e6) + (a2*de2*m6*x6*cos(e3)*cos(e6)*sin(e4))/2 - 1.0*d4*de4*m6*y6*cos(e5)*cos(e6)*sin(e4) - 1.0*d4*de5*m6*y6*cos(e4)*cos(e6)*sin(e5) - 1.0*d4*de6*m6*y6*cos(e4)*cos(e5)*sin(e6) + de4*m6*x6*z6*cos(e4)*cos(e5)*cos(e6) - 0.5*a2*de2*m6*y6*cos(e3)*sin(e4)*sin(e6) - 0.5*a2*de2*m6*y6*cos(e6)*sin(e3)*sin(e5) - 1.0*d4*de4*m6*x6*cos(e5)*sin(e4)*sin(e6) - 1.0*d4*de5*m6*x6*cos(e4)*sin(e5)*sin(e6) - 1.0*de4*m6*y6*z6*cos(e4)*cos(e5)*sin(e6) - 1.0*de6*m6*y6*z6*cos(e5)*cos(e6)*sin(e4) - 0.5*a2*de2*m6*x6*sin(e3)*sin(e5)*sin(e6) - 1.0*de5*m6*x6*z6*cos(e6)*sin(e4)*sin(e5) - 1.0*de6*m6*x6*z6*cos(e5)*sin(e4)*sin(e6) + de5*m6*y6*z6*sin(e4)*sin(e5)*sin(e6) + (a3*de1*m6*x6*cos(e2)*cos(e3)*cos(e4)*cos(e6))/2 + (a2*de2*m6*y6*cos(e3)*cos(e4)*cos(e5)*cos(e6))/2 + (a2*de2*m6*x6*cos(e3)*cos(e4)*cos(e5)*sin(e6))/2 - 0.5*a3*de1*m6*y6*cos(e2)*cos(e3)*cos(e4)*sin(e6) - 0.5*d4*de1*m6*x6*cos(e2)*cos(e4)*cos(e6)*sin(e3) - 0.5*d4*de1*m6*x6*cos(e3)*cos(e4)*cos(e6)*sin(e2) - 0.5*a3*de1*m6*x6*cos(e4)*cos(e6)*sin(e2)*sin(e3) + (d4*de1*m6*y6*cos(e2)*cos(e4)*sin(e3)*sin(e6))/2 + (d4*de1*m6*y6*cos(e3)*cos(e4)*sin(e2)*sin(e6))/2 - 0.5*de1*m6*x6*z6*cos(e2)*cos(e3)*cos(e6)*sin(e5) + (a3*de1*m6*y6*cos(e4)*sin(e2)*sin(e3)*sin(e6))/2 + (de1*m6*y6*z6*cos(e2)*cos(e6)*sin(e3)*sin(e4))/2 + (de1*m6*y6*z6*cos(e3)*cos(e6)*sin(e2)*sin(e4))/2 + (de1*m6*y6*z6*cos(e2)*cos(e3)*sin(e5)*sin(e6))/2 + (de1*m6*x6*z6*cos(e2)*sin(e3)*sin(e4)*sin(e6))/2 + (de1*m6*x6*z6*cos(e3)*sin(e2)*sin(e4)*sin(e6))/2 + (de1*m6*x6*z6*cos(e6)*sin(e2)*sin(e3)*sin(e5))/2 - 0.5*de1*m6*y6*z6*sin(e2)*sin(e3)*sin(e5)*sin(e6) - 0.5*a3*de1*m6*y6*cos(e2)*cos(e3)*cos(e5)*cos(e6)*sin(e4) - 0.5*a3*de1*m6*x6*cos(e2)*cos(e3)*cos(e5)*sin(e4)*sin(e6) + (d4*de1*m6*y6*cos(e2)*cos(e5)*cos(e6)*sin(e3)*sin(e4))/2 + (d4*de1*m6*y6*cos(e3)*cos(e5)*cos(e6)*sin(e2)*sin(e4))/2 - 0.5*de1*m6*x6*z6*cos(e2)*cos(e4)*cos(e5)*cos(e6)*sin(e3) - 0.5*de1*m6*x6*z6*cos(e3)*cos(e4)*cos(e5)*cos(e6)*sin(e2) + (a3*de1*m6*y6*cos(e5)*cos(e6)*sin(e2)*sin(e3)*sin(e4))/2 + (d4*de1*m6*x6*cos(e2)*cos(e5)*sin(e3)*sin(e4)*sin(e6))/2 + (d4*de1*m6*x6*cos(e3)*cos(e5)*sin(e2)*sin(e4)*sin(e6))/2 + (de1*m6*y6*z6*cos(e2)*cos(e4)*cos(e5)*sin(e3)*sin(e6))/2 + (de1*m6*y6*z6*cos(e3)*cos(e4)*cos(e5)*sin(e2)*sin(e6))/2 + (a3*de1*m6*x6*cos(e5)*sin(e2)*sin(e3)*sin(e4)*sin(e6))/2;
 
C411 = (I4xx*de1*sin(2*e4))/2 - 0.5*I6xx*de1*sin(2*e4) - 0.5*I4yy*de1*sin(2*e4) + (I5yy*de1*sin(2*e4))/2 - 0.5*I5zz*de1*sin(2*e4) + (I6zz*de1*sin(2*e4))/2 + de1*m4*x4*y4 - 0.5*de1*m4*x4^2*sin(2*e4) + (de1*m6*x6^2*sin(2*e4))/2 + (de1*m4*y4^2*sin(2*e4))/2 - 0.5*de1*m5*y5^2*sin(2*e4) + (de1*m5*z5^2*sin(2*e4))/2 - 0.5*de1*m6*z6^2*sin(2*e4) - 0.5*I4xx*de2*cos(e2)*cos(e3) - 0.5*I4xx*de3*cos(e2)*cos(e3) - 1.0*I5xx*de2*cos(e2)*cos(e3) - 1.0*I5xx*de3*cos(e2)*cos(e3) + 0.5*I6xx*de2*cos(e2)*cos(e3) + 0.5*I6xx*de3*cos(e2)*cos(e3) + 0.5*I4yy*de2*cos(e2)*cos(e3) + 0.5*I4yy*de3*cos(e2)*cos(e3) - 0.5*I5yy*de2*cos(e2)*cos(e3) - 0.5*I5yy*de3*cos(e2)*cos(e3) - 1.0*I6yy*de2*cos(e2)*cos(e3) - 1.0*I6yy*de3*cos(e2)*cos(e3) - 1.0*I4zz*de2*cos(e2)*cos(e3) - 1.0*I4zz*de3*cos(e2)*cos(e3) + 0.5*I5zz*de2*cos(e2)*cos(e3) + 0.5*I5zz*de3*cos(e2)*cos(e3) - 0.5*I6zz*de2*cos(e2)*cos(e3) - 0.5*I6zz*de3*cos(e2)*cos(e3) + 0.5*I4xx*de2*sin(e2)*sin(e3) + 0.5*I4xx*de3*sin(e2)*sin(e3) + I5xx*de2*sin(e2)*sin(e3) + I5xx*de3*sin(e2)*sin(e3) - 0.5*I6xx*de2*sin(e2)*sin(e3) - 0.5*I6xx*de3*sin(e2)*sin(e3) - 0.5*I4yy*de2*sin(e2)*sin(e3) - 0.5*I4yy*de3*sin(e2)*sin(e3) + 0.5*I5yy*de2*sin(e2)*sin(e3) + 0.5*I5yy*de3*sin(e2)*sin(e3) + I6yy*de2*sin(e2)*sin(e3) + I6yy*de3*sin(e2)*sin(e3) + I4zz*de2*sin(e2)*sin(e3) + I4zz*de3*sin(e2)*sin(e3) - 0.5*I5zz*de2*sin(e2)*sin(e3) - 0.5*I5zz*de3*sin(e2)*sin(e3) + 0.5*I6zz*de2*sin(e2)*sin(e3) + 0.5*I6zz*de3*sin(e2)*sin(e3) - 1.0*de1*m4*x4*y4*cos(e2)^2 - 1.0*de1*m4*x4*y4*cos(e3)^2 - 2.0*de1*m4*x4*y4*cos(e4)^2 - 1.0*I5xx*de5*cos(e2)*cos(e3)*cos(e4) - 0.5*I6xx*de5*cos(e2)*cos(e3)*cos(e4) + I5yy*de5*cos(e2)*cos(e3)*cos(e4) - 1.0*I6yy*de5*cos(e2)*cos(e3)*cos(e4) - 0.5*I5zz*de5*cos(e2)*cos(e3)*cos(e4) + I6zz*de5*cos(e2)*cos(e3)*cos(e4) - 1.0*I6xx*de1*cos(e5)*cos(e6)*sin(e6) + I6yy*de1*cos(e5)*cos(e6)*sin(e6) + I5xx*de5*cos(e4)*sin(e2)*sin(e3) + 0.5*I6xx*de5*cos(e4)*sin(e2)*sin(e3) - 1.0*I5yy*de5*cos(e4)*sin(e2)*sin(e3) + I6yy*de5*cos(e4)*sin(e2)*sin(e3) + 0.5*I5zz*de5*cos(e4)*sin(e2)*sin(e3) - 1.0*I6zz*de5*cos(e4)*sin(e2)*sin(e3) - 0.5*de2*m4*x4^2*cos(e2)*cos(e3) - 0.5*de3*m4*x4^2*cos(e2)*cos(e3) - 1.5*de2*m6*x6^2*cos(e2)*cos(e3) - 1.5*de3*m6*x6^2*cos(e2)*cos(e3) - 1.5*de2*m4*y4^2*cos(e2)*cos(e3) - 1.5*de3*m4*y4^2*cos(e2)*cos(e3) - 0.5*de2*m5*y5^2*cos(e2)*cos(e3) - 0.5*de3*m5*y5^2*cos(e2)*cos(e3) - 1.5*de2*m5*z5^2*cos(e2)*cos(e3) - 1.5*de3*m5*z5^2*cos(e2)*cos(e3) - 0.5*de2*m6*z6^2*cos(e2)*cos(e3) - 0.5*de3*m6*z6^2*cos(e2)*cos(e3) + 0.5*de2*m4*x4^2*sin(e2)*sin(e3) + 0.5*de3*m4*x4^2*sin(e2)*sin(e3) + 1.5*de2*m6*x6^2*sin(e2)*sin(e3) + 1.5*de3*m6*x6^2*sin(e2)*sin(e3) + 1.5*de2*m4*y4^2*sin(e2)*sin(e3) + 1.5*de3*m4*y4^2*sin(e2)*sin(e3) + 0.5*de2*m5*y5^2*sin(e2)*sin(e3) + 0.5*de3*m5*y5^2*sin(e2)*sin(e3) + 1.5*de2*m5*z5^2*sin(e2)*sin(e3) + 1.5*de3*m5*z5^2*sin(e2)*sin(e3) + 0.5*de2*m6*z6^2*sin(e2)*sin(e3) + 0.5*de3*m6*z6^2*sin(e2)*sin(e3) + I4xx*de2*cos(e2)*cos(e3)*cos(e4)^2 + I4xx*de3*cos(e2)*cos(e3)*cos(e4)^2 + 0.5*I5xx*de2*cos(e2)*cos(e3)*cos(e5)^2 - 1.0*I6xx*de2*cos(e2)*cos(e3)*cos(e4)^2 + 0.5*I5xx*de3*cos(e2)*cos(e3)*cos(e5)^2 - 1.0*I6xx*de3*cos(e2)*cos(e3)*cos(e4)^2 - 1.5*I6xx*de2*cos(e2)*cos(e3)*cos(e6)^2 - 1.5*I6xx*de3*cos(e2)*cos(e3)*cos(e6)^2 - 1.0*I4yy*de2*cos(e2)*cos(e3)*cos(e4)^2 - 1.0*I4yy*de3*cos(e2)*cos(e3)*cos(e4)^2 + I5yy*de2*cos(e2)*cos(e3)*cos(e4)^2 - 0.5*I5yy*de2*cos(e2)*cos(e3)*cos(e5)^2 + I5yy*de3*cos(e2)*cos(e3)*cos(e4)^2 - 0.5*I5yy*de3*cos(e2)*cos(e3)*cos(e5)^2 + 0.5*I6yy*de2*cos(e2)*cos(e3)*cos(e5)^2 + 1.5*I6yy*de2*cos(e2)*cos(e3)*cos(e6)^2 + 0.5*I6yy*de3*cos(e2)*cos(e3)*cos(e5)^2 + 1.5*I6yy*de3*cos(e2)*cos(e3)*cos(e6)^2 - 1.0*I5zz*de2*cos(e2)*cos(e3)*cos(e4)^2 - 1.0*I5zz*de3*cos(e2)*cos(e3)*cos(e4)^2 + I6zz*de2*cos(e2)*cos(e3)*cos(e4)^2 - 0.5*I6zz*de2*cos(e2)*cos(e3)*cos(e5)^2 + I6zz*de3*cos(e2)*cos(e3)*cos(e4)^2 - 0.5*I6zz*de3*cos(e2)*cos(e3)*cos(e5)^2 + 0.5*a1*de4*m4*y4*cos(e4) - 0.5*a1*de4*m5*z5*cos(e4) - 1.0*I4xx*de1*cos(e2)^2*cos(e4)*sin(e4) - 1.0*I4xx*de1*cos(e3)^2*cos(e4)*sin(e4) + I6xx*de1*cos(e2)^2*cos(e4)*sin(e4) + I6xx*de1*cos(e3)^2*cos(e4)*sin(e4) + I5xx*de1*cos(e4)*cos(e5)^2*sin(e4) + I6xx*de1*cos(e4)*cos(e6)^2*sin(e4) + I4yy*de1*cos(e2)^2*cos(e4)*sin(e4) + I4yy*de1*cos(e3)^2*cos(e4)*sin(e4) - 1.0*I5yy*de1*cos(e2)^2*cos(e4)*sin(e4) - 1.0*I5yy*de1*cos(e3)^2*cos(e4)*sin(e4) - 1.0*I5yy*de1*cos(e4)*cos(e5)^2*sin(e4) + I6yy*de1*cos(e4)*cos(e5)^2*sin(e4) - 1.0*I6yy*de1*cos(e4)*cos(e6)^2*sin(e4) + I5zz*de1*cos(e2)^2*cos(e4)*sin(e4) + I5zz*de1*cos(e3)^2*cos(e4)*sin(e4) - 1.0*I6zz*de1*cos(e2)^2*cos(e4)*sin(e4) - 1.0*I6zz*de1*cos(e3)^2*cos(e4)*sin(e4) - 1.0*I6zz*de1*cos(e4)*cos(e5)^2*sin(e4) + 0.5*a1*de4*m4*x4*sin(e4) - 1.0*I4xx*de2*cos(e4)^2*sin(e2)*sin(e3) - 1.0*I4xx*de3*cos(e4)^2*sin(e2)*sin(e3) - 0.5*I5xx*de2*cos(e5)^2*sin(e2)*sin(e3) + I6xx*de2*cos(e4)^2*sin(e2)*sin(e3) - 0.5*I5xx*de3*cos(e5)^2*sin(e2)*sin(e3) + I6xx*de3*cos(e4)^2*sin(e2)*sin(e3) + 1.5*I6xx*de2*cos(e6)^2*sin(e2)*sin(e3) + 1.5*I6xx*de3*cos(e6)^2*sin(e2)*sin(e3) + I4yy*de2*cos(e4)^2*sin(e2)*sin(e3) + I4yy*de3*cos(e4)^2*sin(e2)*sin(e3) - 1.0*I5yy*de2*cos(e4)^2*sin(e2)*sin(e3) + 0.5*I5yy*de2*cos(e5)^2*sin(e2)*sin(e3) - 1.0*I5yy*de3*cos(e4)^2*sin(e2)*sin(e3) + 0.5*I5yy*de3*cos(e5)^2*sin(e2)*sin(e3) - 0.5*I6yy*de2*cos(e5)^2*sin(e2)*sin(e3) - 1.5*I6yy*de2*cos(e6)^2*sin(e2)*sin(e3) - 0.5*I6yy*de3*cos(e5)^2*sin(e2)*sin(e3) - 1.5*I6yy*de3*cos(e6)^2*sin(e2)*sin(e3) + I5zz*de2*cos(e4)^2*sin(e2)*sin(e3) + I5zz*de3*cos(e4)^2*sin(e2)*sin(e3) - 1.0*I6zz*de2*cos(e4)^2*sin(e2)*sin(e3) + 0.5*I6zz*de2*cos(e5)^2*sin(e2)*sin(e3) - 1.0*I6zz*de3*cos(e4)^2*sin(e2)*sin(e3) + 0.5*I6zz*de3*cos(e5)^2*sin(e2)*sin(e3) - 1.0*de1*m6*x6*y6*cos(e5) - 1.0*de1*m5*x5*z5*cos(e5) + de1*m5*y5*z5*sin(e5) + a3*de1*m4*x4*cos(e2)^2*sin(e4) + a3*de1*m4*x4*cos(e3)^2*sin(e4) - 1.0*I5xx*de2*cos(e4)^2*cos(e5)^2*sin(e2)*sin(e3) - 1.0*I5xx*de3*cos(e4)^2*cos(e5)^2*sin(e2)*sin(e3) - 1.0*I6xx*de2*cos(e4)^2*cos(e6)^2*sin(e2)*sin(e3) - 0.5*I6xx*de2*cos(e5)^2*cos(e6)^2*sin(e2)*sin(e3) - 1.0*I6xx*de3*cos(e4)^2*cos(e6)^2*sin(e2)*sin(e3) - 0.5*I6xx*de3*cos(e5)^2*cos(e6)^2*sin(e2)*sin(e3) + I5yy*de2*cos(e4)^2*cos(e5)^2*sin(e2)*sin(e3) + I5yy*de3*cos(e4)^2*cos(e5)^2*sin(e2)*sin(e3) - 1.0*I6yy*de2*cos(e4)^2*cos(e5)^2*sin(e2)*sin(e3) + I6yy*de2*cos(e4)^2*cos(e6)^2*sin(e2)*sin(e3) - 1.0*I6yy*de3*cos(e4)^2*cos(e5)^2*sin(e2)*sin(e3) + 0.5*I6yy*de2*cos(e5)^2*cos(e6)^2*sin(e2)*sin(e3) + I6yy*de3*cos(e4)^2*cos(e6)^2*sin(e2)*sin(e3) + 0.5*I6yy*de3*cos(e5)^2*cos(e6)^2*sin(e2)*sin(e3) + I6zz*de2*cos(e4)^2*cos(e5)^2*sin(e2)*sin(e3) + I6zz*de3*cos(e4)^2*cos(e5)^2*sin(e2)*sin(e3) + de1*m6*x6*y6*cos(e2)^2*cos(e5) + de1*m6*x6*y6*cos(e3)^2*cos(e5) + 2.0*de1*m6*x6*y6*cos(e4)^2*cos(e5) + 2.0*de1*m6*x6*y6*cos(e5)*cos(e6)^2 + de1*m5*x5*z5*cos(e2)^2*cos(e5) + de1*m5*x5*z5*cos(e3)^2*cos(e5) + 2.0*de1*m5*x5*z5*cos(e4)^2*cos(e5) - 1.0*de1*m5*y5*z5*cos(e2)^2*sin(e5) - 1.0*de1*m5*y5*z5*cos(e3)^2*sin(e5) - 2.0*de1*m5*y5*z5*cos(e4)^2*sin(e5) - 2.0*I5xx*de5*cos(e2)*cos(e5)*sin(e3)*sin(e5) - 2.0*I5xx*de5*cos(e3)*cos(e5)*sin(e2)*sin(e5) + I6xx*de6*cos(e2)*cos(e3)*sin(e4)*sin(e5) + 2.0*I6xx*de6*cos(e2)*cos(e6)*sin(e3)*sin(e6) + 2.0*I6xx*de6*cos(e3)*cos(e6)*sin(e2)*sin(e6) + 2.0*I5yy*de5*cos(e2)*cos(e5)*sin(e3)*sin(e5) + 2.0*I5yy*de5*cos(e3)*cos(e5)*sin(e2)*sin(e5) - 2.0*I6yy*de5*cos(e2)*cos(e5)*sin(e3)*sin(e5) - 2.0*I6yy*de5*cos(e3)*cos(e5)*sin(e2)*sin(e5) - 1.0*I6yy*de6*cos(e2)*cos(e3)*sin(e4)*sin(e5) - 2.0*I6yy*de6*cos(e2)*cos(e6)*sin(e3)*sin(e6) - 2.0*I6yy*de6*cos(e3)*cos(e6)*sin(e2)*sin(e6) + 2.0*I6zz*de5*cos(e2)*cos(e5)*sin(e3)*sin(e5) + 2.0*I6zz*de5*cos(e3)*cos(e5)*sin(e2)*sin(e5) - 0.5*I6zz*de6*cos(e2)*cos(e3)*sin(e4)*sin(e5) + 0.5*de5*m5*x5^2*cos(e2)*cos(e3)*cos(e4) - 1.5*de5*m5*y5^2*cos(e2)*cos(e3)*cos(e4) + 0.5*de5*m6*y6^2*cos(e2)*cos(e3)*cos(e4) - 1.5*de5*m6*z6^2*cos(e2)*cos(e3)*cos(e4) - 1.0*I6xx*de6*sin(e2)*sin(e3)*sin(e4)*sin(e5) + I6yy*de6*sin(e2)*sin(e3)*sin(e4)*sin(e5) + 0.5*I6zz*de6*sin(e2)*sin(e3)*sin(e4)*sin(e5) + de1*m6*x6^2*cos(e5)*cos(e6)*sin(e6) + 2.0*de1*m4*x4*y4*cos(e2)^2*cos(e3)^2 + 2.0*de1*m4*x4*y4*cos(e2)^2*cos(e4)^2 + 2.0*de1*m4*x4*y4*cos(e3)^2*cos(e4)^2 - 1.0*de1*m6*y6^2*cos(e5)*cos(e6)*sin(e6) - 0.5*de5*m5*x5^2*cos(e4)*sin(e2)*sin(e3) + 1.5*de5*m5*y5^2*cos(e4)*sin(e2)*sin(e3) - 0.5*de5*m6*y6^2*cos(e4)*sin(e2)*sin(e3) + 1.5*de5*m6*z6^2*cos(e4)*sin(e2)*sin(e3) + 2.0*I5xx*de5*cos(e2)*cos(e3)*cos(e4)*cos(e5)^2 - 0.5*I6xx*de5*cos(e2)*cos(e3)*cos(e4)*cos(e6)^2 - 2.0*I5yy*de5*cos(e2)*cos(e3)*cos(e4)*cos(e5)^2 + 2.0*I6yy*de5*cos(e2)*cos(e3)*cos(e4)*cos(e5)^2 + 0.5*I6yy*de5*cos(e2)*cos(e3)*cos(e4)*cos(e6)^2 - 2.0*I6zz*de5*cos(e2)*cos(e3)*cos(e4)*cos(e5)^2 - 1.5*a2*de2*m4*x4*cos(e2)*cos(e4) + a2*de1*m4*y4*cos(e3)*cos(e4) + 0.5*a1*de5*m5*y5*cos(e4)*cos(e5) + 0.5*a1*de4*m6*y6*cos(e4)*cos(e6) - 1.0*a2*de1*m5*z5*cos(e3)*cos(e4) + 0.5*a1*de5*m6*z6*cos(e4)*cos(e5) + I6xx*de1*cos(e2)^2*cos(e5)*cos(e6)*sin(e6) + I6xx*de1*cos(e3)^2*cos(e5)*cos(e6)*sin(e6) + 2.0*I6xx*de1*cos(e4)^2*cos(e5)*cos(e6)*sin(e6) - 1.0*I6yy*de1*cos(e2)^2*cos(e5)*cos(e6)*sin(e6) - 1.0*I6yy*de1*cos(e3)^2*cos(e5)*cos(e6)*sin(e6) - 2.0*I6yy*de1*cos(e4)^2*cos(e5)*cos(e6)*sin(e6) + a2*de1*m4*x4*cos(e3)*sin(e4) + 0.5*a1*de4*m5*x5*cos(e5)*sin(e4) + 0.5*a1*de5*m5*x5*cos(e4)*sin(e5) + 0.5*a1*de4*m6*x6*cos(e4)*sin(e6) + 0.5*a1*de6*m6*x6*cos(e6)*sin(e4) + 1.5*a2*de2*m4*y4*cos(e2)*sin(e4) + 0.5*a2*de4*m4*y4*cos(e4)*sin(e2) - 1.5*a2*de2*m5*z5*cos(e2)*sin(e4) - 0.5*a2*de4*m5*z5*cos(e4)*sin(e2) - 2.0*I5xx*de5*cos(e4)*cos(e5)^2*sin(e2)*sin(e3) + 0.5*I6xx*de5*cos(e4)*cos(e6)^2*sin(e2)*sin(e3) + 2.0*I5yy*de5*cos(e4)*cos(e5)^2*sin(e2)*sin(e3) - 2.0*I6yy*de5*cos(e4)*cos(e5)^2*sin(e2)*sin(e3) - 0.5*I6yy*de5*cos(e4)*cos(e6)^2*sin(e2)*sin(e3) + 2.0*I6zz*de5*cos(e4)*cos(e5)^2*sin(e2)*sin(e3) + 0.5*a2*de4*m4*x4*sin(e2)*sin(e4) - 0.5*a1*de4*m5*y5*sin(e4)*sin(e5) - 0.5*a1*de6*m6*y6*sin(e4)*sin(e6) - 0.5*a1*de4*m6*z6*sin(e4)*sin(e5) - 1.0*de2*m4*x4^2*cos(e2)*cos(e3)*cos(e4)^2 - 1.0*de3*m4*x4^2*cos(e2)*cos(e3)*cos(e4)^2 - 0.5*de2*m5*x5^2*cos(e2)*cos(e3)*cos(e5)^2 + de2*m6*x6^2*cos(e2)*cos(e3)*cos(e4)^2 - 0.5*de3*m5*x5^2*cos(e2)*cos(e3)*cos(e5)^2 + de3*m6*x6^2*cos(e2)*cos(e3)*cos(e4)^2 + 1.5*de2*m6*x6^2*cos(e2)*cos(e3)*cos(e6)^2 + 1.5*de3*m6*x6^2*cos(e2)*cos(e3)*cos(e6)^2 + de2*m4*y4^2*cos(e2)*cos(e3)*cos(e4)^2 + de3*m4*y4^2*cos(e2)*cos(e3)*cos(e4)^2 - 1.0*de2*m5*y5^2*cos(e2)*cos(e3)*cos(e4)^2 + 0.5*de2*m5*y5^2*cos(e2)*cos(e3)*cos(e5)^2 - 1.0*de3*m5*y5^2*cos(e2)*cos(e3)*cos(e4)^2 + 0.5*de3*m5*y5^2*cos(e2)*cos(e3)*cos(e5)^2 - 0.5*de2*m6*y6^2*cos(e2)*cos(e3)*cos(e5)^2 - 1.5*de2*m6*y6^2*cos(e2)*cos(e3)*cos(e6)^2 - 0.5*de3*m6*y6^2*cos(e2)*cos(e3)*cos(e5)^2 - 1.5*de3*m6*y6^2*cos(e2)*cos(e3)*cos(e6)^2 - 2.0*de5*m5*x5*y5*cos(e2)*sin(e3) - 2.0*de5*m5*x5*y5*cos(e3)*sin(e2) + 2.0*de6*m6*x6*y6*cos(e2)*sin(e3) + 2.0*de6*m6*x6*y6*cos(e3)*sin(e2) + de2*m5*z5^2*cos(e2)*cos(e3)*cos(e4)^2 + de3*m5*z5^2*cos(e2)*cos(e3)*cos(e4)^2 - 1.0*de2*m6*z6^2*cos(e2)*cos(e3)*cos(e4)^2 + 0.5*de2*m6*z6^2*cos(e2)*cos(e3)*cos(e5)^2 - 1.0*de3*m6*z6^2*cos(e2)*cos(e3)*cos(e4)^2 + 0.5*de3*m6*z6^2*cos(e2)*cos(e3)*cos(e5)^2 - 1.0*de1*m6*y6*z6*cos(e6)*sin(e5) + de1*m4*x4^2*cos(e2)^2*cos(e4)*sin(e4) + de1*m4*x4^2*cos(e3)^2*cos(e4)*sin(e4) - 1.0*de1*m6*x6^2*cos(e2)^2*cos(e4)*sin(e4) - 1.0*de1*m5*x5^2*cos(e4)*cos(e5)^2*sin(e4) - 1.0*de1*m6*x6^2*cos(e3)^2*cos(e4)*sin(e4) - 1.0*de1*m6*x6^2*cos(e4)*cos(e6)^2*sin(e4) - 1.0*de1*m4*y4^2*cos(e2)^2*cos(e4)*sin(e4) - 1.0*de1*m4*y4^2*cos(e3)^2*cos(e4)*sin(e4) + de1*m5*y5^2*cos(e2)^2*cos(e4)*sin(e4) + de1*m5*y5^2*cos(e3)^2*cos(e4)*sin(e4) + de1*m5*y5^2*cos(e4)*cos(e5)^2*sin(e4) - 1.0*de1*m6*y6^2*cos(e4)*cos(e5)^2*sin(e4) + de1*m6*y6^2*cos(e4)*cos(e6)^2*sin(e4) - 1.0*de1*m5*z5^2*cos(e2)^2*cos(e4)*sin(e4) - 1.0*de1*m5*z5^2*cos(e3)^2*cos(e4)*sin(e4) + de1*m6*z6^2*cos(e2)^2*cos(e4)*sin(e4) + de1*m6*z6^2*cos(e3)^2*cos(e4)*sin(e4) + de1*m6*z6^2*cos(e4)*cos(e5)^2*sin(e4) - 1.0*de1*m6*x6*z6*sin(e5)*sin(e6) + de2*m4*x4^2*cos(e4)^2*sin(e2)*sin(e3) + de3*m4*x4^2*cos(e4)^2*sin(e2)*sin(e3) + 0.5*de2*m5*x5^2*cos(e5)^2*sin(e2)*sin(e3) - 1.0*de2*m6*x6^2*cos(e4)^2*sin(e2)*sin(e3) + 0.5*de3*m5*x5^2*cos(e5)^2*sin(e2)*sin(e3) - 1.0*de3*m6*x6^2*cos(e4)^2*sin(e2)*sin(e3) - 1.5*de2*m6*x6^2*cos(e6)^2*sin(e2)*sin(e3) - 1.5*de3*m6*x6^2*cos(e6)^2*sin(e2)*sin(e3) - 1.0*de2*m4*y4^2*cos(e4)^2*sin(e2)*sin(e3) - 1.0*de3*m4*y4^2*cos(e4)^2*sin(e2)*sin(e3) + de2*m5*y5^2*cos(e4)^2*sin(e2)*sin(e3) - 0.5*de2*m5*y5^2*cos(e5)^2*sin(e2)*sin(e3) + de3*m5*y5^2*cos(e4)^2*sin(e2)*sin(e3) - 0.5*de3*m5*y5^2*cos(e5)^2*sin(e2)*sin(e3) + 0.5*de2*m6*y6^2*cos(e5)^2*sin(e2)*sin(e3) + 1.5*de2*m6*y6^2*cos(e6)^2*sin(e2)*sin(e3) + 0.5*de3*m6*y6^2*cos(e5)^2*sin(e2)*sin(e3) + 1.5*de3*m6*y6^2*cos(e6)^2*sin(e2)*sin(e3) - 1.0*de2*m5*z5^2*cos(e4)^2*sin(e2)*sin(e3) - 1.0*de3*m5*z5^2*cos(e4)^2*sin(e2)*sin(e3) + de2*m6*z6^2*cos(e4)^2*sin(e2)*sin(e3) - 0.5*de2*m6*z6^2*cos(e5)^2*sin(e2)*sin(e3) + de3*m6*z6^2*cos(e4)^2*sin(e2)*sin(e3) - 0.5*de3*m6*z6^2*cos(e5)^2*sin(e2)*sin(e3) + I5xx*de2*cos(e2)*cos(e3)*cos(e4)^2*cos(e5)^2 + I5xx*de3*cos(e2)*cos(e3)*cos(e4)^2*cos(e5)^2 + I6xx*de2*cos(e2)*cos(e3)*cos(e4)^2*cos(e6)^2 + 0.5*I6xx*de2*cos(e2)*cos(e3)*cos(e5)^2*cos(e6)^2 + I6xx*de3*cos(e2)*cos(e3)*cos(e4)^2*cos(e6)^2 + 0.5*I6xx*de3*cos(e2)*cos(e3)*cos(e5)^2*cos(e6)^2 - 1.0*I5yy*de2*cos(e2)*cos(e3)*cos(e4)^2*cos(e5)^2 - 1.0*I5yy*de3*cos(e2)*cos(e3)*cos(e4)^2*cos(e5)^2 + I6yy*de2*cos(e2)*cos(e3)*cos(e4)^2*cos(e5)^2 - 1.0*I6yy*de2*cos(e2)*cos(e3)*cos(e4)^2*cos(e6)^2 + I6yy*de3*cos(e2)*cos(e3)*cos(e4)^2*cos(e5)^2 - 0.5*I6yy*de2*cos(e2)*cos(e3)*cos(e5)^2*cos(e6)^2 - 1.0*I6yy*de3*cos(e2)*cos(e3)*cos(e4)^2*cos(e6)^2 - 0.5*I6yy*de3*cos(e2)*cos(e3)*cos(e5)^2*cos(e6)^2 - 1.0*I6zz*de2*cos(e2)*cos(e3)*cos(e4)^2*cos(e5)^2 - 1.0*I6zz*de3*cos(e2)*cos(e3)*cos(e4)^2*cos(e5)^2 + a3*de1*m4*y4*cos(e2)^2*cos(e4) + a3*de1*m4*y4*cos(e3)^2*cos(e4) - 1.0*a3*de1*m5*z5*cos(e2)^2*cos(e4) - 1.0*a3*de1*m5*z5*cos(e3)^2*cos(e4) + 2.0*I4xx*de1*cos(e2)^2*cos(e3)^2*cos(e4)*sin(e4) - 2.0*I6xx*de1*cos(e2)^2*cos(e3)^2*cos(e4)*sin(e4) - 1.0*I5xx*de1*cos(e2)^2*cos(e4)*cos(e5)^2*sin(e4) - 1.0*I5xx*de1*cos(e3)^2*cos(e4)*cos(e5)^2*sin(e4) - 1.0*I6xx*de1*cos(e2)^2*cos(e4)*cos(e6)^2*sin(e4) - 1.0*I6xx*de1*cos(e3)^2*cos(e4)*cos(e6)^2*sin(e4) + I6xx*de1*cos(e4)*cos(e5)^2*cos(e6)^2*sin(e4) - 2.0*I4yy*de1*cos(e2)^2*cos(e3)^2*cos(e4)*sin(e4) + 2.0*I5yy*de1*cos(e2)^2*cos(e3)^2*cos(e4)*sin(e4) + I5yy*de1*cos(e2)^2*cos(e4)*cos(e5)^2*sin(e4) + I5yy*de1*cos(e3)^2*cos(e4)*cos(e5)^2*sin(e4) - 1.0*I6yy*de1*cos(e2)^2*cos(e4)*cos(e5)^2*sin(e4) + I6yy*de1*cos(e2)^2*cos(e4)*cos(e6)^2*sin(e4) - 1.0*I6yy*de1*cos(e3)^2*cos(e4)*cos(e5)^2*sin(e4) + I6yy*de1*cos(e3)^2*cos(e4)*cos(e6)^2*sin(e4) - 1.0*I6yy*de1*cos(e4)*cos(e5)^2*cos(e6)^2*sin(e4) - 2.0*I5zz*de1*cos(e2)^2*cos(e3)^2*cos(e4)*sin(e4) + 2.0*I6zz*de1*cos(e2)^2*cos(e3)^2*cos(e4)*sin(e4) + I6zz*de1*cos(e2)^2*cos(e4)*cos(e5)^2*sin(e4) + I6zz*de1*cos(e3)^2*cos(e4)*cos(e5)^2*sin(e4) + de2*m5*x5^2*cos(e4)^2*cos(e5)^2*sin(e2)*sin(e3) + de3*m5*x5^2*cos(e4)^2*cos(e5)^2*sin(e2)*sin(e3) + de2*m6*x6^2*cos(e4)^2*cos(e6)^2*sin(e2)*sin(e3) + 0.5*de2*m6*x6^2*cos(e5)^2*cos(e6)^2*sin(e2)*sin(e3) + de3*m6*x6^2*cos(e4)^2*cos(e6)^2*sin(e2)*sin(e3) + 0.5*de3*m6*x6^2*cos(e5)^2*cos(e6)^2*sin(e2)*sin(e3) - 1.0*de2*m5*y5^2*cos(e4)^2*cos(e5)^2*sin(e2)*sin(e3) - 1.0*de3*m5*y5^2*cos(e4)^2*cos(e5)^2*sin(e2)*sin(e3) + de2*m6*y6^2*cos(e4)^2*cos(e5)^2*sin(e2)*sin(e3) - 1.0*de2*m6*y6^2*cos(e4)^2*cos(e6)^2*sin(e2)*sin(e3) + de3*m6*y6^2*cos(e4)^2*cos(e5)^2*sin(e2)*sin(e3) - 0.5*de2*m6*y6^2*cos(e5)^2*cos(e6)^2*sin(e2)*sin(e3) - 1.0*de3*m6*y6^2*cos(e4)^2*cos(e6)^2*sin(e2)*sin(e3) - 0.5*de3*m6*y6^2*cos(e5)^2*cos(e6)^2*sin(e2)*sin(e3) - 1.0*de2*m6*z6^2*cos(e4)^2*cos(e5)^2*sin(e2)*sin(e3) - 1.0*de3*m6*z6^2*cos(e4)^2*cos(e5)^2*sin(e2)*sin(e3) + I6xx*de2*cos(e2)*cos(e3)*cos(e4)^2*cos(e5)^2*cos(e6)^2 + I6xx*de3*cos(e2)*cos(e3)*cos(e4)^2*cos(e5)^2*cos(e6)^2 - 1.0*I6yy*de2*cos(e2)*cos(e3)*cos(e4)^2*cos(e5)^2*cos(e6)^2 - 1.0*I6yy*de3*cos(e2)*cos(e3)*cos(e4)^2*cos(e5)^2*cos(e6)^2 - 1.5*I5xx*de2*cos(e2)*cos(e4)*cos(e5)*sin(e3)*sin(e5) - 1.5*I5xx*de2*cos(e3)*cos(e4)*cos(e5)*sin(e2)*sin(e5) - 1.5*I5xx*de3*cos(e2)*cos(e4)*cos(e5)*sin(e3)*sin(e5) - 1.5*I5xx*de3*cos(e3)*cos(e4)*cos(e5)*sin(e2)*sin(e5) - 0.5*I5xx*de4*cos(e2)*cos(e3)*cos(e5)*sin(e4)*sin(e5) + 1.5*I5yy*de2*cos(e2)*cos(e4)*cos(e5)*sin(e3)*sin(e5) + 1.5*I5yy*de2*cos(e3)*cos(e4)*cos(e5)*sin(e2)*sin(e5) + 1.5*I5yy*de3*cos(e2)*cos(e4)*cos(e5)*sin(e3)*sin(e5) + 1.5*I5yy*de3*cos(e3)*cos(e4)*cos(e5)*sin(e2)*sin(e5) - 1.5*I6yy*de2*cos(e2)*cos(e4)*cos(e5)*sin(e3)*sin(e5) - 1.5*I6yy*de2*cos(e3)*cos(e4)*cos(e5)*sin(e2)*sin(e5) + 0.5*I5yy*de4*cos(e2)*cos(e3)*cos(e5)*sin(e4)*sin(e5) - 1.5*I6yy*de3*cos(e2)*cos(e4)*cos(e5)*sin(e3)*sin(e5) - 1.5*I6yy*de3*cos(e3)*cos(e4)*cos(e5)*sin(e2)*sin(e5) - 0.5*I6yy*de4*cos(e2)*cos(e3)*cos(e5)*sin(e4)*sin(e5);
C412 = + 1.5*I6zz*de2*cos(e2)*cos(e4)*cos(e5)*sin(e3)*sin(e5) + 1.5*I6zz*de2*cos(e3)*cos(e4)*cos(e5)*sin(e2)*sin(e5) + 1.5*I6zz*de3*cos(e2)*cos(e4)*cos(e5)*sin(e3)*sin(e5) + 1.5*I6zz*de3*cos(e3)*cos(e4)*cos(e5)*sin(e2)*sin(e5) + 0.5*I6zz*de4*cos(e2)*cos(e3)*cos(e5)*sin(e4)*sin(e5) - 2.0*a3*de1*m4*y4*cos(e2)^2*cos(e3)^2*cos(e4) + 2.0*a3*de1*m5*z5*cos(e2)^2*cos(e3)^2*cos(e4) + 2.0*I5xx*de1*cos(e2)^2*cos(e3)^2*cos(e4)*cos(e5)^2*sin(e4) + 2.0*I6xx*de1*cos(e2)^2*cos(e3)^2*cos(e4)*cos(e6)^2*sin(e4) - 1.0*I6xx*de1*cos(e2)^2*cos(e4)*cos(e5)^2*cos(e6)^2*sin(e4) - 1.0*I6xx*de1*cos(e3)^2*cos(e4)*cos(e5)^2*cos(e6)^2*sin(e4) - 2.0*I5yy*de1*cos(e2)^2*cos(e3)^2*cos(e4)*cos(e5)^2*sin(e4) + 2.0*I6yy*de1*cos(e2)^2*cos(e3)^2*cos(e4)*cos(e5)^2*sin(e4) - 2.0*I6yy*de1*cos(e2)^2*cos(e3)^2*cos(e4)*cos(e6)^2*sin(e4) + I6yy*de1*cos(e2)^2*cos(e4)*cos(e5)^2*cos(e6)^2*sin(e4) + I6yy*de1*cos(e3)^2*cos(e4)*cos(e5)^2*cos(e6)^2*sin(e4) - 2.0*I6zz*de1*cos(e2)^2*cos(e3)^2*cos(e4)*cos(e5)^2*sin(e4) + I5xx*de1*cos(e2)*cos(e5)*sin(e2)*sin(e4)*sin(e5) + I5xx*de1*cos(e3)*cos(e5)*sin(e3)*sin(e4)*sin(e5) - 1.0*I5yy*de1*cos(e2)*cos(e5)*sin(e2)*sin(e4)*sin(e5) + I6yy*de1*cos(e2)*cos(e5)*sin(e2)*sin(e4)*sin(e5) - 1.0*I5yy*de1*cos(e3)*cos(e5)*sin(e3)*sin(e4)*sin(e5) + I6yy*de1*cos(e3)*cos(e5)*sin(e3)*sin(e4)*sin(e5) - 1.0*I6zz*de1*cos(e2)*cos(e5)*sin(e2)*sin(e4)*sin(e5) - 1.0*I6zz*de1*cos(e3)*cos(e5)*sin(e3)*sin(e4)*sin(e5) - 2.0*a3*de1*m4*x4*cos(e2)^2*cos(e3)^2*sin(e4) - 1.0*I6xx*de2*cos(e4)^2*cos(e5)^2*cos(e6)^2*sin(e2)*sin(e3) - 1.0*I6xx*de3*cos(e4)^2*cos(e5)^2*cos(e6)^2*sin(e2)*sin(e3) + I6yy*de2*cos(e4)^2*cos(e5)^2*cos(e6)^2*sin(e2)*sin(e3) + I6yy*de3*cos(e4)^2*cos(e5)^2*cos(e6)^2*sin(e2)*sin(e3) + 0.5*I5xx*de4*cos(e5)*sin(e2)*sin(e3)*sin(e4)*sin(e5) - 0.5*I5yy*de4*cos(e5)*sin(e2)*sin(e3)*sin(e4)*sin(e5) + 0.5*I6yy*de4*cos(e5)*sin(e2)*sin(e3)*sin(e4)*sin(e5) - 0.5*I6zz*de4*cos(e5)*sin(e2)*sin(e3)*sin(e4)*sin(e5) - 2.0*de1*m6*x6*y6*cos(e2)^2*cos(e3)^2*cos(e5) - 2.0*de1*m6*x6*y6*cos(e2)^2*cos(e4)^2*cos(e5) - 2.0*de1*m6*x6*y6*cos(e3)^2*cos(e4)^2*cos(e5) - 2.0*de1*m6*x6*y6*cos(e2)^2*cos(e5)*cos(e6)^2 - 2.0*de1*m6*x6*y6*cos(e3)^2*cos(e5)*cos(e6)^2 - 4.0*de1*m6*x6*y6*cos(e4)^2*cos(e5)*cos(e6)^2 - 2.0*de1*m5*x5*z5*cos(e2)^2*cos(e3)^2*cos(e5) - 2.0*de1*m5*x5*z5*cos(e2)^2*cos(e4)^2*cos(e5) - 2.0*de1*m5*x5*z5*cos(e3)^2*cos(e4)^2*cos(e5) + 2.0*de5*m5*x5^2*cos(e2)*cos(e5)*sin(e3)*sin(e5) + 2.0*de5*m5*x5^2*cos(e3)*cos(e5)*sin(e2)*sin(e5) - 1.5*de6*m6*x6^2*cos(e2)*cos(e3)*sin(e4)*sin(e5) - 2.0*de6*m6*x6^2*cos(e2)*cos(e6)*sin(e3)*sin(e6) - 2.0*de6*m6*x6^2*cos(e3)*cos(e6)*sin(e2)*sin(e6) - 2.0*de5*m5*y5^2*cos(e2)*cos(e5)*sin(e3)*sin(e5) - 2.0*de5*m5*y5^2*cos(e3)*cos(e5)*sin(e2)*sin(e5) + 2.0*de5*m6*y6^2*cos(e2)*cos(e5)*sin(e3)*sin(e5) + 2.0*de5*m6*y6^2*cos(e3)*cos(e5)*sin(e2)*sin(e5) + 0.5*de6*m6*y6^2*cos(e2)*cos(e3)*sin(e4)*sin(e5) + 2.0*de6*m6*y6^2*cos(e2)*cos(e6)*sin(e3)*sin(e6) + 2.0*de6*m6*y6^2*cos(e3)*cos(e6)*sin(e2)*sin(e6) - 2.0*de5*m6*z6^2*cos(e2)*cos(e5)*sin(e3)*sin(e5) - 2.0*de5*m6*z6^2*cos(e3)*cos(e5)*sin(e2)*sin(e5) + 2.0*de1*m5*y5*z5*cos(e2)^2*cos(e3)^2*sin(e5) + 2.0*de1*m5*y5*z5*cos(e2)^2*cos(e4)^2*sin(e5) + 2.0*de1*m5*y5*z5*cos(e3)^2*cos(e4)^2*sin(e5) - 1.5*a3*de2*m4*x4*cos(e2)*cos(e3)*cos(e4) - 1.5*a3*de3*m4*x4*cos(e2)*cos(e3)*cos(e4) - 1.5*a2*de2*m5*x5*cos(e2)*cos(e4)*cos(e5) + a2*de1*m6*y6*cos(e3)*cos(e4)*cos(e6) + 0.5*a1*de6*m6*y6*cos(e4)*cos(e5)*cos(e6) + 0.5*d4*de4*m4*y4*cos(e2)*cos(e3)*cos(e4) - 0.5*d4*de4*m5*z5*cos(e2)*cos(e3)*cos(e4) + 1.5*de6*m6*x6^2*sin(e2)*sin(e3)*sin(e4)*sin(e5) - 0.5*de6*m6*y6^2*sin(e2)*sin(e3)*sin(e4)*sin(e5) + a2*de1*m5*x5*cos(e3)*cos(e5)*sin(e4) + a2*de1*m6*x6*cos(e3)*cos(e4)*sin(e6) + 0.5*a1*de4*m6*x6*cos(e5)*cos(e6)*sin(e4) + 0.5*a1*de5*m6*x6*cos(e4)*cos(e6)*sin(e5) + 0.5*a1*de6*m6*x6*cos(e4)*cos(e5)*sin(e6) + a1*de1*m4*y4*cos(e2)*cos(e4)*sin(e3) + a1*de1*m4*y4*cos(e3)*cos(e4)*sin(e2) + 1.5*a3*de2*m4*y4*cos(e2)*cos(e3)*sin(e4) + 1.5*a3*de3*m4*y4*cos(e2)*cos(e3)*sin(e4) + 0.5*a3*de4*m4*y4*cos(e2)*cos(e4)*sin(e3) + 0.5*a3*de4*m4*y4*cos(e3)*cos(e4)*sin(e2) + 1.5*a2*de2*m5*y5*cos(e2)*cos(e4)*sin(e5) + 1.5*a2*de2*m6*y6*cos(e2)*cos(e6)*sin(e4) + 0.5*a2*de5*m5*y5*cos(e4)*cos(e5)*sin(e2) + 0.5*a2*de4*m6*y6*cos(e4)*cos(e6)*sin(e2) - 1.0*a1*de1*m5*z5*cos(e2)*cos(e4)*sin(e3) - 1.0*a1*de1*m5*z5*cos(e3)*cos(e4)*sin(e2) - 1.5*a3*de2*m5*z5*cos(e2)*cos(e3)*sin(e4) - 1.5*a3*de3*m5*z5*cos(e2)*cos(e3)*sin(e4) - 0.5*a3*de4*m5*z5*cos(e2)*cos(e4)*sin(e3) - 0.5*a3*de4*m5*z5*cos(e3)*cos(e4)*sin(e2) + 1.5*a2*de2*m6*z6*cos(e2)*cos(e4)*sin(e5) + 0.5*a2*de5*m6*z6*cos(e4)*cos(e5)*sin(e2) + 1.5*d4*de2*m4*x4*cos(e2)*cos(e4)*sin(e3) + 1.5*d4*de2*m4*x4*cos(e3)*cos(e4)*sin(e2) + 1.5*d4*de3*m4*x4*cos(e2)*cos(e4)*sin(e3) + 1.5*d4*de3*m4*x4*cos(e3)*cos(e4)*sin(e2) + 0.5*d4*de4*m4*x4*cos(e2)*cos(e3)*sin(e4) - 2.0*I6xx*de5*cos(e2)*cos(e5)*cos(e6)^2*sin(e3)*sin(e5) - 2.0*I6xx*de5*cos(e3)*cos(e5)*cos(e6)^2*sin(e2)*sin(e5) - 2.0*I6xx*de6*cos(e2)*cos(e3)*cos(e6)^2*sin(e4)*sin(e5) - 2.0*I6xx*de6*cos(e2)*cos(e5)^2*cos(e6)*sin(e3)*sin(e6) - 2.0*I6xx*de6*cos(e3)*cos(e5)^2*cos(e6)*sin(e2)*sin(e6) + 2.0*I6yy*de5*cos(e2)*cos(e5)*cos(e6)^2*sin(e3)*sin(e5) + 2.0*I6yy*de5*cos(e3)*cos(e5)*cos(e6)^2*sin(e2)*sin(e5) + 2.0*I6yy*de6*cos(e2)*cos(e3)*cos(e6)^2*sin(e4)*sin(e5) + 2.0*I6yy*de6*cos(e2)*cos(e5)^2*cos(e6)*sin(e3)*sin(e6) + 2.0*I6yy*de6*cos(e3)*cos(e5)^2*cos(e6)*sin(e2)*sin(e6) - 1.0*d4*de1*m4*y4*cos(e2)*cos(e4)*sin(e2) - 1.0*d4*de1*m4*y4*cos(e3)*cos(e4)*sin(e3) + d4*de1*m5*z5*cos(e2)*cos(e4)*sin(e2) + d4*de1*m5*z5*cos(e3)*cos(e4)*sin(e3) + 0.5*de4*m4*y4*z4*cos(e2)*cos(e3)*cos(e4) + a1*de1*m4*x4*cos(e2)*sin(e3)*sin(e4) + a1*de1*m4*x4*cos(e3)*sin(e2)*sin(e4) + 1.5*a3*de2*m4*x4*cos(e4)*sin(e2)*sin(e3) + 1.5*a3*de3*m4*x4*cos(e4)*sin(e2)*sin(e3) + 0.5*a3*de4*m4*x4*cos(e2)*sin(e3)*sin(e4) + 0.5*a3*de4*m4*x4*cos(e3)*sin(e2)*sin(e4) + 0.5*a2*de4*m5*x5*cos(e5)*sin(e2)*sin(e4) + 1.5*a2*de2*m6*x6*cos(e2)*sin(e4)*sin(e6) + 0.5*a2*de5*m5*x5*cos(e4)*sin(e2)*sin(e5) + 0.5*a2*de4*m6*x6*cos(e4)*sin(e2)*sin(e6) + 0.5*a2*de6*m6*x6*cos(e6)*sin(e2)*sin(e4) - 1.0*a2*de1*m5*y5*cos(e3)*sin(e4)*sin(e5) - 0.5*a1*de4*m6*y6*cos(e5)*sin(e4)*sin(e6) - 0.5*a1*de5*m6*y6*cos(e4)*sin(e5)*sin(e6) - 1.0*a2*de1*m6*z6*cos(e3)*sin(e4)*sin(e5) - 1.0*d4*de1*m4*x4*cos(e2)*sin(e2)*sin(e4) - 1.0*d4*de1*m4*x4*cos(e3)*sin(e3)*sin(e4) - 1.5*d4*de2*m4*y4*cos(e2)*sin(e3)*sin(e4) - 1.5*d4*de2*m4*y4*cos(e3)*sin(e2)*sin(e4) - 1.5*d4*de3*m4*y4*cos(e2)*sin(e3)*sin(e4) - 1.5*d4*de3*m4*y4*cos(e3)*sin(e2)*sin(e4) - 0.5*d4*de4*m4*y4*cos(e4)*sin(e2)*sin(e3) + 1.5*d4*de2*m5*z5*cos(e2)*sin(e3)*sin(e4) + 1.5*d4*de2*m5*z5*cos(e3)*sin(e2)*sin(e4) + 1.5*d4*de3*m5*z5*cos(e2)*sin(e3)*sin(e4) + 1.5*d4*de3*m5*z5*cos(e3)*sin(e2)*sin(e4) + 0.5*d4*de4*m5*z5*cos(e4)*sin(e2)*sin(e3) - 2.0*de5*m5*x5^2*cos(e2)*cos(e3)*cos(e4)*cos(e5)^2 + 0.5*de5*m6*x6^2*cos(e2)*cos(e3)*cos(e4)*cos(e6)^2 + 2.0*de5*m5*y5^2*cos(e2)*cos(e3)*cos(e4)*cos(e5)^2 - 2.0*de5*m6*y6^2*cos(e2)*cos(e3)*cos(e4)*cos(e5)^2 - 0.5*de5*m6*y6^2*cos(e2)*cos(e3)*cos(e4)*cos(e6)^2 - 1.5*de2*m5*x5*y5*cos(e2)*cos(e4)*sin(e3) - 1.5*de2*m5*x5*y5*cos(e3)*cos(e4)*sin(e2) - 1.5*de3*m5*x5*y5*cos(e2)*cos(e4)*sin(e3) - 1.5*de3*m5*x5*y5*cos(e3)*cos(e4)*sin(e2) - 0.5*de4*m5*x5*y5*cos(e2)*cos(e3)*sin(e4) + 2.0*de5*m6*z6^2*cos(e2)*cos(e3)*cos(e4)*cos(e5)^2 + 1.5*de2*m4*x4*z4*cos(e2)*cos(e4)*sin(e3) + 1.5*de2*m4*x4*z4*cos(e3)*cos(e4)*sin(e2) + 1.5*de3*m4*x4*z4*cos(e2)*cos(e4)*sin(e3) + 1.5*de3*m4*x4*z4*cos(e3)*cos(e4)*sin(e2) + 0.5*de4*m4*x4*z4*cos(e2)*cos(e3)*sin(e4) - 2.0*de5*m6*x6*z6*cos(e2)*cos(e6)*sin(e3) - 2.0*de5*m6*x6*z6*cos(e3)*cos(e6)*sin(e2) - 1.0*de1*m4*y4*z4*cos(e2)*cos(e4)*sin(e2) - 1.0*de1*m4*y4*z4*cos(e3)*cos(e4)*sin(e3) - 1.5*a3*de2*m4*y4*sin(e2)*sin(e3)*sin(e4) - 1.5*a3*de3*m4*y4*sin(e2)*sin(e3)*sin(e4) - 0.5*a2*de4*m5*y5*sin(e2)*sin(e4)*sin(e5) - 0.5*a2*de6*m6*y6*sin(e2)*sin(e4)*sin(e6) + 1.5*a3*de2*m5*z5*sin(e2)*sin(e3)*sin(e4) + 1.5*a3*de3*m5*z5*sin(e2)*sin(e3)*sin(e4) - 0.5*a2*de4*m6*z6*sin(e2)*sin(e4)*sin(e5) - 0.5*d4*de4*m4*x4*sin(e2)*sin(e3)*sin(e4) + 2.0*I6xx*de6*cos(e6)^2*sin(e2)*sin(e3)*sin(e4)*sin(e5) - 2.0*I6yy*de6*cos(e6)^2*sin(e2)*sin(e3)*sin(e4)*sin(e5) - 1.0*de1*m6*x6^2*cos(e2)^2*cos(e5)*cos(e6)*sin(e6) - 1.0*de1*m6*x6^2*cos(e3)^2*cos(e5)*cos(e6)*sin(e6) - 2.0*de1*m6*x6^2*cos(e4)^2*cos(e5)*cos(e6)*sin(e6) - 4.0*de1*m4*x4*y4*cos(e2)^2*cos(e3)^2*cos(e4)^2 + de1*m6*y6^2*cos(e2)^2*cos(e5)*cos(e6)*sin(e6) + de1*m6*y6^2*cos(e3)^2*cos(e5)*cos(e6)*sin(e6) + 2.0*de1*m6*y6^2*cos(e4)^2*cos(e5)*cos(e6)*sin(e6) + de1*m5*x5*y5*cos(e2)*sin(e2)*sin(e4) + de1*m5*x5*y5*cos(e3)*sin(e3)*sin(e4) - 1.0*de1*m4*x4*z4*cos(e2)*sin(e2)*sin(e4) - 1.0*de1*m4*x4*z4*cos(e3)*sin(e3)*sin(e4) - 1.5*de2*m4*y4*z4*cos(e2)*sin(e3)*sin(e4) - 1.5*de2*m4*y4*z4*cos(e3)*sin(e2)*sin(e4) - 1.5*de3*m4*y4*z4*cos(e2)*sin(e3)*sin(e4) - 1.5*de3*m4*y4*z4*cos(e3)*sin(e2)*sin(e4) - 0.5*de4*m4*y4*z4*cos(e4)*sin(e2)*sin(e3) + 2.0*de5*m6*y6*z6*cos(e2)*sin(e3)*sin(e6) + 2.0*de5*m6*y6*z6*cos(e3)*sin(e2)*sin(e6) + 2.0*de5*m5*x5^2*cos(e4)*cos(e5)^2*sin(e2)*sin(e3) - 0.5*de5*m6*x6^2*cos(e4)*cos(e6)^2*sin(e2)*sin(e3) - 2.0*de5*m5*y5^2*cos(e4)*cos(e5)^2*sin(e2)*sin(e3) + 2.0*de5*m6*y6^2*cos(e4)*cos(e5)^2*sin(e2)*sin(e3) + 0.5*de5*m6*y6^2*cos(e4)*cos(e6)^2*sin(e2)*sin(e3) + 0.5*de4*m5*x5*y5*sin(e2)*sin(e3)*sin(e4) - 2.0*de5*m6*z6^2*cos(e4)*cos(e5)^2*sin(e2)*sin(e3) - 0.5*de4*m4*x4*z4*sin(e2)*sin(e3)*sin(e4) + 2.0*I6xx*de5*cos(e2)*cos(e3)*cos(e4)*cos(e5)^2*cos(e6)^2 - 2.0*I6yy*de5*cos(e2)*cos(e3)*cos(e4)*cos(e5)^2*cos(e6)^2 - 1.0*a2*de1*m4*y4*cos(e2)^2*cos(e3)*cos(e4) + a3*de1*m6*y6*cos(e2)^2*cos(e4)*cos(e6) + a3*de1*m6*y6*cos(e3)^2*cos(e4)*cos(e6) + a2*de1*m5*z5*cos(e2)^2*cos(e3)*cos(e4) - 2.0*I6xx*de1*cos(e2)^2*cos(e3)^2*cos(e5)*cos(e6)*sin(e6) - 2.0*I6xx*de1*cos(e2)^2*cos(e4)^2*cos(e5)*cos(e6)*sin(e6) - 2.0*I6xx*de1*cos(e3)^2*cos(e4)^2*cos(e5)*cos(e6)*sin(e6) + 2.0*I6yy*de1*cos(e2)^2*cos(e3)^2*cos(e5)*cos(e6)*sin(e6) + 2.0*I6yy*de1*cos(e2)^2*cos(e4)^2*cos(e5)*cos(e6)*sin(e6) + 2.0*I6yy*de1*cos(e3)^2*cos(e4)^2*cos(e5)*cos(e6)*sin(e6) - 1.0*a2*de1*m4*x4*cos(e2)^2*cos(e3)*sin(e4) + a3*de1*m5*x5*cos(e2)^2*cos(e5)*sin(e4) + a3*de1*m5*x5*cos(e3)^2*cos(e5)*sin(e4) + a3*de1*m6*x6*cos(e2)^2*cos(e4)*sin(e6) + a3*de1*m6*x6*cos(e3)^2*cos(e4)*sin(e6) - 2.0*I6xx*de5*cos(e4)*cos(e5)^2*cos(e6)^2*sin(e2)*sin(e3) + 2.0*I6yy*de5*cos(e4)*cos(e5)^2*cos(e6)^2*sin(e2)*sin(e3) - 1.0*a3*de1*m5*y5*cos(e2)^2*sin(e4)*sin(e5) - 1.0*a3*de1*m5*y5*cos(e3)^2*sin(e4)*sin(e5) - 1.0*a3*de1*m6*z6*cos(e2)^2*sin(e4)*sin(e5) - 1.0*a3*de1*m6*z6*cos(e3)^2*sin(e4)*sin(e5) - 1.0*de2*m5*x5^2*cos(e2)*cos(e3)*cos(e4)^2*cos(e5)^2 - 1.0*de3*m5*x5^2*cos(e2)*cos(e3)*cos(e4)^2*cos(e5)^2 - 1.0*de2*m6*x6^2*cos(e2)*cos(e3)*cos(e4)^2*cos(e6)^2 - 0.5*de2*m6*x6^2*cos(e2)*cos(e3)*cos(e5)^2*cos(e6)^2 - 1.0*de3*m6*x6^2*cos(e2)*cos(e3)*cos(e4)^2*cos(e6)^2 - 0.5*de3*m6*x6^2*cos(e2)*cos(e3)*cos(e5)^2*cos(e6)^2 + de2*m5*y5^2*cos(e2)*cos(e3)*cos(e4)^2*cos(e5)^2 + de3*m5*y5^2*cos(e2)*cos(e3)*cos(e4)^2*cos(e5)^2 - 1.0*de2*m6*y6^2*cos(e2)*cos(e3)*cos(e4)^2*cos(e5)^2 + de2*m6*y6^2*cos(e2)*cos(e3)*cos(e4)^2*cos(e6)^2 - 1.0*de3*m6*y6^2*cos(e2)*cos(e3)*cos(e4)^2*cos(e5)^2 + 0.5*de2*m6*y6^2*cos(e2)*cos(e3)*cos(e5)^2*cos(e6)^2 + de3*m6*y6^2*cos(e2)*cos(e3)*cos(e4)^2*cos(e6)^2 + 0.5*de3*m6*y6^2*cos(e2)*cos(e3)*cos(e5)^2*cos(e6)^2 + 4.0*de5*m5*x5*y5*cos(e2)*cos(e5)^2*sin(e3) + 4.0*de5*m5*x5*y5*cos(e3)*cos(e5)^2*sin(e2) - 2.0*de6*m6*x6*y6*cos(e2)*cos(e5)^2*sin(e3) - 2.0*de6*m6*x6*y6*cos(e3)*cos(e5)^2*sin(e2) - 4.0*de6*m6*x6*y6*cos(e2)*cos(e6)^2*sin(e3) - 4.0*de6*m6*x6*y6*cos(e3)*cos(e6)^2*sin(e2) + de2*m6*z6^2*cos(e2)*cos(e3)*cos(e4)^2*cos(e5)^2 + de3*m6*z6^2*cos(e2)*cos(e3)*cos(e4)^2*cos(e5)^2 + de1*m6*y6*z6*cos(e2)^2*cos(e6)*sin(e5) + de1*m6*y6*z6*cos(e3)^2*cos(e6)*sin(e5) + 2.0*de1*m6*y6*z6*cos(e4)^2*cos(e6)*sin(e5) - 2.0*de1*m4*x4^2*cos(e2)^2*cos(e3)^2*cos(e4)*sin(e4) + de1*m5*x5^2*cos(e2)^2*cos(e4)*cos(e5)^2*sin(e4) + 2.0*de1*m6*x6^2*cos(e2)^2*cos(e3)^2*cos(e4)*sin(e4) + de1*m5*x5^2*cos(e3)^2*cos(e4)*cos(e5)^2*sin(e4) + de1*m6*x6^2*cos(e2)^2*cos(e4)*cos(e6)^2*sin(e4) + de1*m6*x6^2*cos(e3)^2*cos(e4)*cos(e6)^2*sin(e4) - 1.0*de1*m6*x6^2*cos(e4)*cos(e5)^2*cos(e6)^2*sin(e4) + 2.0*de1*m4*y4^2*cos(e2)^2*cos(e3)^2*cos(e4)*sin(e4) - 2.0*de1*m5*y5^2*cos(e2)^2*cos(e3)^2*cos(e4)*sin(e4) - 1.0*de1*m5*y5^2*cos(e2)^2*cos(e4)*cos(e5)^2*sin(e4) - 1.0*de1*m5*y5^2*cos(e3)^2*cos(e4)*cos(e5)^2*sin(e4) + de1*m6*y6^2*cos(e2)^2*cos(e4)*cos(e5)^2*sin(e4) - 1.0*de1*m6*y6^2*cos(e2)^2*cos(e4)*cos(e6)^2*sin(e4) + de1*m6*y6^2*cos(e3)^2*cos(e4)*cos(e5)^2*sin(e4) - 1.0*de1*m6*y6^2*cos(e3)^2*cos(e4)*cos(e6)^2*sin(e4) + de1*m6*y6^2*cos(e4)*cos(e5)^2*cos(e6)^2*sin(e4) + 2.0*de1*m5*z5^2*cos(e2)^2*cos(e3)^2*cos(e4)*sin(e4) - 2.0*de1*m6*z6^2*cos(e2)^2*cos(e3)^2*cos(e4)*sin(e4) - 1.0*de1*m6*z6^2*cos(e2)^2*cos(e4)*cos(e5)^2*sin(e4) - 1.0*de1*m6*z6^2*cos(e3)^2*cos(e4)*cos(e5)^2*sin(e4) + de1*m6*x6*z6*cos(e2)^2*sin(e5)*sin(e6) + de1*m6*x6*z6*cos(e3)^2*sin(e5)*sin(e6) + 2.0*de1*m6*x6*z6*cos(e4)^2*sin(e5)*sin(e6) + 2.0*a3*de1*m5*y5*cos(e2)^2*cos(e3)^2*sin(e4)*sin(e5) + 2.0*a3*de1*m6*z6*cos(e2)^2*cos(e3)^2*sin(e4)*sin(e5) - 1.0*de2*m6*x6^2*cos(e2)*cos(e3)*cos(e4)^2*cos(e5)^2*cos(e6)^2 - 1.0*de3*m6*x6^2*cos(e2)*cos(e3)*cos(e4)^2*cos(e5)^2*cos(e6)^2 + de2*m6*y6^2*cos(e2)*cos(e3)*cos(e4)^2*cos(e5)^2*cos(e6)^2 + de3*m6*y6^2*cos(e2)*cos(e3)*cos(e4)^2*cos(e5)^2*cos(e6)^2 + 1.5*de2*m5*x5^2*cos(e2)*cos(e4)*cos(e5)*sin(e3)*sin(e5) + 1.5*de2*m5*x5^2*cos(e3)*cos(e4)*cos(e5)*sin(e2)*sin(e5) + 1.5*de3*m5*x5^2*cos(e2)*cos(e4)*cos(e5)*sin(e3)*sin(e5) + 1.5*de3*m5*x5^2*cos(e3)*cos(e4)*cos(e5)*sin(e2)*sin(e5) + 0.5*de4*m5*x5^2*cos(e2)*cos(e3)*cos(e5)*sin(e4)*sin(e5) + 4.0*de6*m6*x6*y6*cos(e2)*cos(e5)^2*cos(e6)^2*sin(e3) + 4.0*de6*m6*x6*y6*cos(e3)*cos(e5)^2*cos(e6)^2*sin(e2) - 1.5*de2*m5*y5^2*cos(e2)*cos(e4)*cos(e5)*sin(e3)*sin(e5) - 1.5*de2*m5*y5^2*cos(e3)*cos(e4)*cos(e5)*sin(e2)*sin(e5) - 1.5*de3*m5*y5^2*cos(e2)*cos(e4)*cos(e5)*sin(e3)*sin(e5) - 1.5*de3*m5*y5^2*cos(e3)*cos(e4)*cos(e5)*sin(e2)*sin(e5) + 1.5*de2*m6*y6^2*cos(e2)*cos(e4)*cos(e5)*sin(e3)*sin(e5) + 1.5*de2*m6*y6^2*cos(e3)*cos(e4)*cos(e5)*sin(e2)*sin(e5) - 0.5*de4*m5*y5^2*cos(e2)*cos(e3)*cos(e5)*sin(e4)*sin(e5) + 1.5*de3*m6*y6^2*cos(e2)*cos(e4)*cos(e5)*sin(e3)*sin(e5) + 1.5*de3*m6*y6^2*cos(e3)*cos(e4)*cos(e5)*sin(e2)*sin(e5) + 0.5*de4*m6*y6^2*cos(e2)*cos(e3)*cos(e5)*sin(e4)*sin(e5) - 1.5*de2*m6*z6^2*cos(e2)*cos(e4)*cos(e5)*sin(e3)*sin(e5) - 1.5*de2*m6*z6^2*cos(e3)*cos(e4)*cos(e5)*sin(e2)*sin(e5) - 1.5*de3*m6*z6^2*cos(e2)*cos(e4)*cos(e5)*sin(e3)*sin(e5) - 1.5*de3*m6*z6^2*cos(e3)*cos(e4)*cos(e5)*sin(e2)*sin(e5) - 0.5*de4*m6*z6^2*cos(e2)*cos(e3)*cos(e5)*sin(e4)*sin(e5) - 2.0*de1*m6*y6*z6*cos(e2)^2*cos(e3)^2*cos(e6)*sin(e5) - 2.0*de1*m6*y6*z6*cos(e2)^2*cos(e4)^2*cos(e6)*sin(e5) - 2.0*de1*m6*y6*z6*cos(e3)^2*cos(e4)^2*cos(e6)*sin(e5) - 2.0*de1*m5*x5^2*cos(e2)^2*cos(e3)^2*cos(e4)*cos(e5)^2*sin(e4) - 2.0*de1*m6*x6^2*cos(e2)^2*cos(e3)^2*cos(e4)*cos(e6)^2*sin(e4) + de1*m6*x6^2*cos(e2)^2*cos(e4)*cos(e5)^2*cos(e6)^2*sin(e4) + de1*m6*x6^2*cos(e3)^2*cos(e4)*cos(e5)^2*cos(e6)^2*sin(e4) + 2.0*de1*m5*y5^2*cos(e2)^2*cos(e3)^2*cos(e4)*cos(e5)^2*sin(e4) - 2.0*de1*m6*y6^2*cos(e2)^2*cos(e3)^2*cos(e4)*cos(e5)^2*sin(e4) + 2.0*de1*m6*y6^2*cos(e2)^2*cos(e3)^2*cos(e4)*cos(e6)^2*sin(e4) - 1.0*de1*m6*y6^2*cos(e2)^2*cos(e4)*cos(e5)^2*cos(e6)^2*sin(e4) - 1.0*de1*m6*y6^2*cos(e3)^2*cos(e4)*cos(e5)^2*cos(e6)^2*sin(e4) - 1.0*de1*m5*x5^2*cos(e2)*cos(e5)*sin(e2)*sin(e4)*sin(e5) - 1.0*de1*m5*x5^2*cos(e3)*cos(e5)*sin(e3)*sin(e4)*sin(e5) + 2.0*de1*m6*z6^2*cos(e2)^2*cos(e3)^2*cos(e4)*cos(e5)^2*sin(e4) + de1*m5*y5^2*cos(e2)*cos(e5)*sin(e2)*sin(e4)*sin(e5) + de1*m5*y5^2*cos(e3)*cos(e5)*sin(e3)*sin(e4)*sin(e5) - 1.0*de1*m6*y6^2*cos(e2)*cos(e5)*sin(e2)*sin(e4)*sin(e5) - 1.0*de1*m6*y6^2*cos(e3)*cos(e5)*sin(e3)*sin(e4)*sin(e5) - 2.0*de1*m6*x6*z6*cos(e2)^2*cos(e3)^2*sin(e5)*sin(e6) - 2.0*de1*m6*x6*z6*cos(e2)^2*cos(e4)^2*sin(e5)*sin(e6) - 2.0*de1*m6*x6*z6*cos(e3)^2*cos(e4)^2*sin(e5)*sin(e6) + de1*m6*z6^2*cos(e2)*cos(e5)*sin(e2)*sin(e4)*sin(e5) + de1*m6*z6^2*cos(e3)*cos(e5)*sin(e3)*sin(e4)*sin(e5) - 1.5*a3*de2*m5*x5*cos(e2)*cos(e3)*cos(e4)*cos(e5) - 1.5*a3*de3*m5*x5*cos(e2)*cos(e3)*cos(e4)*cos(e5) - 1.5*a2*de2*m6*x6*cos(e2)*cos(e4)*cos(e5)*cos(e6) + 0.5*d4*de5*m5*y5*cos(e2)*cos(e3)*cos(e4)*cos(e5) + 0.5*d4*de4*m6*y6*cos(e2)*cos(e3)*cos(e4)*cos(e6) + 0.5*d4*de5*m6*z6*cos(e2)*cos(e3)*cos(e4)*cos(e5) + de2*m6*x6^2*cos(e4)^2*cos(e5)^2*cos(e6)^2*sin(e2)*sin(e3) + de3*m6*x6^2*cos(e4)^2*cos(e5)^2*cos(e6)^2*sin(e2)*sin(e3) - 1.0*de2*m6*y6^2*cos(e4)^2*cos(e5)^2*cos(e6)^2*sin(e2)*sin(e3) - 1.0*de3*m6*y6^2*cos(e4)^2*cos(e5)^2*cos(e6)^2*sin(e2)*sin(e3) - 0.5*de4*m5*x5^2*cos(e5)*sin(e2)*sin(e3)*sin(e4)*sin(e5) + 0.5*de4*m5*y5^2*cos(e5)*sin(e2)*sin(e3)*sin(e4)*sin(e5) - 0.5*de4*m6*y6^2*cos(e5)*sin(e2)*sin(e3)*sin(e4)*sin(e5) + 0.5*de4*m6*z6^2*cos(e5)*sin(e2)*sin(e3)*sin(e4)*sin(e5) + a2*de1*m6*x6*cos(e3)*cos(e5)*cos(e6)*sin(e4) + a1*de1*m6*y6*cos(e2)*cos(e4)*cos(e6)*sin(e3) + a1*de1*m6*y6*cos(e3)*cos(e4)*cos(e6)*sin(e2) + 1.5*a3*de2*m5*y5*cos(e2)*cos(e3)*cos(e4)*sin(e5) + 1.5*a3*de3*m5*y5*cos(e2)*cos(e3)*cos(e4)*sin(e5) + 1.5*a3*de2*m6*y6*cos(e2)*cos(e3)*cos(e6)*sin(e4) + 0.5*a3*de5*m5*y5*cos(e2)*cos(e4)*cos(e5)*sin(e3) + 0.5*a3*de5*m5*y5*cos(e3)*cos(e4)*cos(e5)*sin(e2) + 1.5*a2*de2*m6*y6*cos(e2)*cos(e4)*cos(e5)*sin(e6) + 1.5*a3*de3*m6*y6*cos(e2)*cos(e3)*cos(e6)*sin(e4) + 0.5*a3*de4*m6*y6*cos(e2)*cos(e4)*cos(e6)*sin(e3) + 0.5*a3*de4*m6*y6*cos(e3)*cos(e4)*cos(e6)*sin(e2) + 0.5*a2*de6*m6*y6*cos(e4)*cos(e5)*cos(e6)*sin(e2) + 1.5*a3*de2*m6*z6*cos(e2)*cos(e3)*cos(e4)*sin(e5) + 1.5*a3*de3*m6*z6*cos(e2)*cos(e3)*cos(e4)*sin(e5) + 0.5*a3*de5*m6*z6*cos(e2)*cos(e4)*cos(e5)*sin(e3) + 0.5*a3*de5*m6*z6*cos(e3)*cos(e4)*cos(e5)*sin(e2) + 1.5*d4*de2*m5*x5*cos(e2)*cos(e4)*cos(e5)*sin(e3) + 1.5*d4*de2*m5*x5*cos(e3)*cos(e4)*cos(e5)*sin(e2) + 1.5*d4*de3*m5*x5*cos(e2)*cos(e4)*cos(e5)*sin(e3) + 1.5*d4*de3*m5*x5*cos(e3)*cos(e4)*cos(e5)*sin(e2) + 0.5*d4*de4*m5*x5*cos(e2)*cos(e3)*cos(e5)*sin(e4) + 0.5*d4*de5*m5*x5*cos(e2)*cos(e3)*cos(e4)*sin(e5) + 0.5*d4*de4*m6*x6*cos(e2)*cos(e3)*cos(e4)*sin(e6) + 0.5*d4*de6*m6*x6*cos(e2)*cos(e3)*cos(e6)*sin(e4) - 1.5*I6xx*de2*cos(e2)*cos(e4)*cos(e5)*cos(e6)^2*sin(e3)*sin(e5) - 1.5*I6xx*de2*cos(e3)*cos(e4)*cos(e5)*cos(e6)^2*sin(e2)*sin(e5) - 1.5*I6xx*de3*cos(e2)*cos(e4)*cos(e5)*cos(e6)^2*sin(e3)*sin(e5) - 1.5*I6xx*de3*cos(e3)*cos(e4)*cos(e5)*cos(e6)^2*sin(e2)*sin(e5) - 0.5*I6xx*de4*cos(e2)*cos(e3)*cos(e5)*cos(e6)^2*sin(e4)*sin(e5) + 1.5*I6yy*de2*cos(e2)*cos(e4)*cos(e5)*cos(e6)^2*sin(e3)*sin(e5) + 1.5*I6yy*de2*cos(e3)*cos(e4)*cos(e5)*cos(e6)^2*sin(e2)*sin(e5) + 1.5*I6yy*de3*cos(e2)*cos(e4)*cos(e5)*cos(e6)^2*sin(e3)*sin(e5) + 1.5*I6yy*de3*cos(e3)*cos(e4)*cos(e5)*cos(e6)^2*sin(e2)*sin(e5) + 0.5*I6yy*de4*cos(e2)*cos(e3)*cos(e5)*cos(e6)^2*sin(e4)*sin(e5) - 1.0*d4*de1*m6*y6*cos(e2)*cos(e4)*cos(e6)*sin(e2) - 1.0*d4*de1*m6*y6*cos(e3)*cos(e4)*cos(e6)*sin(e3) - 0.5*de4*m5*y5*z5*cos(e2)*cos(e3)*cos(e4)*cos(e5) - 1.5*de6*m6*y6*z6*cos(e2)*cos(e3)*cos(e4)*cos(e6) + a1*de1*m5*x5*cos(e2)*cos(e5)*sin(e3)*sin(e4) + a1*de1*m5*x5*cos(e3)*cos(e5)*sin(e2)*sin(e4) + a1*de1*m6*x6*cos(e2)*cos(e4)*sin(e3)*sin(e6) + a1*de1*m6*x6*cos(e3)*cos(e4)*sin(e2)*sin(e6) + 1.5*a3*de2*m5*x5*cos(e4)*cos(e5)*sin(e2)*sin(e3) + 1.5*a3*de3*m5*x5*cos(e4)*cos(e5)*sin(e2)*sin(e3) + 0.5*a3*de4*m5*x5*cos(e2)*cos(e5)*sin(e3)*sin(e4) + 0.5*a3*de4*m5*x5*cos(e3)*cos(e5)*sin(e2)*sin(e4) + 1.5*a3*de2*m6*x6*cos(e2)*cos(e3)*sin(e4)*sin(e6) + 0.5*a3*de5*m5*x5*cos(e2)*cos(e4)*sin(e3)*sin(e5) + 0.5*a3*de5*m5*x5*cos(e3)*cos(e4)*sin(e2)*sin(e5) + 1.5*a3*de3*m6*x6*cos(e2)*cos(e3)*sin(e4)*sin(e6) + 0.5*a3*de4*m6*x6*cos(e2)*cos(e4)*sin(e3)*sin(e6) + 0.5*a3*de4*m6*x6*cos(e3)*cos(e4)*sin(e2)*sin(e6) + 0.5*a2*de4*m6*x6*cos(e5)*cos(e6)*sin(e2)*sin(e4) + 0.5*a2*de5*m6*x6*cos(e4)*cos(e6)*sin(e2)*sin(e5) + 0.5*a3*de6*m6*x6*cos(e2)*cos(e6)*sin(e3)*sin(e4) + 0.5*a3*de6*m6*x6*cos(e3)*cos(e6)*sin(e2)*sin(e4) + 0.5*a2*de6*m6*x6*cos(e4)*cos(e5)*sin(e2)*sin(e6) + a2*de1*m4*y4*cos(e2)*cos(e4)*sin(e2)*sin(e3) - 1.0*a2*de1*m6*y6*cos(e3)*cos(e5)*sin(e4)*sin(e6) + 2.0*I6xx*de1*cos(e2)^2*cos(e3)^2*cos(e4)*cos(e5)^2*cos(e6)^2*sin(e4) - 2.0*I6yy*de1*cos(e2)^2*cos(e3)^2*cos(e4)*cos(e5)^2*cos(e6)^2*sin(e4) - 1.0*a2*de1*m5*z5*cos(e2)*cos(e4)*sin(e2)*sin(e3) - 1.0*d4*de1*m5*x5*cos(e2)*cos(e5)*sin(e2)*sin(e4) - 1.0*d4*de1*m5*x5*cos(e3)*cos(e5)*sin(e3)*sin(e4) - 1.0*d4*de1*m6*x6*cos(e2)*cos(e4)*sin(e2)*sin(e6) - 1.0*d4*de1*m6*x6*cos(e3)*cos(e4)*sin(e3)*sin(e6) - 2.0*I5xx*de1*cos(e2)*cos(e3)^2*cos(e5)*sin(e2)*sin(e4)*sin(e5);
